simulink model "ACT_ur10"  (R2021b)
settings: Solver=ode4  StartTime=0.0  StopTime=15.0  FixedStep=1e-3  RelTol=1e-3
values from neighbouring files (symbols this model uses):
  Kp = [100 0 0 0 0 0 0 250 0 0 0 0 ... (36 elements, 6x6)]    [ACT_workspace.mat]    (also in GuadagniControllore.m = 100 * diag([1 1 2 4 5 5]))
  Kv = [100 0 0 0 0 0 0 100 0 0 0 0 ... (36 elements, 6x6)]    [ACT_workspace.mat]    (also in GuadagniControllore.m = 100 * diag([1 1 3 3 5 5]))
  l1 = 0.1273    [ACT_workspace.mat]
  l2 = -0.612    [ACT_workspace.mat]
  l3 = -0.5723    [ACT_workspace.mat]
  l4 = 0.1639    [ACT_workspace.mat]
  l5 = 0.1157    [ACT_workspace.mat]
  l6 = 0.0922    [ACT_workspace.mat]
  m1 = 7.1    [ACT_workspace.mat]
  m2 = 12.7    [ACT_workspace.mat]
  m3 = 4.27    [ACT_workspace.mat]
  m4 = 2    [ACT_workspace.mat]
  m5 = 2    [ACT_workspace.mat]
  m6 = 0.365    [ACT_workspace.mat]
  q0 = [0 0 0 0 0 0]    [ACT_workspace.mat]
  r = 0.02    [ACT_workspace.mat]
undefined symbols (not defined in the file or in its folder): B, pi_param, Spline
libraries: roblocks x2, robotcorelib x1, simulink x1
(part 2 of 6)

== matlab function ACT_ur10/CT control1/Dynamics_parametrs/Regressor ==
  data: q input; Y output; qd input; qdd input
function Y = Y(q, qd, qdd)

t1 = q(1);
t2 = q(2);
t3 = q(3);
t4 = q(4);
t5 = q(5);
t6 = q(6);
t1d = qd(1);
t2d = qd(2);
t3d = qd(3);
t4d = qd(4);
t5d = qd(5);
t6d = qd(6);
t1dd = qdd(1);
t2dd = qdd(2);
t3dd = qdd(3);
t4dd = qdd(4);
t5dd = qdd(5);
t6dd = qdd(6);




%#codegen

%    This function was generated by the Symbolic Math Toolbox version 9.0.
%    31-Aug-2022 14:42:02

t8 = cos(t1);
t9 = cos(t2);
t10 = cos(t3);
t11 = cos(t4);
t12 = cos(t5);
t13 = cos(t6);
t14 = sin(t1);
t15 = sin(t2);
t16 = sin(t3);
t17 = sin(t4);
t18 = sin(t5);
t19 = sin(t6);
t20 = t2+t3;
t21 = t1d.^2;
t22 = t2d.^2;
t33 = -t5;
t23 = t8.^2;
t24 = t9.^2;
t25 = t12.^2;
t26 = t14.^2;
t27 = t15.^2;
t28 = t18.^2;
t29 = t18.^3;
t30 = cos(t20);
t31 = sin(t20);
t32 = t4+t20;
t34 = t8.*t12;
t35 = t8.*t18;
t36 = t12.*t14;
t38 = t14.*t18;
t43 = t9.*t15.*t1d;
t45 = t9.*6.12e+3;
t46 = t15.*6.12e+3;
t86 = t9.*(1.53e+2./2.5e+2);
t87 = t8.*(1.53e+2./5.0e+2);
t96 = t15.*(1.53e+2./2.5e+2);
t97 = t14.*(1.53e+2./5.0e+2);
t160 = t8.*t9.*(-1.53e+2./2.5e+2);
t161 = t9.*t14.*(-1.53e+2./2.5e+2);
t167 = t14.*t15.*(-1.53e+2./2.5e+2);
t169 = t8.*1.639e-1;
t170 = t8.*2.8615e-1;
t171 = t14.*1.639e-1;
t172 = t14.*2.8615e-1;
t225 = t9.*6.00372;
t273 = t8.*t15.*t16.*5.723e-1;
t274 = t9.*t14.*t16.*5.723e-1;
t275 = t10.*t14.*t15.*5.723e-1;
t277 = t14.*t15.*t16.*5.723e-1;
t305 = t8.*t9.*t10.*5.723e-1;
t311 = t8.*t9.*t16.*5.723e-1;
t312 = t8.*t10.*t15.*5.723e-1;
t313 = t9.*t10.*t14.*5.723e-1;
t37 = cos(t32);
t39 = sin(t32);
t40 = t5+t32;
t41 = t30.^2;
t42 = t31.^2;
t47 = t8.*t24;
t48 = t9.*t23;
t49 = t8.*t27;
t50 = t9.*t26;
t51 = t15.*t23;
t52 = t14.*t24;
t54 = t14.*t27;
t55 = t15.*t26;
t58 = t43.*t2d.*2.0;
t65 = t32+t33;
t67 = t30.*5.723e+3;
t68 = t31.*5.723e+3;
t69 = t23.*t30;
t71 = t26.*t30;
t72 = t23.*t31;
t76 = t26.*t31;
t82 = t23+t26;
t88 = t30.*t31.*t1d;
t116 = t30.*t31.*t2d.*2.0;
t117 = t30.*t31.*t3d.*2.0;
t124 = t8.*t86;
t126 = t8.*t96;
t127 = t14.*t86;
t134 = t14.*t96;
t208 = t17.*t31.*9.22e-2;
t209 = t30.*5.723e-1;
t212 = t34.*1.383e-1;
t213 = t34.*5.785e-2;
t214 = t31.*5.723e-1;
t216 = t35.*1.383e-1;
t217 = t36.*1.383e-1;
t218 = t35.*5.785e-2;
t219 = t36.*5.785e-2;
t222 = t38.*1.383e-1;
t223 = t38.*5.785e-2;
t236 = t11.*t30.*9.22e-2;
t238 = t17.*t30.*9.22e-2;
t239 = t11.*t31.*9.22e-2;
t244 = -t225;
t271 = t17.*t31.*1.157e-1;
t302 = t11.*t30.*1.157e-1;
t306 = t17.*t30.*1.157e-1;
t307 = t11.*t31.*1.157e-1;
t315 = t14.*t31.*(-5.723e-1);
t316 = -t277;
t335 = -t305;
t338 = t8.*t31.*(-5.723e-1);
t366 = t30.*5.614263;
t396 = t14.*t17.*t30.*(-1.157e-1);
t397 = t8.*t17.*t31.*(-1.157e-1);
t398 = t11.*t14.*t31.*(-1.157e-1);
t399 = t14.*t17.*t31.*(-1.157e-1);
t486 = t87+t161;
t44 = sin(t40);
t53 = t37.^2;
t56 = t39.^2;
t57 = t39.^3;
t59 = t13.*t37;
t60 = t19.*t37;
t61 = t13.*t39;
t62 = t41.*2.0;
t63 = t19.*t39;
t64 = t42.*2.0;
t66 = sin(t65);
t70 = t8.*t41;
t73 = t14.*t41;
t74 = t8.*t42;
t77 = t14.*t42;
t78 = -t42;
t80 = -t49;
t81 = -t54;
t83 = t34.*t37;
t89 = t35.*t37;
t90 = t36.*t37;
t98 = t37.*t38;
t104 = t23.*t37;
t107 = t26.*t37;
t108 = t23.*t39;
t113 = t26.*t39;
t128 = t37.*t39.*t1d;
t141 = t69./2.0;
t145 = t71./2.0;
t146 = t72./2.0;
t147 = t76./2.0;
t152 = t37.*t39.*2.0;
t173 = t12.*t37.*t39;
t174 = t18.*t37.*t39;
t197 = t23.*t82;
t198 = t26.*t82;
t204 = t30.*t82;
t205 = t31.*t82;
t226 = t48+t50;
t227 = t37.*t82;
t229 = t51+t55;
t230 = t39.*t82;
t241 = -t209;
t251 = t37.*1.157e-1;
t252 = t37.*8.195e-2;
t253 = t39.*1.157e-1;
t254 = t39.*8.195e-2;
t259 = -t236;
t272 = t14.*t214;
t285 = t18.*t37.*4.61e-2;
t286 = t12.*t39.*4.61e-2;
t294 = t18.*t39.*4.61e-2;
t298 = t45+t67;
t299 = t46+t68;
t308 = t8.*t214;
t314 = -t271;
t324 = t18.*t37.*5.785e-2;
t327 = t18.*t39.*5.785e-2;
t336 = -t306;
t337 = -t307;
t343 = t72+t76;
t346 = t72.*5.723e-1;
t347 = t76.*5.723e-1;
t349 = t14.*t39.*(-8.195e-2);
t350 = t8.*t302;
t351 = t8.*t306;
t352 = t14.*t302;
t353 = t8.*t307;
t357 = t14.*t306;
t358 = t8.*t271;
t359 = t14.*t307;
t362 = t14.*t271;
t365 = t69+t71;
t380 = t39.*t216;
t382 = t39.*t218;
t388 = t39.*t222;
t389 = t39.*t223;
t404 = -t366;
t419 = t39.*1.135017;
t420 = t39.*8.039295e-1;
t454 = t97+t124;
t460 = t116+t117;
t529 = t86+t209;
t530 = t96+t214;
t554 = t14.*t486;
t622 = t238+t239;
t707 = t9.*t87.*t486;
t708 = t126.*t486;
t75 = t53.*t1dd;
t79 = -t64;
t84 = t8.*t59;
t85 = t12.*t59;
t91 = t8.*t60;
t92 = t14.*t59;
t93 = t8.*t61;
t94 = t12.*t60;
t95 = t12.*t61;
t99 = t14.*t60;
t100 = t8.*t63;
t101 = t14.*t61;
t102 = t12.*t63;
t103 = t14.*t63;
t105 = t8.*t53;
t106 = t12.*t53;
t109 = t14.*t53;
t110 = t8.*t56;
t111 = t18.*t53;
t112 = t12.*t56;
t114 = t14.*t56;
t115 = t18.*t56;
t118 = -t74;
t119 = -t77;
t125 = t34.*t61;
t129 = t34.*t63;
t130 = t36.*t61;
t131 = t23.*t56;
t132 = t25.*t57;
t135 = t36.*t63;
t136 = t26.*t56;
t137 = t28.*t56;
t138 = t28.*t57;
t139 = -t89;
t140 = -t90;
t148 = t34.*t56;
t149 = t35.*t56;
t150 = t36.*t56;
t151 = t12.*t18.*t57;
t153 = t38.*t56;
t163 = t152.*t2d;
t164 = t152.*t3d;
t165 = t152.*t4d;
t166 = t25.*t56.*2.0;
t178 = -t152;
t179 = t104./2.0;
t180 = t107./2.0;
t181 = t108./2.0;
t182 = t113./2.0;
t188 = t39.*t53.*3.0;
t228 = t204.*t1dd;
t231 = t205.*t1dd;
t232 = t18.*t39.*t59;
t233 = t18.*t39.*t60;
t242 = t39.*t53.*(3.0./2.0);
t245 = t25.*t128;
t246 = t39.*t83.*3.0;
t247 = t28.*t128;
t248 = t39.*t89.*3.0;
t249 = t39.*t90.*3.0;
t250 = t39.*t98.*3.0;
t255 = t34+t98;
t256 = t38+t83;
t257 = t227.*t1dd;
t258 = t230.*t1dd;
t260 = t41+t78;
t261 = t39.*t104.*2.0;
t264 = -t204;
t265 = t39.*t107.*2.0;
t266 = t28.*t152;
t269 = -t205;
t278 = t53.*t108;
t279 = t25.*t39.*t53;
t280 = t47+t80;
t281 = t53.*t113;
t283 = t28.*t39.*t53;
t284 = -t227;
t290 = t52+t81;
t291 = -t230;
t295 = -t251;
t296 = -t253;
t297 = -t254;
t301 = t12.*t18.*t128.*2.0;
t321 = t29.*t37.*t56.*3.0;
t322 = t8.*t252;
t323 = -t285;
t325 = t14.*t252;
t326 = t8.*t254;
t328 = t14.*t254;
t348 = -t324;
t355 = (t204.*t1d.*t2d)./2.0;
t356 = (t204.*t1d.*t3d)./2.0;
t360 = (t205.*t1d.*t2d)./2.0;
t361 = (t205.*t1d.*t3d)./2.0;
t369 = t83.*1.383e-1;
t370 = t83.*5.785e-2;
t371 = t89.*1.383e-1;
t372 = t90.*1.383e-1;
t373 = t89.*5.785e-2;
t374 = t90.*5.785e-2;
t376 = (t227.*t1d.*t2d)./2.0;
t377 = (t227.*t1d.*t3d)./2.0;
t378 = (t227.*t1d.*t4d)./2.0;
t379 = t98.*1.383e-1;
t381 = t98.*5.785e-2;
t384 = t29.*t37.*t56.*(3.0./2.0);
t385 = (t230.*t1d.*t2d)./2.0;
t386 = (t230.*t1d.*t3d)./2.0;
t387 = (t230.*t1d.*t4d)./2.0;
t392 = t104.*8.195e-2;
t393 = t107.*8.195e-2;
t421 = t365.*t2d;
t422 = t365.*t3d;
t425 = t104+t107;
t426 = t343.*t2d;
t427 = t343.*t3d;
t431 = t108+t113;
t432 = t44.*6.783615e-1;
t433 = t44.*2.8375425e-1;
t492 = t66.*6.783615e-1;
t493 = t66.*2.8375425e-1;
t497 = t460.*t1d;
t532 = t8.*t454;
t534 = (t14.*t299)./1.0e+4;
t550 = (t8.*t298)./1.0e+4;
t551 = (t14.*t298)./1.0e+4;
t553 = (t8.*t299)./1.0e+4;
t562 = t530.^2;
t583 = t197+t198;
t584 = (t23.*t299)./1.0e+4;
t586 = (t26.*t299)./1.0e+4;
t599 = -t554;
t638 = t208+t259;
t647 = t214+t252;
t648 = t39.*t104.*3.35790125e-3;
t649 = t39.*t104.*1.007370375e-2;
t652 = t39.*t107.*3.35790125e-3;
t653 = t39.*t107.*1.007370375e-2;
t670 = t241+t254;
t677 = t12.*t622;
t678 = t18.*t622;
t687 = t251+t327;
t692 = t9.*t97.*t454;
t693 = t134.*t454;
t742 = t346+t347;
t820 = t252+t530;
t896 = t69.*t530.*2.8615e-1;
t897 = t76.*t529.*2.8615e-1;
t899 = t346.*t530;
t900 = t71.*t530.*2.8615e-1;
t907 = t347.*t530;
t932 = t72.*t529.*2.8615e-1;
t1287 = t350+t380+t397;
t1288 = t350+t382+t397;
t1297 = t352+t388+t399;
t1298 = t352+t389+t399;
t1453 = t169+t313+t316+t349;
t120 = t106.*2.0;
t121 = t111.*2.0;
t122 = t112.*2.0;
t123 = t115.*2.0;
t133 = -t85;
t142 = -t100;
t143 = -t101;
t144 = -t102;
t154 = -t110;
t155 = -t112;
t157 = -t114;
t158 = -t115;
t162 = t18.*t112.*t1d;
t168 = t137.*2.0;
t175 = t137.*t1dd;
t177 = t151.*2.0;
t183 = t28.*t110;
t184 = t26.*t112;
t185 = t23.*t115;
t186 = t25.*t114;
t187 = t13.*t137;
t189 = t28.*t114;
t190 = t26.*t115;
t191 = t19.*t137;
t193 = -t129;
t194 = -t135;
t196 = -t138;
t199 = -t148;
t200 = t18.*t112.*-2.0;
t201 = -t151;
t203 = -t153;
t206 = t25.*t110;
t207 = t23.*t112;
t211 = -t188;
t221 = t132./2.0;
t224 = t138./2.0;
t237 = t37.*t112;
t240 = t37.*t115;
t276 = -t242;
t282 = t37.*t137;
t287 = t28.*t163;
t288 = t28.*t164;
t289 = t28.*t165;
t292 = -t248;
t293 = -t249;
t317 = t255.^2;
t318 = t62+t79;
t319 = t279.*2.0;
t320 = t283.*2.0;
t329 = t35+t140;
t330 = t36+t139;
t333 = t18.*t39.*t106.*4.0;
t334 = -t257;
t339 = t14.*t256;
t340 = t19.*t256;
t341 = t60+t95;
t342 = t61+t94;
t344 = -t279;
t363 = t8.*t255;
t364 = t13.*t256;
t367 = t21.*t260;
t375 = t53.*t181;
t383 = t53.*t182;
t390 = t14.*t280;
t391 = t8.*t290;
t394 = -t355;
t395 = -t356;
t405 = t73+t119;
t406 = -t371;
t407 = -t372;
t408 = -t373;
t409 = -t374;
t410 = -t376;
t411 = -t377;
t412 = -t378;
t414 = -t385;
t415 = -t386;
t416 = -t387;
t430 = t70+t118;
t435 = t37.*t255;
t436 = t37.*t256;
t437 = t39.*t255;
t438 = t39.*t256;
t439 = t148.*5.785e-2;
t441 = t150.*5.785e-2;
t442 = -t432;
t443 = -t433;
t450 = t425.*t2d;
t451 = t425.*t3d;
t452 = t425.*t4d;
t453 = t91+t125;
t456 = t431.*t2d;
t457 = t431.*t3d;
t458 = t431.*t4d;
t459 = t99+t130;
t505 = t101.*t255;
t512 = t103.*t255;
t535 = t18.*t61.*t255.*2.0;
t537 = t18.*t63.*t255.*2.0;
t555 = -t534;
t568 = t153.*t255;
t571 = -t551;
t572 = -t553;
t617 = t583.*t2dd;
t618 = t583.*t3dd;
t619 = t583.*t4dd;
t637 = t53+t131+t136;
t675 = t647.^2;
t688 = t18.*t638;
t697 = t255.*t380;
t703 = t253+t348;
t704 = t212+t379;
t705 = t222+t369;
t706 = t223+t370;
t720 = t687.^2;
t777 = t163+t164+t165;
t787 = t146+t147+t269;
t793 = t172+t550;
t795 = t167+t534;
t798 = t141+t145+t264;
t799 = t392+t393;
t842 = t426+t427;
t843 = t297+t529;
t855 = t8.*t37.*t687;
t858 = t14.*t37.*t687;
t859 = t8.*t39.*t687;
t860 = t14.*t39.*t687;
t865 = t421+t422;
t876 = t179+t180+t284;
t878 = t181+t182+t291;
t880 = t820.^2;
t881 = -t8.*(t553-t8.*t15.*(1.53e+2./2.5e+2));
t951 = t178+t261+t265;
t1036 = t214+t687;
t1055 = t209+t296+t324;
t1082 = t286+t677;
t1089 = t392.*t647;
t1092 = t393.*t647;
t1093 = t108.*t647.*8.195e-2;
t1094 = t108.*t647.*4.0975e-2;
t1097 = t113.*t647.*8.195e-2;
t1098 = t113.*t647.*4.0975e-2;
t1121 = t311+t312+t322;
t1122 = t392.*t670;
Y = ft_1({t100,t101,t103,t1036,t104,t105,t1055,t106,t107,t108,t1082,t1089,t109,t1092,t1093,t1094,t1097,t1098,t111,t112,t1121,t1122,t113,t115,t12,t120,t121,t122,t123,t124,t126,t127,t128,t1287,t1288,t1297,t1298,t13,t131,t132,t133,t134,t136,t137,t138,t14,t140,t142,t143,t144,t1453,t148,t149,t15,t150,t152,t153,t154,t155,t157,t158,t160,t162,t163,t164,t165,t166,t168,t169,t170,t171,t172,t173,t174,t175,t177,t179,t18,t180,t183,t184,t185,t186,t187,t189,t19,t190,t191,t193,t194,t196,t199,t1d,t1dd,t200,t201,t203,t206,t207,t209,t21,t211,t213,t214,t216,t217,t218,t219,t22,t221,t224,t226,t228,t229,t23,t231,t232,t233,t237,t24,t240,t241,t244,t245,t246,t247,t248,t249,t25,t250,t255,t256,t258,t26,t261,t265,t266,t27,t272,t273,t274,t275,t276,t278,t279,t28,t281,t282,t283,t285,t287,t288,t289,t29,t292,t293,t294,t295,t296,t299,t2d,t2dd,t30,t301,t302,t306,t307,t308,t31,t311,t312,t313,t314,t315,t316,t317,t318,t319,t320,t321,t322,t323,t324,t325,t326,t328,t329,t330,t333,t334,t335,t336,t337,t338,t339,t34,t340,t341,t342,t343,t344,t346,t347,t35,t351,t353,t36,t360,t361,t363,t364,t365,t367,t37,t375,t38,t381,t383,t384,t388,t39,t390,t391,t392,t393,t394,t395,t396,t398,t3d,t3dd,t404,t405,t406,t407,t408,t409,t41,t410,t411,t412,t414,t415,t416,t419,t42,t420,t425,t43,t430,t431,t435,t436,t437,t438,t439,t441,t442,t443,t450,t451,t452,t453,t454,t456,t457,t458,t459,t48,t486,t492,t493,t497,t4d,t4dd,t50,t51,t512,t529,t53,t530,t532,t535,t537,t55,t550,t553,t554,t555,t56,t562,t57,t571,t572,t58,t584,t586,t59,t599,t5d,t5dd,t61,t617,t618,t619,t63,t637,t647,t648,t649,t652,t653,t670,t675,t678,t687,t688,t69,t692,t693,t697,t6d,t6dd,t703,t704,t705,t706,t707,t708,t71,t720,t742,t75,t777,t787,t793,t795,t798,t799,t8,t82,t820,t83,t84,t842,t843,t855,t858,t859,t860,t865,t876,t878,t88,t880,t881,t89,t896,t897,t899,t9,t90,t900,t907,t92,t93,t932,t951,t98});
end
function Y = ft_1(ct)
t100 = ct{1};
t101 = ct{2};
t103 = ct{3};
t1036 = ct{4};
t104 = ct{5};
t105 = ct{6};
t1055 = ct{7};
t106 = ct{8};
t107 = ct{9};
t108 = ct{10};
t1082 = ct{11};
t1089 = ct{12};
t109 = ct{13};
t1092 = ct{14};
t1093 = ct{15};
t1094 = ct{16};
t1097 = ct{17};
t1098 = ct{18};
t111 = ct{19};
t112 = ct{20};
t1121 = ct{21};
t1122 = ct{22};
t113 = ct{23};
t115 = ct{24};
t12 = ct{25};
t120 = ct{26};
t121 = ct{27};
t122 = ct{28};
t123 = ct{29};
t124 = ct{30};
t126 = ct{31};
t127 = ct{32};
t128 = ct{33};
t1287 = ct{34};
t1288 = ct{35};
t1297 = ct{36};
t1298 = ct{37};
t13 = ct{38};
t131 = ct{39};
t132 = ct{40};
t133 = ct{41};
t134 = ct{42};
t136 = ct{43};
t137 = ct{44};
t138 = ct{45};
t14 = ct{46};
t140 = ct{47};
t142 = ct{48};
t143 = ct{49};
t144 = ct{50};
t1453 = ct{51};
t148 = ct{52};
t149 = ct{53};
t15 = ct{54};
t150 = ct{55};
t152 = ct{56};
t153 = ct{57};
t154 = ct{58};
t155 = ct{59};
t157 = ct{60};
t158 = ct{61};
t160 = ct{62};
t162 = ct{63};
t163 = ct{64};
t164 = ct{65};
t165 = ct{66};
t166 = ct{67};
t168 = ct{68};
t169 = ct{69};
t170 = ct{70};
t171 = ct{71};
t172 = ct{72};
t173 = ct{73};
t174 = ct{74};
t175 = ct{75};
t177 = ct{76};
t179 = ct{77};
t18 = ct{78};
t180 = ct{79};
t183 = ct{80};
t184 = ct{81};
t185 = ct{82};
t186 = ct{83};
t187 = ct{84};
t189 = ct{85};
t19 = ct{86};
t190 = ct{87};
t191 = ct{88};
t193 = ct{89};
t194 = ct{90};
t196 = ct{91};
t199 = ct{92};
t1d = ct{93};
t1dd = ct{94};
t200 = ct{95};
t201 = ct{96};
t203 = ct{97};
t206 = ct{98};
t207 = ct{99};
t209 = ct{100};
t21 = ct{101};
t211 = ct{102};
t213 = ct{103};
t214 = ct{104};
t216 = ct{105};
t217 = ct{106};
t218 = ct{107};
t219 = ct{108};
t22 = ct{109};
t221 = ct{110};
t224 = ct{111};
t226 = ct{112};
t228 = ct{113};
t229 = ct{114};
t23 = ct{115};
t231 = ct{116};
t232 = ct{117};
t233 = ct{118};
t237 = ct{119};
t24 = ct{120};
t240 = ct{121};
t241 = ct{122};
t244 = ct{123};
t245 = ct{124};
t246 = ct{125};
t247 = ct{126};
t248 = ct{127};
t249 = ct{128};
t25 = ct{129};
t250 = ct{130};
t255 = ct{131};
t256 = ct{132};
t258 = ct{133};
t26 = ct{134};
t261 = ct{135};
t265 = ct{136};
t266 = ct{137};
t27 = ct{138};
t272 = ct{139};
t273 = ct{140};
t274 = ct{141};
t275 = ct{142};
t276 = ct{143};
t278 = ct{144};
t279 = ct{145};
t28 = ct{146};
t281 = ct{147};
t282 = ct{148};
t283 = ct{149};
t285 = ct{150};
t287 = ct{151};
t288 = ct{152};
t289 = ct{153};
t29 = ct{154};
t292 = ct{155};
t293 = ct{156};
t294 = ct{157};
t295 = ct{158};
t296 = ct{159};
t299 = ct{160};
t2d = ct{161};
t2dd = ct{162};
t30 = ct{163};
t301 = ct{164};
t302 = ct{165};
t306 = ct{166};
t307 = ct{167};
t308 = ct{168};
t31 = ct{169};
t311 = ct{170};
t312 = ct{171};
t313 = ct{172};
t314 = ct{173};
t315 = ct{174};
t316 = ct{175};
t317 = ct{176};
t318 = ct{177};
t319 = ct{178};
t320 = ct{179};
t321 = ct{180};
t322 = ct{181};
t323 = ct{182};
t324 = ct{183};
t325 = ct{184};
t326 = ct{185};
t328 = ct{186};
t329 = ct{187};
t330 = ct{188};
t333 = ct{189};
t334 = ct{190};
t335 = ct{191};
t336 = ct{192};
t337 = ct{193};
t338 = ct{194};
t339 = ct{195};
t34 = ct{196};
t340 = ct{197};
t341 = ct{198};
t342 = ct{199};
t343 = ct{200};
t344 = ct{201};
t346 = ct{202};
t347 = ct{203};
t35 = ct{204};
t351 = ct{205};
t353 = ct{206};
t36 = ct{207};
t360 = ct{208};
t361 = ct{209};
t363 = ct{210};
t364 = ct{211};
t365 = ct{212};
t367 = ct{213};
t37 = ct{214};
t375 = ct{215};
t38 = ct{216};
t381 = ct{217};
t383 = ct{218};
t384 = ct{219};
t388 = ct{220};
t39 = ct{221};
t390 = ct{222};
t391 = ct{223};
t392 = ct{224};
t393 = ct{225};
t394 = ct{226};
t395 = ct{227};
t396 = ct{228};
t398 = ct{229};
t3d = ct{230};
t3dd = ct{231};
t404 = ct{232};
t405 = ct{233};
t406 = ct{234};
t407 = ct{235};
t408 = ct{236};
t409 = ct{237};
t41 = ct{238};
t410 = ct{239};
t411 = ct{240};
t412 = ct{241};
t414 = ct{242};
t415 = ct{243};
t416 = ct{244};
t419 = ct{245};
t42 = ct{246};
t420 = ct{247};
t425 = ct{248};
t43 = ct{249};
t430 = ct{250};
t431 = ct{251};
t435 = ct{252};
t436 = ct{253};
t437 = ct{254};
t438 = ct{255};
t439 = ct{256};
t441 = ct{257};
t442 = ct{258};
t443 = ct{259};
t450 = ct{260};
t451 = ct{261};
t452 = ct{262};
t453 = ct{263};
t454 = ct{264};
t456 = ct{265};
t457 = ct{266};
t458 = ct{267};
t459 = ct{268};
t48 = ct{269};
t486 = ct{270};
t492 = ct{271};
t493 = ct{272};
t497 = ct{273};
t4d = ct{274};
t4dd = ct{275};
t50 = ct{276};
t51 = ct{277};
t512 = ct{278};
t529 = ct{279};
t53 = ct{280};
t530 = ct{281};
t532 = ct{282};
t535 = ct{283};
t537 = ct{284};
t55 = ct{285};
t550 = ct{286};
t553 = ct{287};
t554 = ct{288};
t555 = ct{289};
t56 = ct{290};
t562 = ct{291};
t57 = ct{292};
t571 = ct{293};
t572 = ct{294};
t58 = ct{295};
t584 = ct{296};
t586 = ct{297};
t59 = ct{298};
t599 = ct{299};
t5d = ct{300};
t5dd = ct{301};
t61 = ct{302};
t617 = ct{303};
t618 = ct{304};
t619 = ct{305};
t63 = ct{306};
t637 = ct{307};
t647 = ct{308};
t648 = ct{309};
t649 = ct{310};
t652 = ct{311};
t653 = ct{312};
t670 = ct{313};
t675 = ct{314};
t678 = ct{315};
t687 = ct{316};
t688 = ct{317};
t69 = ct{318};
t692 = ct{319};
t693 = ct{320};
t697 = ct{321};
t6d = ct{322};
t6dd = ct{323};
t703 = ct{324};
t704 = ct{325};
t705 = ct{326};
t706 = ct{327};
t707 = ct{328};
t708 = ct{329};
t71 = ct{330};
t720 = ct{331};
t742 = ct{332};
t75 = ct{333};
t777 = ct{334};
t787 = ct{335};
t793 = ct{336};
t795 = ct{337};
t798 = ct{338};
t799 = ct{339};
t8 = ct{340};
t82 = ct{341};
t820 = ct{342};
t83 = ct{343};
t84 = ct{344};
t842 = ct{345};
t843 = ct{346};
t855 = ct{347};
t858 = ct{348};
t859 = ct{349};
t860 = ct{350};
t865 = ct{351};
t876 = ct{352};
t878 = ct{353};
t88 = ct{354};
t880 = ct{355};
t881 = ct{356};
t89 = ct{357};
t896 = ct{358};
t897 = ct{359};
t899 = ct{360};
t9 = ct{361};
t90 = ct{362};
t900 = ct{363};
t907 = ct{364};
t92 = ct{365};
t93 = ct{366};
t932 = ct{367};
t951 = ct{368};
t98 = ct{369};
t1123 = t104.*t670.*4.0975e-2;
t1133 = t393.*t670;
t1134 = t107.*t670.*4.0975e-2;
t1140 = t274+t275+t325;
t1203 = t532+t599;
t1222 = t12.*t113.*t687.*2.8925e-2;
t1245 = t12.*t108.*t687.*5.785e-2;
t1246 = t12.*t108.*t687.*2.8925e-2;
t1248 = t12.*t113.*t687.*5.785e-2;
t1265 = t584+t586;
t1302 = t530+t687;
t1321 = t296+t324+t529;
t1330 = t393.*t820;
t1331 = t108.*t820.*8.195e-2;
t1332 = t108.*t820.*4.0975e-2;
t1334 = t113.*t820.*8.195e-2;
t1335 = t113.*t820.*4.0975e-2;
t1352 = t392.*t820;
t1364 = t8.*t1287;
t1365 = t8.*t1288;
t1372 = t14.*t1297;
t1373 = t14.*t1298;
t1426 = t37.*t1287;
t1427 = t37.*t1288;
t1431 = t37.*t1297;
t1432 = t37.*t1298;
t1450 = t171+t273+t326+t335;
t1462 = t14.*t39.*t1287;
t1463 = t14.*t39.*t1288;
t1466 = t8.*t39.*t1297;
t1467 = t8.*t39.*t1298;
t1510 = t14.*t1453;
t1519 = t693+t708;
t1534 = t692+t707;
t1596 = t213+t381+t396+t398;
t1666 = t23.*t647.*t820;
t1669 = t26.*t647.*t820;
t1677 = t127+t1453;
t1754 = (t23.*t670.*t820)./2.0;
t1758 = (t26.*t670.*t820)./2.0;
t1807 = t294+t302+t314+t678;
t1961 = t311+t312+t1287;
t1962 = t311+t312+t1288;
t1976 = t274+t275+t1297;
t1977 = t274+t275+t1298;
t2106 = (t14.*t687.*t1288)./2.0;
t2109 = (t8.*t687.*t1298)./2.0;
t156 = -t122;
t159 = -t123;
t176 = t18.*t122;
t195 = -t168;
t202 = -t177;
t210 = t13.*t168;
t215 = t19.*t168;
t220 = t18.*t155.*t1d;
t234 = t34.*t123;
t235 = t36.*t123;
t243 = -t224;
t262 = t37.*t122;
t263 = t39.*t120;
t267 = t37.*t123;
t268 = t39.*t121;
t270 = t25.*t154;
t300 = t18.*t237;
t303 = t37.*t155;
t304 = t237.*-2.0;
t309 = t37.*t158;
t310 = t240.*-2.0;
t345 = -t319;
t368 = t330.^2;
t400 = t14.*t330;
t401 = t19.*t329;
t402 = t59+t144;
t403 = t63+t133;
t413 = t13.*t317;
t417 = t19.*t317;
t418 = t341.^2;
t423 = t13.*t363;
t424 = t19.*t363;
t428 = t8.*t329;
t429 = t13.*t329;
t434 = -t367;
t440 = -t391;
t447 = t390./2.0;
t448 = t391./2.0;
t449 = -t441;
t462 = t105+t154;
t463 = t106+t155;
t465 = t109+t157;
t466 = t111+t158;
t467 = t183.*1.383e-1;
t468 = t8.*t436;
t469 = t12.*t435;
t470 = t12.*t436;
t471 = t189.*1.383e-1;
t472 = t14.*t435;
t473 = t8.*t438;
t474 = t18.*t435;
t475 = t18.*t436;
t476 = t12.*t437;
t477 = t14.*t437;
t478 = t18.*t438;
t479 = t14.*t430;
t480 = t37.*t329;
t481 = t37.*t330;
t482 = t8.*t405;
t483 = t39.*t329;
t484 = t39.*t330;
t490 = t12.*t438.*2.0;
t491 = t18.*t437.*2.0;
t494 = t37.*t341;
t495 = t37.*t342;
t496 = t39.*t341;
t499 = t84+t193;
t502 = t92+t194;
t503 = t35.*t437;
t504 = t36.*t438;
t506 = t8.*t459;
t533 = t14.*t453;
t536 = t38.*t437.*2.0;
t545 = t18.*t39.*t342;
t556 = t100.*t330;
t557 = t143.*t255;
t561 = -t512;
t574 = t93.*t330;
t578 = t18.*t61.*t330.*2.0;
t579 = t18.*t63.*t330.*2.0;
t597 = t115.*t341;
t602 = t18.*t63.*t341.*2.0;
t603 = t149.*t330;
t606 = t203.*t255;
t609 = t93+t340;
t610 = t189.*t255;
t611 = t123.*t341;
t614 = t83.*t438;
t615 = t8.*t39.*t453;
t616 = t18.*t39.*t453;
t620 = t98.*t437;
t623 = t14.*t39.*t459;
t624 = t18.*t39.*t459;
t634 = t158.*t341;
t636 = t168.*t341;
t640 = t142+t364;
t642 = t183.*t330;
t644 = t28.*t157.*t255;
t664 = t18.*t152.*t341;
t695 = -t14.*(t100-t364);
t696 = t266.*t341;
t698 = t255.*t341;
t699 = t256.*t341;
t700 = t255.*t342;
t709 = t255.*t329.*2.0;
t710 = t256.*t330.*2.0;
t715 = t199+t436;
t718 = t203+t435;
t719 = -t688;
t721 = t216+t407;
t722 = t217+t406;
t723 = t218+t409;
t731 = t330.*t388;
t732 = t329.*t341;
t733 = t330.*t341;
t734 = t330.*t342;
t738 = t39.*t637;
t741 = t246+t438;
t743 = t250+t437;
t744 = t341.*t342;
t745 = t8.*t705;
t746 = t8.*t706;
t749 = -t8.*t39.*(t100-t364);
t750 = -t18.*t37.*(t100-t364);
t751 = -t12.*t39.*(t100-t364);
t758 = -t18.*t39.*(t100-t364);
t768 = -t14.*(t148-t436);
t769 = -t8.*(t153-t435);
t771 = t8.*t37.*t637;
t772 = t12.*t37.*t637;
t773 = t14.*t37.*t637;
t774 = t18.*t37.*t637;
t779 = t255.*t459;
t782 = -t8.*t37.*(t100-t364);
t791 = t126+t572;
t802 = t8.*t39.*(t100-t364);
t811 = t18.*t39.*(t100-t364);
t818 = t37.*t705;
t819 = t37.*t706;
t824 = t170+t571;
t828 = t777.*t1d;
t830 = t330.*t453;
t836 = -t35.*t39.*(t100-t364);
t837 = -t18.*t61.*(t100-t364);
t840 = -t18.*t63.*(t100-t364);
t841 = t341.*t453;
t844 = t341.*t459;
t849 = t14.*(t148-t436).*(-1.0./2.0);
t850 = t8.*(t153-t435).*(-1.0./2.0);
t856 = t798.*t2d;
t857 = t798.*t3d;
t862 = t787.*t2d;
t863 = t787.*t3d;
t869 = t18.*t37.*t704;
t870 = t12.*t39.*t704;
t872 = t14.*t39.*t705;
t873 = t18.*t39.*t704;
t874 = t18.*t39.*t705;
t875 = t14.*t39.*t706;
t884 = t8.*t793;
t885 = t8.*t39.*t703;
t886 = t14.*t39.*t703;
t890 = t14.*t795;
t892 = t35.*t39.*(t100-t364);
t893 = t18.*t61.*(t100-t364);
t918 = -t8.*t37.*(t148-t436);
t920 = -t8.*t39.*(t148-t436);
t921 = -t855;
t924 = -t858;
t925 = -t859;
t926 = -t14.*t37.*(t153-t435);
t929 = -t14.*t39.*(t153-t435);
t933 = t35.*t39.*t704;
t934 = t876.*t2d;
t935 = t876.*t3d;
t936 = t876.*t4d;
t940 = t878.*t2d;
t941 = t878.*t3d;
t942 = t878.*t4d;
t963 = t8.*t37.*(t148-t436);
t966 = t8.*t39.*(t148-t436);
t970 = t14.*t37.*(t153-t435);
t973 = t14.*t39.*(t153-t435);
t1002 = t255.*t637;
t1003 = t256.*t637;
t1016 = -t256.*(t100-t364);
t1051 = t329.*t637;
t1052 = t330.*t637;
t1065 = -t330.*(t100-t364);
t1066 = t256.*(t100-t364);
t1075 = -t342.*(t100-t364);
t1085 = t37.*t951;
t1096 = t1036.^2;
t1104 = t341.*(t100-t364).*-2.0;
t1135 = -t1094;
t1139 = -t1098;
t1141 = t255.*t705;
t1142 = t256.*t704;
t1163 = t8.*t39.*t951;
t1164 = t12.*t39.*t951;
t1165 = t14.*t39.*t951;
t1166 = t18.*t39.*t951;
t1169 = t160+t793;
t1172 = -t1123;
t1174 = -t1134;
t1194 = t330.*t704;
t1200 = t14.*t1140;
t1215 = t8.*t1121;
t1256 = t14.*t209.*t793;
t1257 = t30.*t172.*t793;
t1258 = t272.*t793;
t1299 = t8.*t39.*t1082;
t1303 = t14.*t39.*t1082;
t1333 = t1302.^2;
t1355 = -t1332;
t1358 = -t1335;
t1368 = t617+t618;
t1375 = t104.*t843.*4.0975e-2;
t1378 = t107.*t843.*4.0975e-2;
t1380 = t255.*t951;
t1381 = t256.*t951;
t1410 = t126+t1121;
t1413 = t134+t1140;
t1414 = t329.*t951;
t1415 = t330.*t951;
t1470 = t255.*t1082;
t1481 = t8.*t1450;
t1485 = t450+t451+t452;
t1488 = t14.*t530.*t793;
t1492 = t456+t457+t458;
t1494 = -t1466;
t1495 = -t1467;
t1498 = t325.*t1121;
t1499 = t14.*t37.*t1121.*4.0975e-2;
t1500 = t322.*t1140;
t1501 = t8.*t37.*t1140.*4.0975e-2;
t1506 = t330.*t1082;
t1512 = t338+t1121;
t1515 = t315+t1140;
t1516 = t14.*t37.*t1121.*(-8.195e-2);
t1517 = t12.*t108.*t1036.*5.785e-2;
t1518 = t12.*t108.*t1036.*2.8925e-2;
t1520 = t12.*t113.*t1036.*5.785e-2;
t1521 = t12.*t113.*t1036.*2.8925e-2;
t1540 = -t1510;
t1541 = (t14.*t529.*t793)./2.0;
t1547 = t14.*t687.*t706;
t1576 = t219+t351+t353+t408;
t1595 = t396+t398+t704;
t1650 = (t23.*t687.*t703)./2.0;
t1651 = t23.*t687.*t703.*(3.0./2.0);
t1652 = (t26.*t687.*t703)./2.0;
t1653 = t26.*t687.*t703.*(3.0./2.0);
t1674 = t160+t1450;
t1709 = t12.*t108.*t1302.*5.785e-2;
t1710 = t12.*t108.*t1302.*2.8925e-2;
t1713 = t12.*t113.*t1302.*5.785e-2;
t1714 = t12.*t113.*t1302.*2.8925e-2;
t1729 = t37.*t1596;
t1731 = t39.*t1596;
t1745 = t14.*t1677;
t1751 = (t23.*t647.*t843)./2.0;
t1755 = (t26.*t647.*t843)./2.0;
t1818 = t306+t307+t323+t688;
t1837 = t14.*t706.*t1036;
t1840 = t1807.^2;
t1863 = t23.*t687.*t1036;
t1868 = t26.*t687.*t1036;
t1888 = t23.*t687.*t1055;
t1889 = t23.*t703.*t1036;
t1890 = t26.*t687.*t1055;
t1891 = t26.*t703.*t1036;
t1906 = (t14.*t647.*t1121)./2.0;
t1910 = (t8.*t647.*t1140)./2.0;
t2003 = t8.*t37.*t1807;
t2006 = t14.*t37.*t1807;
t2007 = t8.*t39.*t1807;
t2008 = t14.*t39.*t1807;
t2034 = t8.*t1961;
t2035 = t8.*t1962;
t2040 = t14.*t1976;
t2041 = t14.*t1977;
t2043 = t14.*t820.*t1121;
t2044 = t8.*t820.*t1140;
t2051 = t322.*t1677;
t2055 = t326.*t1677;
t2056 = t8.*t39.*t1677.*4.0975e-2;
t2070 = t14.*t706.*t1302;
t2081 = t23.*t687.*t1302;
t2087 = t26.*t687.*t1302;
t2100 = t23.*t703.*t1302;
t2101 = t26.*t703.*t1302;
t2113 = t214+t1807;
t2118 = -t2106;
t2141 = (t23.*t687.*t1321)./2.0;
t2142 = (t26.*t687.*t1321)./2.0;
t2148 = t295+t1807;
t2167 = t126+t1961;
t2168 = t126+t1962;
t2173 = t134+t1976;
t2174 = t134+t1977;
t2201 = t571+t1677;
t2272 = t338+t1961;
t2273 = t338+t1962;
t2276 = t315+t1976;
t2277 = t315+t1977;
t2279 = t530+t1807;
t2286 = t8.*t1036.*t1298;
t2309 = t14.*t1036.*t1288;
t2338 = t8.*t647.*t1677;
t2340 = t23.*t1036.*t1302;
t2344 = t26.*t1036.*t1302;
t2354 = t8.*t670.*t1677;
t2398 = (t23.*t1036.*t1321)./2.0;
t2399 = (t23.*t1055.*t1302)./2.0;
t2400 = (t26.*t1036.*t1321)./2.0;
t2401 = (t26.*t1055.*t1302)./2.0;
t2465 = t14.*t1288.*t1302;
t2467 = t8.*t1298.*t1302;
t2483 = t169+t313+t316+t1596;
t2496 = t8.*t820.*t1677;
t2509 = t14.*t705.*t1807;
t2529 = t1364+t1372;
t2530 = t1365+t1373;
t2565 = (t8.*t843.*t1677)./2.0;
t2606 = t8.*t687.*t1977;
t2618 = t14.*t687.*t1962;
t2743 = t23.*t1082.*t1807;
t2744 = t26.*t1082.*t1807;
t2831 = (t8.*t1036.*t1977)./2.0;
t2839 = (t14.*t1036.*t1962)./2.0;
t2896 = (t14.*t1287.*t1807)./2.0;
t2897 = (t8.*t1297.*t1807)./2.0;
t2956 = t14.*t1302.*t1962;
t2960 = t8.*t1302.*t1977;
t3307 = t14.*t1807.*t1961;
t3308 = t8.*t1807.*t1976;
t192 = t176.*t5d;
t331 = t37.*t176;
t332 = t18.*t263;
t354 = t18.*t303;
t444 = t13.*t368;
t445 = t19.*t368;
t446 = t402.^2;
t455 = t418.*2.0;
t461 = t13.*t400;
t464 = t19.*t400;
t485 = -t448;
t487 = t120+t156;
t488 = t121+t159;
t489 = -t471;
t498 = t463.*t1d;
t501 = t466.*t1d;
t507 = t8.*t481;
t508 = -t468;
t509 = t12.*t480;
t510 = t12.*t481;
t511 = -t469;
t513 = t14.*t480;
t514 = t8.*t484;
t515 = -t472;
t516 = -t473;
t517 = t18.*t480;
t518 = t18.*t481;
t519 = t12.*t484;
t520 = -t474;
t521 = -t475;
t522 = t14.*t462;
t523 = t14.*t483;
t524 = -t477;
t525 = t18.*t483;
t526 = -t478;
t527 = t8.*t465;
t528 = -t482;
t538 = t12.*t483.*2.0;
t539 = t18.*t484.*2.0;
t540 = t479./2.0;
t541 = t482./2.0;
t542 = t18.*t494;
t543 = t12.*t496;
t544 = t18.*t496;
t546 = t37.*t402;
t547 = t37.*t403;
t548 = t39.*t402;
t552 = t39.*t418;
t558 = t8.*t502;
t559 = t38.*t484;
t560 = -t536;
t569 = t545.*2.0;
t570 = t166+t195;
t573 = t34.*t483;
t575 = t14.*t499;
t576 = -t533;
t577 = t35.*t484.*2.0;
t582 = t35.*t496;
t585 = t38.*t496;
t592 = t18.*t39.*t403;
t594 = -t545;
t596 = t18.*t37.*t418;
t621 = t8.*t39.*t462;
t628 = -t602;
t629 = t14.*t39.*t465;
t633 = t115.*t402;
t635 = t597.*-2.0;
t639 = t18.*t61.*t402.*2.0;
t641 = t103+t429;
t645 = t123.*t402;
t650 = t8.*t39.*t499;
t651 = -t615;
t654 = t89.*t484;
t655 = t90.*t483;
t656 = t18.*t39.*t499;
t657 = -t616;
t658 = -t620;
t659 = t14.*t39.*t502;
t660 = -t623;
t661 = t18.*t39.*t502;
t666 = t610./2.0;
t667 = t158.*t402;
t669 = t14.*t609;
t671 = t614./2.0;
t672 = t620./2.0;
t673 = t168.*t402;
t679 = t143+t401;
t682 = t28.*t39.*t494;
t684 = t140.*t483;
t689 = t18.*t152.*t402;
t690 = t642./2.0;
t716 = t150+t480;
t717 = t149+t481;
t724 = -t8.*(t101-t401);
t725 = t266.*t402;
t726 = t8.*t39.*t609;
t727 = t18.*t37.*t609;
t728 = t12.*t39.*t609;
t729 = t19.*t698;
t730 = t18.*t39.*t609;
t735 = t255.*t402;
t736 = t256.*t402;
t737 = t255.*t403;
t739 = t8.*t37.*t609;
t740 = t13.*t698;
t747 = t14.*t721;
t748 = t14.*t723;
t752 = t19.*t733;
t759 = t329.*t402;
t760 = t330.*t402;
t761 = t330.*t403;
t762 = -t734;
t766 = t744.*2.0;
t775 = t12.*t738;
t776 = t18.*t738;
t778 = -t738;
Y = ft_2({t100,t1002,t1003,t101,t1016,t1036,t104,t1051,t1052,t1055,t106,t1065,t1066,t107,t1075,t108,t1082,t1085,t1089,t1092,t1093,t1094,t1096,t1097,t1098,t1104,t111,t112,t1121,t1122,t1123,t113,t1133,t1134,t1135,t1139,t1140,t1141,t1142,t115,t1163,t1164,t1165,t1166,t1169,t1172,t1174,t1194,t12,t1200,t1203,t1215,t1222,t124,t1245,t1246,t1248,t1256,t1257,t1258,t1265,t127,t128,t1287,t1288,t1297,t1298,t1299,t13,t1302,t1303,t131,t132,t1321,t1330,t1331,t1332,t1333,t1334,t1335,t134,t1352,t1355,t1358,t136,t1368,t137,t1375,t1378,t138,t1380,t1381,t14,t1410,t1413,t1414,t1415,t1426,t1427,t1431,t1432,t1462,t1463,t1470,t1481,t1485,t1488,t1492,t1494,t1495,t1499,t15,t150,t1500,t1501,t1506,t1512,t1515,t1516,t1517,t1518,t1519,t152,t1520,t1521,t1534,t1540,t1541,t1547,t155,t156,t1576,t158,t159,t1595,t160,t162,t163,t164,t165,t1650,t1651,t1652,t1653,t1666,t1669,t1674,t1677,t169,t170,t1709,t171,t1710,t1713,t1714,t1729,t173,t1731,t174,t1745,t175,t1751,t1754,t1755,t1758,t177,t179,t18,t180,t1807,t1818,t183,t1837,t184,t1840,t185,t186,t1863,t1868,t187,t1888,t1889,t189,t1890,t1891,t19,t190,t1906,t191,t1910,t192,t196,t1961,t1962,t1976,t1977,t199,t1d,t1dd,t200,t2003,t2006,t2007,t2008,t201,t202,t2034,t2035,t2040,t2041,t2043,t2044,t2051,t2055,t2056,t206,t207,t2070,t2081,t2087,t209,t21,t210,t2100,t2101,t2109,t211,t2113,t2118,t213,t2141,t2142,t2148,t215,t2167,t2168,t2173,t2174,t219,t22,t220,t2201,t221,t226,t2272,t2273,t2276,t2277,t2279,t228,t2286,t229,t23,t2309,t231,t232,t233,t2338,t234,t2340,t2344,t235,t2354,t2398,t2399,t24,t2400,t2401,t241,t243,t244,t245,t2465,t2467,t247,t248,t2483,t249,t2496,t25,t2509,t2529,t2530,t255,t256,t2565,t258,t26,t2606,t261,t2618,t263,t265,t266,t268,t27,t270,t273,t2743,t2744,t276,t278,t279,t28,t281,t282,t283,t2831,t2839,t285,t287,t288,t289,t2896,t2897,t29,t292,t293,t2956,t296,t2960,t299,t2d,t2dd,t30,t301,t303,t304,t308,t309,t31,t310,t313,t315,t316,t317,t318,t319,t320,t321,t322,t325,t328,t329,t330,t3307,t3308,t331,t332,t333,t334,t335,t336,t337,t339,t34,t341,t342,t343,t344,t345,t346,t347,t35,t351,t353,t354,t36,t360,t361,t363,t364,t365,t368,t37,t375,t38,t383,t384,t39,t390,t392,t393,t394,t395,t3d,t3dd,t400,t401,t402,t403,t404,t41,t410,t411,t412,t413,t414,t415,t416,t417,t418,t419,t42,t420,t423,t424,t425,t428,t43,t431,t434,t437,t439,t440,t441,t442,t443,t444,t445,t446,t447,t449,t453,t454,t455,t459,t461,t463,t464,t466,t467,t468,t470,t472,t473,t476,t477,t478,t479,t48,t483,t484,t485,t486,t487,t488,t489,t490,t491,t492,t493,t494,t495,t496,t497,t498,t499,t4d,t4dd,t50,t501,t502,t503,t504,t506,t507,t508,t509,t51,t510,t511,t513,t514,t515,t516,t517,t518,t519,t520,t521,t522,t523,t524,t525,t526,t527,t528,t529,t53,t530,t532,t535,t536,t537,t538,t539,t540,t541,t542,t543,t544,t545,t546,t547,t548,t55,t550,t552,t553,t554,t555,t556,t557,t558,t559,t56,t560,t561,t562,t569,t57,t570,t571,t573,t574,t575,t576,t577,t578,t579,t58,t582,t585,t592,t594,t596,t5d,t5dd,t602,t603,t606,t609,t61,t614,t615,t616,t617,t619,t621,t623,t624,t628,t629,t63,t633,t634,t635,t636,t637,t639,t641,t642,t644,t645,t647,t648,t649,t650,t651,t652,t653,t654,t655,t656,t657,t658,t659,t660,t661,t664,t666,t667,t669,t670,t671,t672,t673,t675,t682,t684,t687,t689,t69,t690,t695,t696,t697,t698,t699,t6d,t6dd,t700,t703,t705,t706,t709,t71,t710,t716,t717,t719,t720,t721,t722,t723,t724,t725,t726,t727,t728,t729,t730,t731,t732,t733,t735,t736,t737,t738,t739,t740,t741,t742,t743,t744,t745,t746,t747,t748,t749,t75,t750,t751,t752,t759,t760,t761,t762,t766,t768,t769,t771,t772,t773,t774,t775,t776,t778,t779,t782,t791,t793,t799,t8,t802,t811,t818,t819,t82,t820,t824,t828,t830,t836,t840,t841,t842,t843,t844,t849,t850,t855,t856,t857,t859,t860,t862,t863,t865,t869,t870,t872,t873,t874,t875,t88,t880,t881,t884,t885,t886,t890,t892,t893,t896,t897,t899,t9,t900,t907,t921,t924,t925,t932,t933,t934,t935,t936,t940,t941,t942,t963,t966,t970,t973});
end
function Y = ft_2(ct)
t100 = ct{1};
t1002 = ct{2};
t1003 = ct{3};
t101 = ct{4};
t1016 = ct{5};
t1036 = ct{6};
t104 = ct{7};
t1051 = ct{8};
t1052 = ct{9};
t1055 = ct{10};
t106 = ct{11};
t1065 = ct{12};
t1066 = ct{13};
t107 = ct{14};
t1075 = ct{15};
t108 = ct{16};
t1082 = ct{17};
t1085 = ct{18};
t1089 = ct{19};
t1092 = ct{20};
t1093 = ct{21};
t1094 = ct{22};
t1096 = ct{23};
t1097 = ct{24};
t1098 = ct{25};
t1104 = ct{26};
t111 = ct{27};
t112 = ct{28};
t1121 = ct{29};
t1122 = ct{30};
t1123 = ct{31};
t113 = ct{32};
t1133 = ct{33};
t1134 = ct{34};
t1135 = ct{35};
t1139 = ct{36};
t1140 = ct{37};
t1141 = ct{38};
t1142 = ct{39};
t115 = ct{40};
t1163 = ct{41};
t1164 = ct{42};
t1165 = ct{43};
t1166 = ct{44};
t1169 = ct{45};
t1172 = ct{46};
t1174 = ct{47};
t1194 = ct{48};
t12 = ct{49};
t1200 = ct{50};
t1203 = ct{51};
t1215 = ct{52};
t1222 = ct{53};
t124 = ct{54};
t1245 = ct{55};
t1246 = ct{56};
t1248 = ct{57};
t1256 = ct{58};
t1257 = ct{59};
t1258 = ct{60};
t1265 = ct{61};
t127 = ct{62};
t128 = ct{63};
t1287 = ct{64};
t1288 = ct{65};
t1297 = ct{66};
t1298 = ct{67};
t1299 = ct{68};
t13 = ct{69};
t1302 = ct{70};
t1303 = ct{71};
t131 = ct{72};
t132 = ct{73};
t1321 = ct{74};
t1330 = ct{75};
t1331 = ct{76};
t1332 = ct{77};
t1333 = ct{78};
t1334 = ct{79};
t1335 = ct{80};
t134 = ct{81};
t1352 = ct{82};
t1355 = ct{83};
t1358 = ct{84};
t136 = ct{85};
t1368 = ct{86};
t137 = ct{87};
t1375 = ct{88};
t1378 = ct{89};
t138 = ct{90};
t1380 = ct{91};
t1381 = ct{92};
t14 = ct{93};
t1410 = ct{94};
t1413 = ct{95};
t1414 = ct{96};
t1415 = ct{97};
t1426 = ct{98};
t1427 = ct{99};
t1431 = ct{100};
t1432 = ct{101};
t1462 = ct{102};
t1463 = ct{103};
t1470 = ct{104};
t1481 = ct{105};
t1485 = ct{106};
t1488 = ct{107};
t1492 = ct{108};
t1494 = ct{109};
t1495 = ct{110};
t1499 = ct{111};
t15 = ct{112};
t150 = ct{113};
t1500 = ct{114};
t1501 = ct{115};
t1506 = ct{116};
t1512 = ct{117};
t1515 = ct{118};
t1516 = ct{119};
t1517 = ct{120};
t1518 = ct{121};
t1519 = ct{122};
t152 = ct{123};
t1520 = ct{124};
t1521 = ct{125};
t1534 = ct{126};
t1540 = ct{127};
t1541 = ct{128};
t1547 = ct{129};
t155 = ct{130};
t156 = ct{131};
t1576 = ct{132};
t158 = ct{133};
t159 = ct{134};
t1595 = ct{135};
t160 = ct{136};
t162 = ct{137};
t163 = ct{138};
t164 = ct{139};
t165 = ct{140};
t1650 = ct{141};
t1651 = ct{142};
t1652 = ct{143};
t1653 = ct{144};
t1666 = ct{145};
t1669 = ct{146};
t1674 = ct{147};
t1677 = ct{148};
t169 = ct{149};
t170 = ct{150};
t1709 = ct{151};
t171 = ct{152};
t1710 = ct{153};
t1713 = ct{154};
t1714 = ct{155};
t1729 = ct{156};
t173 = ct{157};
t1731 = ct{158};
t174 = ct{159};
t1745 = ct{160};
t175 = ct{161};
t1751 = ct{162};
t1754 = ct{163};
t1755 = ct{164};
t1758 = ct{165};
t177 = ct{166};
t179 = ct{167};
t18 = ct{168};
t180 = ct{169};
t1807 = ct{170};
t1818 = ct{171};
t183 = ct{172};
t1837 = ct{173};
t184 = ct{174};
t1840 = ct{175};
t185 = ct{176};
t186 = ct{177};
t1863 = ct{178};
t1868 = ct{179};
t187 = ct{180};
t1888 = ct{181};
t1889 = ct{182};
t189 = ct{183};
t1890 = ct{184};
t1891 = ct{185};
t19 = ct{186};
t190 = ct{187};
t1906 = ct{188};
t191 = ct{189};
t1910 = ct{190};
t192 = ct{191};
t196 = ct{192};
t1961 = ct{193};
t1962 = ct{194};
t1976 = ct{195};
t1977 = ct{196};
t199 = ct{197};
t1d = ct{198};
t1dd = ct{199};
t200 = ct{200};
t2003 = ct{201};
t2006 = ct{202};
t2007 = ct{203};
t2008 = ct{204};
t201 = ct{205};
t202 = ct{206};
t2034 = ct{207};
t2035 = ct{208};
t2040 = ct{209};
t2041 = ct{210};
t2043 = ct{211};
t2044 = ct{212};
t2051 = ct{213};
t2055 = ct{214};
t2056 = ct{215};
t206 = ct{216};
t207 = ct{217};
t2070 = ct{218};
t2081 = ct{219};
t2087 = ct{220};
t209 = ct{221};
t21 = ct{222};
t210 = ct{223};
t2100 = ct{224};
t2101 = ct{225};
t2109 = ct{226};
t211 = ct{227};
t2113 = ct{228};
t2118 = ct{229};
t213 = ct{230};
t2141 = ct{231};
t2142 = ct{232};
t2148 = ct{233};
t215 = ct{234};
t2167 = ct{235};
t2168 = ct{236};
t2173 = ct{237};
t2174 = ct{238};
t219 = ct{239};
t22 = ct{240};
t220 = ct{241};
t2201 = ct{242};
t221 = ct{243};
t226 = ct{244};
t2272 = ct{245};
t2273 = ct{246};
t2276 = ct{247};
t2277 = ct{248};
t2279 = ct{249};
t228 = ct{250};
t2286 = ct{251};
t229 = ct{252};
t23 = ct{253};
t2309 = ct{254};
t231 = ct{255};
t232 = ct{256};
t233 = ct{257};
t2338 = ct{258};
t234 = ct{259};
t2340 = ct{260};
t2344 = ct{261};
t235 = ct{262};
t2354 = ct{263};
t2398 = ct{264};
t2399 = ct{265};
t24 = ct{266};
t2400 = ct{267};
t2401 = ct{268};
t241 = ct{269};
t243 = ct{270};
t244 = ct{271};
t245 = ct{272};
t2465 = ct{273};
t2467 = ct{274};
t247 = ct{275};
t248 = ct{276};
t2483 = ct{277};
t249 = ct{278};
t2496 = ct{279};
t25 = ct{280};
t2509 = ct{281};
t2529 = ct{282};
t2530 = ct{283};
t255 = ct{284};
t256 = ct{285};
t2565 = ct{286};
t258 = ct{287};
t26 = ct{288};
t2606 = ct{289};
t261 = ct{290};
t2618 = ct{291};
t263 = ct{292};
t265 = ct{293};
t266 = ct{294};
t268 = ct{295};
t27 = ct{296};
t270 = ct{297};
t273 = ct{298};
t2743 = ct{299};
t2744 = ct{300};
t276 = ct{301};
t278 = ct{302};
t279 = ct{303};
t28 = ct{304};
t281 = ct{305};
t282 = ct{306};
t283 = ct{307};
t2831 = ct{308};
t2839 = ct{309};
t285 = ct{310};
t287 = ct{311};
t288 = ct{312};
t289 = ct{313};
t2896 = ct{314};
t2897 = ct{315};
t29 = ct{316};
t292 = ct{317};
t293 = ct{318};
t2956 = ct{319};
t296 = ct{320};
t2960 = ct{321};
t299 = ct{322};
t2d = ct{323};
t2dd = ct{324};
t30 = ct{325};
t301 = ct{326};
t303 = ct{327};
t304 = ct{328};
t308 = ct{329};
t309 = ct{330};
t31 = ct{331};
t310 = ct{332};
t313 = ct{333};
t315 = ct{334};
t316 = ct{335};
t317 = ct{336};
t318 = ct{337};
t319 = ct{338};
t320 = ct{339};
t321 = ct{340};
t322 = ct{341};
t325 = ct{342};
t328 = ct{343};
t329 = ct{344};
t330 = ct{345};
t3307 = ct{346};
t3308 = ct{347};
t331 = ct{348};
t332 = ct{349};
t333 = ct{350};
t334 = ct{351};
t335 = ct{352};
t336 = ct{353};
t337 = ct{354};
t339 = ct{355};
t34 = ct{356};
t341 = ct{357};
t342 = ct{358};
t343 = ct{359};
t344 = ct{360};
t345 = ct{361};
t346 = ct{362};
t347 = ct{363};
t35 = ct{364};
t351 = ct{365};
t353 = ct{366};
t354 = ct{367};
t36 = ct{368};
t360 = ct{369};
t361 = ct{370};
t363 = ct{371};
t364 = ct{372};
t365 = ct{373};
t368 = ct{374};
t37 = ct{375};
t375 = ct{376};
t38 = ct{377};
t383 = ct{378};
t384 = ct{379};
t39 = ct{380};
t390 = ct{381};
t392 = ct{382};
t393 = ct{383};
t394 = ct{384};
t395 = ct{385};
t3d = ct{386};
t3dd = ct{387};
t400 = ct{388};
t401 = ct{389};
t402 = ct{390};
t403 = ct{391};
t404 = ct{392};
t41 = ct{393};
t410 = ct{394};
t411 = ct{395};
t412 = ct{396};
t413 = ct{397};
t414 = ct{398};
t415 = ct{399};
t416 = ct{400};
t417 = ct{401};
t418 = ct{402};
t419 = ct{403};
t42 = ct{404};
t420 = ct{405};
t423 = ct{406};
t424 = ct{407};
t425 = ct{408};
t428 = ct{409};
t43 = ct{410};
t431 = ct{411};
t434 = ct{412};
t437 = ct{413};
t439 = ct{414};
t440 = ct{415};
t441 = ct{416};
t442 = ct{417};
t443 = ct{418};
t444 = ct{419};
t445 = ct{420};
t446 = ct{421};
t447 = ct{422};
t449 = ct{423};
t453 = ct{424};
t454 = ct{425};
t455 = ct{426};
t459 = ct{427};
t461 = ct{428};
t463 = ct{429};
t464 = ct{430};
t466 = ct{431};
t467 = ct{432};
t468 = ct{433};
t470 = ct{434};
t472 = ct{435};
t473 = ct{436};
t476 = ct{437};
t477 = ct{438};
t478 = ct{439};
t479 = ct{440};
t48 = ct{441};
t483 = ct{442};
t484 = ct{443};
t485 = ct{444};
t486 = ct{445};
t487 = ct{446};
t488 = ct{447};
t489 = ct{448};
t490 = ct{449};
t491 = ct{450};
t492 = ct{451};
t493 = ct{452};
t494 = ct{453};
t495 = ct{454};
t496 = ct{455};
t497 = ct{456};
t498 = ct{457};
t499 = ct{458};
t4d = ct{459};
t4dd = ct{460};
t50 = ct{461};
t501 = ct{462};
t502 = ct{463};
t503 = ct{464};
t504 = ct{465};
t506 = ct{466};
t507 = ct{467};
t508 = ct{468};
t509 = ct{469};
t51 = ct{470};
t510 = ct{471};
t511 = ct{472};
t513 = ct{473};
t514 = ct{474};
t515 = ct{475};
t516 = ct{476};
t517 = ct{477};
t518 = ct{478};
t519 = ct{479};
t520 = ct{480};
t521 = ct{481};
t522 = ct{482};
t523 = ct{483};
t524 = ct{484};
t525 = ct{485};
t526 = ct{486};
t527 = ct{487};
t528 = ct{488};
t529 = ct{489};
t53 = ct{490};
t530 = ct{491};
t532 = ct{492};
t535 = ct{493};
t536 = ct{494};
t537 = ct{495};
t538 = ct{496};
t539 = ct{497};
t540 = ct{498};
t541 = ct{499};
t542 = ct{500};
t543 = ct{501};
t544 = ct{502};
t545 = ct{503};
t546 = ct{504};
t547 = ct{505};
t548 = ct{506};
t55 = ct{507};
t550 = ct{508};
t552 = ct{509};
t553 = ct{510};
t554 = ct{511};
t555 = ct{512};
t556 = ct{513};
t557 = ct{514};
t558 = ct{515};
t559 = ct{516};
t56 = ct{517};
t560 = ct{518};
t561 = ct{519};
t562 = ct{520};
t569 = ct{521};
t57 = ct{522};
t570 = ct{523};
t571 = ct{524};
t573 = ct{525};
t574 = ct{526};
t575 = ct{527};
t576 = ct{528};
t577 = ct{529};
t578 = ct{530};
t579 = ct{531};
t58 = ct{532};
t582 = ct{533};
t585 = ct{534};
t592 = ct{535};
t594 = ct{536};
t596 = ct{537};
t5d = ct{538};
t5dd = ct{539};
t602 = ct{540};
t603 = ct{541};
t606 = ct{542};
t609 = ct{543};
t61 = ct{544};
t614 = ct{545};
t615 = ct{546};
t616 = ct{547};
t617 = ct{548};
t619 = ct{549};
t621 = ct{550};
t623 = ct{551};
t624 = ct{552};
t628 = ct{553};
t629 = ct{554};
t63 = ct{555};
t633 = ct{556};
t634 = ct{557};
t635 = ct{558};
t636 = ct{559};
t637 = ct{560};
t639 = ct{561};
t641 = ct{562};
t642 = ct{563};
t644 = ct{564};
t645 = ct{565};
t647 = ct{566};
t648 = ct{567};
t649 = ct{568};
t650 = ct{569};
t651 = ct{570};
t652 = ct{571};
t653 = ct{572};
t654 = ct{573};
t655 = ct{574};
t656 = ct{575};
t657 = ct{576};
t658 = ct{577};
t659 = ct{578};
t660 = ct{579};
t661 = ct{580};
t664 = ct{581};
t666 = ct{582};
t667 = ct{583};
t669 = ct{584};
t670 = ct{585};
t671 = ct{586};
t672 = ct{587};
t673 = ct{588};
t675 = ct{589};
t682 = ct{590};
t684 = ct{591};
t687 = ct{592};
t689 = ct{593};
t69 = ct{594};
t690 = ct{595};
t695 = ct{596};
t696 = ct{597};
t697 = ct{598};
t698 = ct{599};
t699 = ct{600};
t6d = ct{601};
t6dd = ct{602};
t700 = ct{603};
t703 = ct{604};
t705 = ct{605};
t706 = ct{606};
t709 = ct{607};
t71 = ct{608};
t710 = ct{609};
t716 = ct{610};
t717 = ct{611};
t719 = ct{612};
t720 = ct{613};
t721 = ct{614};
t722 = ct{615};
t723 = ct{616};
t724 = ct{617};
t725 = ct{618};
t726 = ct{619};
t727 = ct{620};
t728 = ct{621};
t729 = ct{622};
t730 = ct{623};
t731 = ct{624};
t732 = ct{625};
t733 = ct{626};
t735 = ct{627};
t736 = ct{628};
t737 = ct{629};
t738 = ct{630};
t739 = ct{631};
t740 = ct{632};
t741 = ct{633};
t742 = ct{634};
t743 = ct{635};
t744 = ct{636};
t745 = ct{637};
t746 = ct{638};
t747 = ct{639};
t748 = ct{640};
t749 = ct{641};
t75 = ct{642};
t750 = ct{643};
t751 = ct{644};
t752 = ct{645};
t759 = ct{646};
t760 = ct{647};
t761 = ct{648};
t762 = ct{649};
t766 = ct{650};
t768 = ct{651};
t769 = ct{652};
t771 = ct{653};
t772 = ct{654};
t773 = ct{655};
t774 = ct{656};
t775 = ct{657};
t776 = ct{658};
t778 = ct{659};
t779 = ct{660};
t782 = ct{661};
t791 = ct{662};
t793 = ct{663};
t799 = ct{664};
t8 = ct{665};
t802 = ct{666};
t811 = ct{667};
t818 = ct{668};
t819 = ct{669};
t82 = ct{670};
t820 = ct{671};
t824 = ct{672};
t828 = ct{673};
t830 = ct{674};
t836 = ct{675};
t840 = ct{676};
t841 = ct{677};
t842 = ct{678};
t843 = ct{679};
t844 = ct{680};
t849 = ct{681};
t850 = ct{682};
t855 = ct{683};
t856 = ct{684};
t857 = ct{685};
t859 = ct{686};
t860 = ct{687};
t862 = ct{688};
t863 = ct{689};
t865 = ct{690};
t869 = ct{691};
t870 = ct{692};
t872 = ct{693};
t873 = ct{694};
t874 = ct{695};
t875 = ct{696};
t88 = ct{697};
t880 = ct{698};
t881 = ct{699};
t884 = ct{700};
t885 = ct{701};
t886 = ct{702};
t890 = ct{703};
t892 = ct{704};
t893 = ct{705};
t896 = ct{706};
t897 = ct{707};
t899 = ct{708};
t9 = ct{709};
t900 = ct{710};
t907 = ct{711};
t921 = ct{712};
t924 = ct{713};
t925 = ct{714};
t932 = ct{715};
t933 = ct{716};
t934 = ct{717};
t935 = ct{718};
t936 = ct{719};
t940 = ct{720};
t941 = ct{721};
t942 = ct{722};
t963 = ct{723};
t966 = ct{724};
t970 = ct{725};
t973 = ct{726};
t780 = t35.*t39.*t609;
t781 = t18.*t61.*t609;
t784 = t13.*t733;
t786 = t18.*t63.*t609;
t788 = t339+t428;
t789 = t363+t400;
t790 = t270+t470;
t797 = t738./2.0;
t800 = -t745;
t801 = -t746;
t807 = -t14.*t37.*(t101-t401);
t809 = -t18.*t37.*(t101-t401);
t810 = -t12.*t39.*(t101-t401);
t812 = t293+t483;
t813 = t292+t484;
t815 = -t14.*t39.*(t101-t401);
t816 = -t18.*t39.*(t101-t401);
t821 = t14.*t741;
t822 = t8.*t743;
t823 = t34.*t738;
t825 = t35.*t738;
t826 = t36.*t738;
t827 = t38.*t738;
t831 = t341.*t402.*t1d;
t832 = t341.*t403.*t1d;
t833 = t342.*t402.*t1d;
t834 = t255.*t502;
t835 = -t779;
t845 = t37.*t721;
t846 = t37.*t723;
t847 = t402.*t403;
t852 = t772./2.0;
t853 = t390+t440;
t854 = t774./2.0;
t861 = t341.*t402.*t6d.*2.0;
t864 = t37.*t738;
t866 = -t38.*t39.*(t101-t401);
t867 = -t18.*t63.*(t101-t401);
t868 = t18.*t37.*(t101-t401);
t871 = t14.*t39.*(t101-t401);
t879 = -t828;
t883 = -t14.*(t206-t470);
t887 = t330.*t499;
t894 = -t18.*t61.*(t101-t401);
t901 = t341.*t499;
t902 = t402.*t453;
t903 = t8.*t39.*t721;
t904 = t18.*t37.*t722;
t905 = t12.*t39.*t722;
t906 = t8.*t39.*t723;
t909 = t18.*t39.*t721;
t910 = t18.*t39.*t722;
t911 = t341.*t502;
t912 = t402.*t459;
t913 = -t844;
t914 = -t8.*(t249-t483);
t916 = -t14.*(t248-t484);
t928 = t14.*t824;
t937 = t38.*t39.*(t101-t401);
t938 = -t870;
t939 = -t873;
t943 = t402.*t494;
t944 = t403.*t494;
t945 = t402.*t495;
t946 = t402.*t496;
t948 = -t890;
t952 = t402.*t499;
t953 = t38.*t39.*t722;
t954 = t104.*t738;
t956 = t107.*t738;
t958 = t402.*t502;
t959 = t8.*t39.*t741;
t965 = t14.*t39.*t743;
t968 = t14.*(t206-t470).*(-1.0./2.0);
t969 = t256.*t609;
t981 = -t933;
t984 = t8.*(t249-t483).*(-1.0./2.0);
t985 = t14.*(t248-t484).*(-1.0./2.0);
t989 = t402.*t545;
t990 = t963.*(-1.0./2.0);
t995 = t970.*(-1.0./2.0);
t1008 = t963./2.0;
t1015 = t330.*t609;
t1018 = t970./2.0;
t1022 = -t8.*t39.*(t206-t470);
t1027 = t341.*t609;
t1028 = t342.*t609;
t1029 = t179.*t738;
t1030 = t180.*t738;
t1037 = -t8.*t39.*(t248-t484);
t1040 = -t14.*t39.*(t249-t483);
t1069 = -t255.*(t101-t401);
t1070 = t137+t317+t368;
t1076 = t403.*t609;
t1086 = t8.*t39.*(t248-t484);
t1087 = t14.*t39.*(t249-t483);
t1099 = t8.*t39.*(t206-t470).*(-1.0./2.0);
t1105 = t402.*t609.*2.0;
t1137 = -t329.*(t101-t401);
t1149 = -t402.*(t100-t364);
t1150 = -t403.*(t100-t364);
t1153 = -t341.*(t101-t401);
t1154 = -t342.*(t101-t401);
t1170 = t127+t824;
t1175 = t255.*t722;
t1179 = t341.*t695;
t1188 = t1085./2.0;
t1193 = t329.*(t101-t401);
t1195 = -t1142;
t1197 = t402.*(t100-t364);
t1198 = -t403.*(t101-t401);
t1213 = t329.*t722;
t1214 = t330.*t721;
t1223 = t402.*(t101-t401).*-2.0;
t1229 = t1164./2.0;
t1235 = t1166./2.0;
t1242 = t8.*t1169;
t1243 = -t1194;
t1275 = t8.*t209.*t824;
t1276 = t30.*t170.*t824;
t1279 = t308.*t824;
t1283 = -t8.*t494.*(t100-t364);
t1349 = -t1303;
t1353 = t8.*t494.*(t100-t364).*(-1.0./2.0);
t1399 = t439+t819;
t1416 = -t1380;
t1417 = -t1381;
t1455 = t14.*t1413;
t1469 = t8.*t1410;
t1511 = t8.*t530.*t824;
t1532 = t232+t557+t574;
t1535 = t233+t556+t561;
t1542 = t14.*t1515;
t1548 = (t8.*t529.*t824)./2.0;
t1570 = t8.*t1512;
t1574 = t8.*t687.*t723;
t1575 = t351+t353+t722;
t1618 = t1547./2.0;
t1640 = t282+t603+t606;
t1699 = t733+t811;
t1704 = t37.*t1576;
t1706 = t39.*t1576;
t1728 = t37.*t1595;
t1730 = t39.*t1595;
t1732 = t325.*t1410;
t1733 = t14.*t37.*t1410.*4.0975e-2;
t1736 = t8.*t1674;
t1740 = t322.*t1413;
t1741 = t8.*t37.*t1413.*4.0975e-2;
t1759 = t14.*t37.*t1410.*(-8.195e-2);
t1769 = t8.*t1729;
t1772 = t8.*t1731;
t1788 = -t1745;
t1804 = t862+t863;
t1811 = t200+t709+t710;
t1812 = t856+t857;
t1866 = t8.*t723.*t1036;
t1930 = t1837./2.0;
t1937 = -t1906;
t1942 = t555+t1413;
t1955 = t791+t1121;
t1965 = t1888./2.0;
t1968 = t1889./2.0;
t1969 = t1890./2.0;
t1973 = t1891./2.0;
t1984 = t619+t1368;
t1989 = t771+t1163;
t1994 = t773+t1165;
t2017 = t8.*t39.*t1818;
t2019 = t14.*t39.*t1818;
t2037 = -t2003;
t2038 = -t2006;
t2039 = -t2007;
t2045 = t325.*t1674;
t2047 = t328.*t1674;
t2048 = t14.*t39.*t1674.*4.0975e-2;
t2063 = -t37.*(t738-t1085);
t2074 = -t2043;
t2075 = t8.*t647.*t1413;
t2085 = t8.*t723.*t1302;
t2089 = t14.*t647.*t1410;
t2090 = t2043./2.0;
t2093 = t2044./2.0;
t2110 = t37.*(t738-t1085).*(-1.0./2.0);
t2117 = t2070./2.0;
t2123 = t818+t1299;
t2140 = t241+t1818;
t2144 = t2100./2.0;
t2145 = t2101./2.0;
t2147 = t2113.^2;
t2158 = t296+t1818;
t2170 = t578+t699+t751;
t2197 = t550+t1674;
t2217 = t8.*t2167;
t2218 = t8.*t2168;
t2231 = t14.*t2173;
t2232 = t14.*t2174;
t2254 = t14.*t2201;
t2298 = (t14.*t820.*t1410)./2.0;
t2300 = t1200+t1215;
t2303 = (t8.*t820.*t1413)./2.0;
t2311 = t2279.^2;
t2312 = t35.*t39.*t2148;
t2315 = t38.*t39.*t2148;
t2334 = t14.*t647.*t1674;
t2336 = t8.*t2272;
t2337 = t8.*t2273;
t2341 = t14.*t2276;
t2342 = t14.*t2277;
t2346 = -t2309;
t2348 = t2286./2.0;
t2353 = t14.*t670.*t1674;
t2357 = t285+t336+t337+t529+t719;
t2359 = t2309./2.0;
t2395 = t2354./2.0;
t2434 = t255.*t2148;
t2435 = t256.*t2148;
t2470 = t171+t273+t335+t1576;
t2472 = t329.*t2148;
t2473 = t330.*t2148;
t2482 = t169+t313+t316+t1595;
t2490 = -t2465;
t2495 = t14.*t820.*t1674;
t2507 = t860+t1729;
t2508 = t2465./2.0;
t2511 = t2467./2.0;
t2527 = t8.*t721.*t1807;
t2540 = t14.*t2483;
t2542 = -t2509;
t2557 = t2509./2.0;
t2560 = (t14.*t843.*t1674)./2.0;
t2633 = t791+t1961;
t2634 = t791+t1962;
t2638 = t555+t2173;
t2639 = t555+t2174;
t2642 = -t2618;
t2644 = t2606./2.0;
t2648 = t2618./2.0;
t2659 = t127+t2483;
t2685 = t940+t941+t942;
t2692 = t934+t935+t936;
t2708 = t14.*t705.*t2113;
t2718 = t8.*t721.*t2113;
t2745 = t8.*t687.*t2174;
t2748 = t14.*t687.*t2168;
t2749 = t1481+t1540;
t2776 = t2743./2.0;
t2777 = t2744./2.0;
t2849 = -t2831;
t2862 = t14.*t705.*t2279;
t2876 = t8.*t721.*t2279;
t2919 = -t2896;
t2983 = t23.*t1082.*t2113;
t2985 = t26.*t1082.*t2113;
t2987 = t8.*t1036.*t2174;
t2989 = -t2960;
t2995 = t14.*t1036.*t2168;
t2996 = t2956./2.0;
t2999 = t2960./2.0;
t3035 = t8.*t1297.*t2113;
t3046 = t14.*t1287.*t2113;
t3086 = t23.*t1082.*t2279;
t3088 = t26.*t1082.*t2279;
t3122 = (t14.*t1302.*t2168)./2.0;
t3131 = (t8.*t1302.*t2174)./2.0;
t3178 = t14.*t1287.*t2279;
t3183 = t8.*t1297.*t2279;
t3288 = (t23.*t1807.*t1818)./2.0;
t3289 = t23.*t1807.*t1818.*(3.0./2.0);
t3291 = (t26.*t1807.*t1818)./2.0;
t3292 = t26.*t1807.*t1818.*(3.0./2.0);
t3321 = -t3307;
t3330 = t3307./2.0;
t3332 = t3308./2.0;
t3388 = t23.*t1807.*t2113;
t3391 = t26.*t1807.*t2113;
t3400 = t23.*t1818.*t2113;
t3401 = t26.*t1818.*t2113;
t3404 = t2034+t2040;
t3405 = t2035+t2041;
t3415 = t8.*t1807.*t2173;
t3422 = t14.*t1807.*t2167;
t3488 = (t8.*t1976.*t2113)./2.0;
t3496 = (t14.*t1961.*t2113)./2.0;
t3509 = t23.*t1807.*t2279;
t3510 = t26.*t1807.*t2279;
t3516 = t23.*t1818.*t2279;
t3517 = t26.*t1818.*t2279;
t3553 = t14.*t1961.*t2279;
t3557 = t8.*t1976.*t2279;
t3575 = t8.*t2113.*t2173;
t3593 = t14.*t2113.*t2167;
t3683 = t23.*t2113.*t2279;
t3685 = t26.*t2113.*t2279;
t3743 = (t14.*t2167.*t2279)./2.0;
t3746 = (t8.*t2173.*t2279)./2.0;
t3905 = t886+t924+t1432+t1731;
t500 = t446.*2.0;
t549 = -t498;
t563 = -t525;
t564 = -t527;
t565 = -t541;
t566 = t542.*2.0;
t567 = t543.*2.0;
t580 = t522./2.0;
t581 = t527./2.0;
t587 = t18.*t546;
t588 = t12.*t548;
t589 = -t543;
t591 = t18.*t548;
t593 = -t544;
t595 = -t569;
t598 = t39.*t446;
t601 = t37.*t487;
t607 = t592.*2.0;
t608 = t37.*t488;
t612 = t552./2.0;
t613 = -t575;
t625 = t35.*t548;
t626 = -t582;
t627 = t38.*t548;
t630 = -t592;
t632 = t18.*t37.*t446;
t643 = t596./2.0;
t668 = t633.*-2.0;
t674 = t621./2.0;
t676 = t629./2.0;
t681 = -t666;
t683 = -t650;
t685 = -t672;
t686 = -t659;
t694 = t8.*t641;
t701 = t654./2.0;
t702 = t655./2.0;
t711 = t28.*t39.*t546;
t712 = -t682;
t713 = t682.*-2.0;
t753 = t19.*t735;
t754 = -t729;
t755 = t14.*t37.*t641;
t756 = t18.*t37.*t641;
t757 = t12.*t39.*t641;
t763 = -t736;
t764 = t14.*t39.*t641;
t765 = t18.*t39.*t641;
t767 = t8.*t716;
t770 = t14.*t717;
t783 = -t739;
t785 = t13.*t735;
t792 = t186+t509;
t794 = t183+t518;
t796 = t189+t520;
t803 = t19.*t760;
t804 = -t752;
t805 = t38.*t39.*t641;
t806 = t18.*t63.*t641;
t814 = -t759;
t829 = -t797;
t838 = t13.*t760;
t839 = t18.*t61.*t641;
t877 = t847.*2.0;
t891 = -t834;
t898 = t423+t461;
t908 = t424+t464;
t915 = t821./2.0;
t917 = t822./2.0;
t919 = t8.*t37.*t717;
t922 = t14.*t37.*t716;
t923 = t8.*t39.*t717;
t927 = t14.*t39.*t716;
t931 = t37.*t778;
t950 = t37.*t797;
t955 = -t905;
t957 = -t910;
t960 = t943.*2.0;
t961 = t944.*2.0;
t962 = t945.*2.0;
t964 = t946.*2.0;
t971 = -t928;
t972 = t22.*t853;
t974 = t37.*t788;
t975 = t37.*t789;
t978 = t39.*t788;
t979 = t39.*t789;
t980 = t864.*(-1.0./2.0);
t986 = t402.*t542;
t987 = t402.*t544;
t988 = t403.*t544;
t991 = t447+t485;
t992 = -t946;
t998 = -t952;
t999 = -t953;
t1000 = t53.*t788;
t1001 = t53.*t789;
t1007 = t402.*t569;
t1017 = -t969;
t1021 = t255.*t641;
t1034 = t959./2.0;
t1041 = t965./2.0;
t1045 = t106.*t788;
t1046 = t111.*t789;
t1047 = t112.*t788;
t1048 = t115.*t789;
t1059 = t18.*t61.*t789;
t1062 = t18.*t63.*t789;
t1068 = t329.*t641;
t1071 = t479+t528;
t1077 = t342.*t641;
t1102 = t152.*t788;
t1103 = t152.*t789;
t1107 = t341.*t641.*2.0;
t1112 = t131.*t788;
t1113 = t131.*t789;
t1114 = t1086.*(-1.0./2.0);
t1115 = t136.*t788;
t1116 = t136.*t789;
t1117 = t137.*t789;
t1118 = t1087.*(-1.0./2.0);
t1127 = t519+t526;
t1128 = t490+t539;
t1129 = t491+t538;
t1144 = t18.*t112.*t789;
t1151 = -t1076;
t1155 = t402.*t641;
t1156 = t403.*t641;
t1167 = t1086./2.0;
t1168 = t1087./2.0;
t1176 = t173.*t788;
t1177 = t174.*t789;
t1180 = t402.*t669;
t1183 = t207.*t788;
t1184 = t184.*t788;
t1185 = t185.*t789;
t1186 = t504+t573;
t1187 = t506+t576;
t1189 = t190.*t789;
t1190 = t503+t559;
t1196 = t18.*t155.*t789;
t1219 = -t14.*(t478-t519);
t1224 = t261.*t788;
t1225 = t261.*t789;
t1226 = t265.*t788;
t1227 = t265.*t789;
t1228 = t266.*t789;
t1230 = t23.*t155.*t788;
t1236 = t26.*t155.*t788;
t1237 = t23.*t158.*t789;
t1238 = t26.*t158.*t789;
t1244 = t14.*t1170;
t1253 = t255.*t788;
t1254 = t256.*t789;
t1262 = -t1214;
t1263 = t402.*t724;
t1264 = t14.*t494.*t641;
t1267 = t18.*t37.*t1070;
t1268 = t12.*t39.*t1070;
t1277 = t256.*t788.*2.0;
t1278 = t255.*t789.*2.0;
t1284 = t8.*t546.*t609;
t1285 = t14.*(t478-t519).*(-1.0./2.0);
t1291 = t363.*t789;
t1292 = t13.*t255.*t789;
t1293 = t339.*t788;
t1294 = t19.*t255.*t789;
t1295 = t330.*t788;
t1296 = t329.*t789;
t1305 = t317.*t789;
t1306 = -t8.*t37.*(t478-t519);
t1307 = t585.*t641;
t1310 = t35.*t39.*t1070;
t1311 = t18.*t61.*t1070;
t1313 = -t8.*t39.*(t478-t519);
t1315 = t38.*t39.*t1070;
t1316 = t18.*t63.*t1070;
t1319 = t329.*t788.*2.0;
t1320 = t330.*t789.*2.0;
t1322 = t115.*t1070;
t1323 = t341.*t788;
t1324 = t341.*t789;
t1325 = t342.*t789;
t1340 = t428.*t788;
t1341 = t13.*t330.*t789;
t1342 = t400.*t789;
t1343 = t19.*t330.*t789;
t1351 = t368.*t789;
t1360 = -t14.*t546.*(t101-t401);
t1366 = t158.*t1070;
t1369 = t402.*t788;
t1370 = t402.*t789;
t1371 = t403.*t789;
t1376 = t582.*(t100-t364);
t1382 = t8.*t37.*(t478-t519).*(-1.0./2.0);
t1384 = t628+t639;
t1386 = t8.*t39.*(t478-t519).*(-1.0./2.0);
t1398 = (t8.*t39.*(t478-t519))./2.0;
t1400 = t468.*t788;
t1401 = t453.*t789;
t1403 = t472.*t789;
t1404 = t473.*t788;
t1405 = t477.*t789;
Y = ft_3({t100,t1000,t1001,t1002,t1003,t1007,t1008,t101,t1015,t1016,t1017,t1018,t1021,t1022,t1027,t1028,t1029,t1030,t1034,t1036,t104,t1041,t1045,t1046,t1047,t1048,t1051,t1052,t1055,t1059,t106,t1062,t1065,t1066,t1068,t1069,t107,t1070,t1071,t1075,t1077,t108,t1082,t1085,t1086,t1087,t1089,t1092,t1093,t1094,t1096,t1097,t1098,t1099,t1104,t1105,t1107,t111,t1112,t1113,t1115,t1116,t1117,t112,t1121,t1122,t1123,t1128,t1129,t113,t1133,t1134,t1135,t1137,t1139,t1140,t1141,t1144,t115,t1150,t1151,t1153,t1154,t1155,t1156,t1164,t1166,t1167,t1168,t1172,t1174,t1175,t1176,t1177,t1179,t1180,t1183,t1184,t1185,t1186,t1187,t1188,t1189,t1190,t1193,t1195,t1196,t1197,t1198,t12,t1203,t1213,t1219,t1222,t1223,t1224,t1225,t1226,t1227,t1229,t1230,t1235,t1236,t1237,t1238,t124,t1242,t1243,t1244,t1245,t1246,t1248,t1253,t1254,t1256,t1257,t1258,t1262,t1263,t1264,t1265,t1267,t1268,t127,t1275,t1276,t1277,t1278,t1279,t128,t1283,t1284,t1285,t1287,t1288,t1291,t1292,t1293,t1294,t1295,t1296,t1297,t1298,t13,t1302,t1305,t1306,t1307,t131,t1310,t1311,t1313,t1315,t1316,t1319,t132,t1320,t1321,t1322,t1323,t1324,t1325,t1330,t1331,t1332,t1333,t1334,t1335,t134,t1340,t1341,t1342,t1343,t1349,t1351,t1352,t1353,t1355,t1358,t136,t1360,t1366,t1368,t1369,t137,t1370,t1371,t1375,t1376,t1378,t138,t1382,t1398,t1399,t14,t1400,t1401,t1403,t1410,t1413,t1414,t1415,t1416,t1417,t1426,t1427,t1431,t1455,t1462,t1463,t1469,t1470,t1485,t1488,t1492,t1494,t1495,t1499,t15,t150,t1500,t1501,t1506,t1511,t1516,t1517,t1518,t1519,t152,t1520,t1521,t1532,t1534,t1535,t1541,t1542,t1547,t1548,t155,t156,t1570,t1574,t1575,t158,t159,t160,t1618,t162,t163,t164,t1640,t165,t1650,t1651,t1652,t1653,t1666,t1669,t1674,t1677,t1699,t1704,t1706,t1709,t171,t1710,t1713,t1714,t1728,t173,t1730,t1733,t1736,t174,t1740,t1741,t175,t1751,t1754,t1755,t1758,t1759,t1769,t177,t1772,t1788,t18,t1804,t1807,t1811,t1812,t1818,t1837,t184,t1840,t185,t1863,t1866,t1868,t187,t1888,t1889,t1890,t1891,t19,t190,t191,t1910,t192,t1930,t1937,t1942,t1955,t196,t1961,t1962,t1965,t1968,t1969,t1973,t1976,t1977,t1984,t1989,t199,t1994,t1d,t1dd,t200,t2008,t201,t2017,t2019,t202,t2037,t2038,t2039,t2044,t2045,t2047,t2048,t2051,t2055,t2056,t206,t2063,t207,t2070,t2074,t2075,t2081,t2085,t2087,t2089,t2090,t2093,t21,t210,t2100,t2101,t2109,t211,t2110,t2113,t2117,t2118,t2123,t213,t2140,t2141,t2142,t2144,t2145,t2147,t215,t2158,t2167,t2168,t2170,t2173,t2174,t219,t2197,t22,t220,t221,t2217,t2218,t2231,t2232,t2254,t226,t2279,t228,t2286,t229,t2298,t23,t2300,t2303,t231,t2311,t2312,t2315,t232,t233,t2334,t2336,t2337,t2338,t234,t2340,t2341,t2342,t2344,t2346,t2348,t235,t2353,t2354,t2357,t2359,t2395,t2398,t2399,t24,t2400,t2401,t243,t2434,t2435,t244,t245,t2467,t247,t2470,t2472,t2473,t248,t2482,t249,t2490,t2495,t2496,t25,t2507,t2508,t2509,t2511,t2527,t2529,t2530,t2540,t255,t2557,t256,t2560,t2565,t258,t26,t2606,t263,t2633,t2634,t2638,t2639,t2642,t2644,t2648,t2659,t266,t268,t2685,t2692,t27,t2708,t2718,t273,t2743,t2744,t2745,t2748,t2749,t276,t2776,t2777,t278,t279,t28,t281,t283,t2839,t2849,t2862,t287,t2876,t288,t289,t2897,t29,t2919,t2956,t2983,t2985,t2987,t2989,t299,t2995,t2996,t2999,t2d,t2dd,t30,t301,t303,t3035,t304,t3046,t308,t3086,t3088,t309,t31,t310,t3122,t3131,t315,t317,t3178,t318,t3183,t319,t320,t321,t325,t3288,t3289,t329,t3291,t3292,t330,t3308,t331,t332,t3321,t333,t3330,t3332,t334,t335,t3388,t339,t3391,t34,t3400,t3401,t3404,t3405,t341,t3415,t342,t3422,t343,t344,t345,t346,t347,t3488,t3496,t35,t3509,t3510,t3516,t3517,t354,t3553,t3557,t3575,t3593,t36,t360,t361,t363,t364,t365,t368,t3683,t3685,t37,t3743,t3746,t375,t38,t383,t384,t39,t3905,t392,t393,t394,t395,t3d,t3dd,t400,t401,t402,t403,t404,t41,t410,t411,t412,t413,t414,t415,t416,t417,t418,t419,t42,t420,t425,t428,t43,t431,t434,t437,t441,t442,t443,t444,t445,t446,t449,t453,t454,t455,t459,t463,t466,t467,t468,t470,t472,t476,t477,t478,t48,t483,t484,t486,t487,t488,t489,t492,t493,t494,t495,t496,t497,t498,t499,t4d,t4dd,t50,t500,t501,t502,t503,t507,t508,t51,t510,t511,t513,t514,t515,t516,t517,t519,t521,t522,t523,t524,t529,t53,t530,t532,t535,t536,t537,t540,t542,t543,t544,t545,t546,t547,t548,t549,t55,t550,t552,t553,t554,t558,t56,t560,t562,t563,t564,t565,t566,t567,t569,t57,t570,t571,t577,t579,t58,t580,t581,t582,t585,t587,t588,t589,t591,t593,t594,t595,t596,t598,t5d,t5dd,t601,t602,t607,t608,t609,t61,t612,t613,t614,t615,t616,t617,t621,t623,t624,t625,t626,t627,t629,t63,t630,t632,t633,t634,t635,t636,t637,t639,t641,t642,t643,t644,t645,t647,t648,t649,t650,t651,t652,t653,t654,t655,t656,t657,t658,t659,t660,t661,t664,t667,t668,t669,t670,t671,t673,t674,t675,t676,t681,t682,t683,t684,t685,t686,t687,t689,t69,t690,t694,t695,t696,t697,t698,t699,t6d,t6dd,t700,t701,t702,t703,t705,t706,t71,t711,t712,t713,t720,t721,t723,t724,t725,t726,t727,t728,t729,t730,t731,t732,t733,t735,t736,t737,t738,t739,t740,t742,t744,t745,t746,t747,t748,t749,t75,t750,t752,t753,t754,t755,t756,t757,t759,t760,t761,t762,t763,t764,t765,t766,t767,t768,t769,t770,t772,t774,t775,t776,t778,t780,t781,t782,t783,t784,t785,t786,t788,t789,t792,t793,t794,t796,t797,t799,t8,t800,t801,t802,t803,t804,t805,t806,t807,t810,t814,t815,t816,t82,t820,t821,t822,t823,t824,t825,t826,t827,t828,t829,t830,t831,t832,t833,t835,t836,t838,t839,t840,t841,t842,t843,t844,t845,t846,t847,t849,t850,t852,t853,t854,t855,t859,t861,t865,t866,t867,t868,t869,t870,t871,t872,t873,t874,t875,t877,t879,t88,t880,t881,t883,t884,t885,t887,t890,t891,t892,t893,t894,t896,t897,t898,t899,t9,t900,t901,t902,t903,t904,t906,t907,t908,t909,t910,t911,t912,t913,t914,t915,t916,t917,t919,t921,t922,t923,t925,t927,t928,t931,t932,t937,t938,t939,t943,t944,t945,t948,t952,t954,t955,t956,t957,t958,t959,t960,t961,t962,t963,t964,t965,t966,t968,t969,t970,t971,t972,t973,t974,t975,t978,t979,t980,t981,t984,t985,t986,t987,t988,t989,t991,t992,t998,t999});
end
function Y = ft_3(ct)
t100 = ct{1};
t1000 = ct{2};
t1001 = ct{3};
t1002 = ct{4};
t1003 = ct{5};
t1007 = ct{6};
t1008 = ct{7};
t101 = ct{8};
t1015 = ct{9};
t1016 = ct{10};
t1017 = ct{11};
t1018 = ct{12};
t1021 = ct{13};
t1022 = ct{14};
t1027 = ct{15};
t1028 = ct{16};
t1029 = ct{17};
t1030 = ct{18};
t1034 = ct{19};
t1036 = ct{20};
t104 = ct{21};
t1041 = ct{22};
t1045 = ct{23};
t1046 = ct{24};
t1047 = ct{25};
t1048 = ct{26};
t1051 = ct{27};
t1052 = ct{28};
t1055 = ct{29};
t1059 = ct{30};
t106 = ct{31};
t1062 = ct{32};
t1065 = ct{33};
t1066 = ct{34};
t1068 = ct{35};
t1069 = ct{36};
t107 = ct{37};
t1070 = ct{38};
t1071 = ct{39};
t1075 = ct{40};
t1077 = ct{41};
t108 = ct{42};
t1082 = ct{43};
t1085 = ct{44};
t1086 = ct{45};
t1087 = ct{46};
t1089 = ct{47};
t1092 = ct{48};
t1093 = ct{49};
t1094 = ct{50};
t1096 = ct{51};
t1097 = ct{52};
t1098 = ct{53};
t1099 = ct{54};
t1104 = ct{55};
t1105 = ct{56};
t1107 = ct{57};
t111 = ct{58};
t1112 = ct{59};
t1113 = ct{60};
t1115 = ct{61};
t1116 = ct{62};
t1117 = ct{63};
t112 = ct{64};
t1121 = ct{65};
t1122 = ct{66};
t1123 = ct{67};
t1128 = ct{68};
t1129 = ct{69};
t113 = ct{70};
t1133 = ct{71};
t1134 = ct{72};
t1135 = ct{73};
t1137 = ct{74};
t1139 = ct{75};
t1140 = ct{76};
t1141 = ct{77};
t1144 = ct{78};
t115 = ct{79};
t1150 = ct{80};
t1151 = ct{81};
t1153 = ct{82};
t1154 = ct{83};
t1155 = ct{84};
t1156 = ct{85};
t1164 = ct{86};
t1166 = ct{87};
t1167 = ct{88};
t1168 = ct{89};
t1172 = ct{90};
t1174 = ct{91};
t1175 = ct{92};
t1176 = ct{93};
t1177 = ct{94};
t1179 = ct{95};
t1180 = ct{96};
t1183 = ct{97};
t1184 = ct{98};
t1185 = ct{99};
t1186 = ct{100};
t1187 = ct{101};
t1188 = ct{102};
t1189 = ct{103};
t1190 = ct{104};
t1193 = ct{105};
t1195 = ct{106};
t1196 = ct{107};
t1197 = ct{108};
t1198 = ct{109};
t12 = ct{110};
t1203 = ct{111};
t1213 = ct{112};
t1219 = ct{113};
t1222 = ct{114};
t1223 = ct{115};
t1224 = ct{116};
t1225 = ct{117};
t1226 = ct{118};
t1227 = ct{119};
t1229 = ct{120};
t1230 = ct{121};
t1235 = ct{122};
t1236 = ct{123};
t1237 = ct{124};
t1238 = ct{125};
t124 = ct{126};
t1242 = ct{127};
t1243 = ct{128};
t1244 = ct{129};
t1245 = ct{130};
t1246 = ct{131};
t1248 = ct{132};
t1253 = ct{133};
t1254 = ct{134};
t1256 = ct{135};
t1257 = ct{136};
t1258 = ct{137};
t1262 = ct{138};
t1263 = ct{139};
t1264 = ct{140};
t1265 = ct{141};
t1267 = ct{142};
t1268 = ct{143};
t127 = ct{144};
t1275 = ct{145};
t1276 = ct{146};
t1277 = ct{147};
t1278 = ct{148};
t1279 = ct{149};
t128 = ct{150};
t1283 = ct{151};
t1284 = ct{152};
t1285 = ct{153};
t1287 = ct{154};
t1288 = ct{155};
t1291 = ct{156};
t1292 = ct{157};
t1293 = ct{158};
t1294 = ct{159};
t1295 = ct{160};
t1296 = ct{161};
t1297 = ct{162};
t1298 = ct{163};
t13 = ct{164};
t1302 = ct{165};
t1305 = ct{166};
t1306 = ct{167};
t1307 = ct{168};
t131 = ct{169};
t1310 = ct{170};
t1311 = ct{171};
t1313 = ct{172};
t1315 = ct{173};
t1316 = ct{174};
t1319 = ct{175};
t132 = ct{176};
t1320 = ct{177};
t1321 = ct{178};
t1322 = ct{179};
t1323 = ct{180};
t1324 = ct{181};
t1325 = ct{182};
t1330 = ct{183};
t1331 = ct{184};
t1332 = ct{185};
t1333 = ct{186};
t1334 = ct{187};
t1335 = ct{188};
t134 = ct{189};
t1340 = ct{190};
t1341 = ct{191};
t1342 = ct{192};
t1343 = ct{193};
t1349 = ct{194};
t1351 = ct{195};
t1352 = ct{196};
t1353 = ct{197};
t1355 = ct{198};
t1358 = ct{199};
t136 = ct{200};
t1360 = ct{201};
t1366 = ct{202};
t1368 = ct{203};
t1369 = ct{204};
t137 = ct{205};
t1370 = ct{206};
t1371 = ct{207};
t1375 = ct{208};
t1376 = ct{209};
t1378 = ct{210};
t138 = ct{211};
t1382 = ct{212};
t1398 = ct{213};
t1399 = ct{214};
t14 = ct{215};
t1400 = ct{216};
t1401 = ct{217};
t1403 = ct{218};
t1410 = ct{219};
t1413 = ct{220};
t1414 = ct{221};
t1415 = ct{222};
t1416 = ct{223};
t1417 = ct{224};
t1426 = ct{225};
t1427 = ct{226};
t1431 = ct{227};
t1455 = ct{228};
t1462 = ct{229};
t1463 = ct{230};
t1469 = ct{231};
t1470 = ct{232};
t1485 = ct{233};
t1488 = ct{234};
t1492 = ct{235};
t1494 = ct{236};
t1495 = ct{237};
t1499 = ct{238};
t15 = ct{239};
t150 = ct{240};
t1500 = ct{241};
t1501 = ct{242};
t1506 = ct{243};
t1511 = ct{244};
t1516 = ct{245};
t1517 = ct{246};
t1518 = ct{247};
t1519 = ct{248};
t152 = ct{249};
t1520 = ct{250};
t1521 = ct{251};
t1532 = ct{252};
t1534 = ct{253};
t1535 = ct{254};
t1541 = ct{255};
t1542 = ct{256};
t1547 = ct{257};
t1548 = ct{258};
t155 = ct{259};
t156 = ct{260};
t1570 = ct{261};
t1574 = ct{262};
t1575 = ct{263};
t158 = ct{264};
t159 = ct{265};
t160 = ct{266};
t1618 = ct{267};
t162 = ct{268};
t163 = ct{269};
t164 = ct{270};
t1640 = ct{271};
t165 = ct{272};
t1650 = ct{273};
t1651 = ct{274};
t1652 = ct{275};
t1653 = ct{276};
t1666 = ct{277};
t1669 = ct{278};
t1674 = ct{279};
t1677 = ct{280};
t1699 = ct{281};
t1704 = ct{282};
t1706 = ct{283};
t1709 = ct{284};
t171 = ct{285};
t1710 = ct{286};
t1713 = ct{287};
t1714 = ct{288};
t1728 = ct{289};
t173 = ct{290};
t1730 = ct{291};
t1733 = ct{292};
t1736 = ct{293};
t174 = ct{294};
t1740 = ct{295};
t1741 = ct{296};
t175 = ct{297};
t1751 = ct{298};
t1754 = ct{299};
t1755 = ct{300};
t1758 = ct{301};
t1759 = ct{302};
t1769 = ct{303};
t177 = ct{304};
t1772 = ct{305};
t1788 = ct{306};
t18 = ct{307};
t1804 = ct{308};
t1807 = ct{309};
t1811 = ct{310};
t1812 = ct{311};
t1818 = ct{312};
t1837 = ct{313};
t184 = ct{314};
t1840 = ct{315};
t185 = ct{316};
t1863 = ct{317};
t1866 = ct{318};
t1868 = ct{319};
t187 = ct{320};
t1888 = ct{321};
t1889 = ct{322};
t1890 = ct{323};
t1891 = ct{324};
t19 = ct{325};
t190 = ct{326};
t191 = ct{327};
t1910 = ct{328};
t192 = ct{329};
t1930 = ct{330};
t1937 = ct{331};
t1942 = ct{332};
t1955 = ct{333};
t196 = ct{334};
t1961 = ct{335};
t1962 = ct{336};
t1965 = ct{337};
t1968 = ct{338};
t1969 = ct{339};
t1973 = ct{340};
t1976 = ct{341};
t1977 = ct{342};
t1984 = ct{343};
t1989 = ct{344};
t199 = ct{345};
t1994 = ct{346};
t1d = ct{347};
t1dd = ct{348};
t200 = ct{349};
t2008 = ct{350};
t201 = ct{351};
t2017 = ct{352};
t2019 = ct{353};
t202 = ct{354};
t2037 = ct{355};
t2038 = ct{356};
t2039 = ct{357};
t2044 = ct{358};
t2045 = ct{359};
t2047 = ct{360};
t2048 = ct{361};
t2051 = ct{362};
t2055 = ct{363};
t2056 = ct{364};
t206 = ct{365};
t2063 = ct{366};
t207 = ct{367};
t2070 = ct{368};
t2074 = ct{369};
t2075 = ct{370};
t2081 = ct{371};
t2085 = ct{372};
t2087 = ct{373};
t2089 = ct{374};
t2090 = ct{375};
t2093 = ct{376};
t21 = ct{377};
t210 = ct{378};
t2100 = ct{379};
t2101 = ct{380};
t2109 = ct{381};
t211 = ct{382};
t2110 = ct{383};
t2113 = ct{384};
t2117 = ct{385};
t2118 = ct{386};
t2123 = ct{387};
t213 = ct{388};
t2140 = ct{389};
t2141 = ct{390};
t2142 = ct{391};
t2144 = ct{392};
t2145 = ct{393};
t2147 = ct{394};
t215 = ct{395};
t2158 = ct{396};
t2167 = ct{397};
t2168 = ct{398};
t2170 = ct{399};
t2173 = ct{400};
t2174 = ct{401};
t219 = ct{402};
t2197 = ct{403};
t22 = ct{404};
t220 = ct{405};
t221 = ct{406};
t2217 = ct{407};
t2218 = ct{408};
t2231 = ct{409};
t2232 = ct{410};
t2254 = ct{411};
t226 = ct{412};
t2279 = ct{413};
t228 = ct{414};
t2286 = ct{415};
t229 = ct{416};
t2298 = ct{417};
t23 = ct{418};
t2300 = ct{419};
t2303 = ct{420};
t231 = ct{421};
t2311 = ct{422};
t2312 = ct{423};
t2315 = ct{424};
t232 = ct{425};
t233 = ct{426};
t2334 = ct{427};
t2336 = ct{428};
t2337 = ct{429};
t2338 = ct{430};
t234 = ct{431};
t2340 = ct{432};
t2341 = ct{433};
t2342 = ct{434};
t2344 = ct{435};
t2346 = ct{436};
t2348 = ct{437};
t235 = ct{438};
t2353 = ct{439};
t2354 = ct{440};
t2357 = ct{441};
t2359 = ct{442};
t2395 = ct{443};
t2398 = ct{444};
t2399 = ct{445};
t24 = ct{446};
t2400 = ct{447};
t2401 = ct{448};
t243 = ct{449};
t2434 = ct{450};
t2435 = ct{451};
t244 = ct{452};
t245 = ct{453};
t2467 = ct{454};
t247 = ct{455};
t2470 = ct{456};
t2472 = ct{457};
t2473 = ct{458};
t248 = ct{459};
t2482 = ct{460};
t249 = ct{461};
t2490 = ct{462};
t2495 = ct{463};
t2496 = ct{464};
t25 = ct{465};
t2507 = ct{466};
t2508 = ct{467};
t2509 = ct{468};
t2511 = ct{469};
t2527 = ct{470};
t2529 = ct{471};
t2530 = ct{472};
t2540 = ct{473};
t255 = ct{474};
t2557 = ct{475};
t256 = ct{476};
t2560 = ct{477};
t2565 = ct{478};
t258 = ct{479};
t26 = ct{480};
t2606 = ct{481};
t263 = ct{482};
t2633 = ct{483};
t2634 = ct{484};
t2638 = ct{485};
t2639 = ct{486};
t2642 = ct{487};
t2644 = ct{488};
t2648 = ct{489};
t2659 = ct{490};
t266 = ct{491};
t268 = ct{492};
t2685 = ct{493};
t2692 = ct{494};
t27 = ct{495};
t2708 = ct{496};
t2718 = ct{497};
t273 = ct{498};
t2743 = ct{499};
t2744 = ct{500};
t2745 = ct{501};
t2748 = ct{502};
t2749 = ct{503};
t276 = ct{504};
t2776 = ct{505};
t2777 = ct{506};
t278 = ct{507};
t279 = ct{508};
t28 = ct{509};
t281 = ct{510};
t283 = ct{511};
t2839 = ct{512};
t2849 = ct{513};
t2862 = ct{514};
t287 = ct{515};
t2876 = ct{516};
t288 = ct{517};
t289 = ct{518};
t2897 = ct{519};
t29 = ct{520};
t2919 = ct{521};
t2956 = ct{522};
t2983 = ct{523};
t2985 = ct{524};
t2987 = ct{525};
t2989 = ct{526};
t299 = ct{527};
t2995 = ct{528};
t2996 = ct{529};
t2999 = ct{530};
t2d = ct{531};
t2dd = ct{532};
t30 = ct{533};
t301 = ct{534};
t303 = ct{535};
t3035 = ct{536};
t304 = ct{537};
t3046 = ct{538};
t308 = ct{539};
t3086 = ct{540};
t3088 = ct{541};
t309 = ct{542};
t31 = ct{543};
t310 = ct{544};
t3122 = ct{545};
t3131 = ct{546};
t315 = ct{547};
t317 = ct{548};
t3178 = ct{549};
t318 = ct{550};
t3183 = ct{551};
t319 = ct{552};
t320 = ct{553};
t321 = ct{554};
t325 = ct{555};
t3288 = ct{556};
t3289 = ct{557};
t329 = ct{558};
t3291 = ct{559};
t3292 = ct{560};
t330 = ct{561};
t3308 = ct{562};
t331 = ct{563};
t332 = ct{564};
t3321 = ct{565};
t333 = ct{566};
t3330 = ct{567};
t3332 = ct{568};
t334 = ct{569};
t335 = ct{570};
t3388 = ct{571};
t339 = ct{572};
t3391 = ct{573};
t34 = ct{574};
t3400 = ct{575};
t3401 = ct{576};
t3404 = ct{577};
t3405 = ct{578};
t341 = ct{579};
t3415 = ct{580};
t342 = ct{581};
t3422 = ct{582};
t343 = ct{583};
t344 = ct{584};
t345 = ct{585};
t346 = ct{586};
t347 = ct{587};
t3488 = ct{588};
t3496 = ct{589};
t35 = ct{590};
t3509 = ct{591};
t3510 = ct{592};
t3516 = ct{593};
t3517 = ct{594};
t354 = ct{595};
t3553 = ct{596};
t3557 = ct{597};
t3575 = ct{598};
t3593 = ct{599};
t36 = ct{600};
t360 = ct{601};
t361 = ct{602};
t363 = ct{603};
t364 = ct{604};
t365 = ct{605};
t368 = ct{606};
t3683 = ct{607};
t3685 = ct{608};
t37 = ct{609};
t3743 = ct{610};
t3746 = ct{611};
t375 = ct{612};
t38 = ct{613};
t383 = ct{614};
t384 = ct{615};
t39 = ct{616};
t3905 = ct{617};
t392 = ct{618};
t393 = ct{619};
t394 = ct{620};
t395 = ct{621};
t3d = ct{622};
t3dd = ct{623};
t400 = ct{624};
t401 = ct{625};
t402 = ct{626};
t403 = ct{627};
t404 = ct{628};
t41 = ct{629};
t410 = ct{630};
t411 = ct{631};
t412 = ct{632};
t413 = ct{633};
t414 = ct{634};
t415 = ct{635};
t416 = ct{636};
t417 = ct{637};
t418 = ct{638};
t419 = ct{639};
t42 = ct{640};
t420 = ct{641};
t425 = ct{642};
t428 = ct{643};
t43 = ct{644};
t431 = ct{645};
t434 = ct{646};
t437 = ct{647};
t441 = ct{648};
t442 = ct{649};
t443 = ct{650};
t444 = ct{651};
t445 = ct{652};
t446 = ct{653};
t449 = ct{654};
t453 = ct{655};
t454 = ct{656};
t455 = ct{657};
t459 = ct{658};
t463 = ct{659};
t466 = ct{660};
t467 = ct{661};
t468 = ct{662};
t470 = ct{663};
t472 = ct{664};
t476 = ct{665};
t477 = ct{666};
t478 = ct{667};
t48 = ct{668};
t483 = ct{669};
t484 = ct{670};
t486 = ct{671};
t487 = ct{672};
t488 = ct{673};
t489 = ct{674};
t492 = ct{675};
t493 = ct{676};
t494 = ct{677};
t495 = ct{678};
t496 = ct{679};
t497 = ct{680};
t498 = ct{681};
t499 = ct{682};
t4d = ct{683};
t4dd = ct{684};
t50 = ct{685};
t500 = ct{686};
t501 = ct{687};
t502 = ct{688};
t503 = ct{689};
t507 = ct{690};
t508 = ct{691};
t51 = ct{692};
t510 = ct{693};
t511 = ct{694};
t513 = ct{695};
t514 = ct{696};
t515 = ct{697};
t516 = ct{698};
t517 = ct{699};
t519 = ct{700};
t521 = ct{701};
t522 = ct{702};
t523 = ct{703};
t524 = ct{704};
t529 = ct{705};
t53 = ct{706};
t530 = ct{707};
t532 = ct{708};
t535 = ct{709};
t536 = ct{710};
t537 = ct{711};
t540 = ct{712};
t542 = ct{713};
t543 = ct{714};
t544 = ct{715};
t545 = ct{716};
t546 = ct{717};
t547 = ct{718};
t548 = ct{719};
t549 = ct{720};
t55 = ct{721};
t550 = ct{722};
t552 = ct{723};
t553 = ct{724};
t554 = ct{725};
t558 = ct{726};
t56 = ct{727};
t560 = ct{728};
t562 = ct{729};
t563 = ct{730};
t564 = ct{731};
t565 = ct{732};
t566 = ct{733};
t567 = ct{734};
t569 = ct{735};
t57 = ct{736};
t570 = ct{737};
t571 = ct{738};
t577 = ct{739};
t579 = ct{740};
t58 = ct{741};
t580 = ct{742};
t581 = ct{743};
t582 = ct{744};
t585 = ct{745};
t587 = ct{746};
t588 = ct{747};
t589 = ct{748};
t591 = ct{749};
t593 = ct{750};
t594 = ct{751};
t595 = ct{752};
t596 = ct{753};
t598 = ct{754};
t5d = ct{755};
t5dd = ct{756};
t601 = ct{757};
t602 = ct{758};
t607 = ct{759};
t608 = ct{760};
t609 = ct{761};
t61 = ct{762};
t612 = ct{763};
t613 = ct{764};
t614 = ct{765};
t615 = ct{766};
t616 = ct{767};
t617 = ct{768};
t621 = ct{769};
t623 = ct{770};
t624 = ct{771};
t625 = ct{772};
t626 = ct{773};
t627 = ct{774};
t629 = ct{775};
t63 = ct{776};
t630 = ct{777};
t632 = ct{778};
t633 = ct{779};
t634 = ct{780};
t635 = ct{781};
t636 = ct{782};
t637 = ct{783};
t639 = ct{784};
t641 = ct{785};
t642 = ct{786};
t643 = ct{787};
t644 = ct{788};
t645 = ct{789};
t647 = ct{790};
t648 = ct{791};
t649 = ct{792};
t650 = ct{793};
t651 = ct{794};
t652 = ct{795};
t653 = ct{796};
t654 = ct{797};
t655 = ct{798};
t656 = ct{799};
t657 = ct{800};
t658 = ct{801};
t659 = ct{802};
t660 = ct{803};
t661 = ct{804};
t664 = ct{805};
t667 = ct{806};
t668 = ct{807};
t669 = ct{808};
t670 = ct{809};
t671 = ct{810};
t673 = ct{811};
t674 = ct{812};
t675 = ct{813};
t676 = ct{814};
t681 = ct{815};
t682 = ct{816};
t683 = ct{817};
t684 = ct{818};
t685 = ct{819};
t686 = ct{820};
t687 = ct{821};
t689 = ct{822};
t69 = ct{823};
t690 = ct{824};
t694 = ct{825};
t695 = ct{826};
t696 = ct{827};
t697 = ct{828};
t698 = ct{829};
t699 = ct{830};
t6d = ct{831};
t6dd = ct{832};
t700 = ct{833};
t701 = ct{834};
t702 = ct{835};
t703 = ct{836};
t705 = ct{837};
t706 = ct{838};
t71 = ct{839};
t711 = ct{840};
t712 = ct{841};
t713 = ct{842};
t720 = ct{843};
t721 = ct{844};
t723 = ct{845};
t724 = ct{846};
t725 = ct{847};
t726 = ct{848};
t727 = ct{849};
t728 = ct{850};
t729 = ct{851};
t730 = ct{852};
t731 = ct{853};
t732 = ct{854};
t733 = ct{855};
t735 = ct{856};
t736 = ct{857};
t737 = ct{858};
t738 = ct{859};
t739 = ct{860};
t740 = ct{861};
t742 = ct{862};
t744 = ct{863};
t745 = ct{864};
t746 = ct{865};
t747 = ct{866};
t748 = ct{867};
t749 = ct{868};
t75 = ct{869};
t750 = ct{870};
t752 = ct{871};
t753 = ct{872};
t754 = ct{873};
t755 = ct{874};
t756 = ct{875};
t757 = ct{876};
t759 = ct{877};
t760 = ct{878};
t761 = ct{879};
t762 = ct{880};
t763 = ct{881};
t764 = ct{882};
t765 = ct{883};
t766 = ct{884};
t767 = ct{885};
t768 = ct{886};
t769 = ct{887};
t770 = ct{888};
t772 = ct{889};
t774 = ct{890};
t775 = ct{891};
t776 = ct{892};
t778 = ct{893};
t780 = ct{894};
t781 = ct{895};
t782 = ct{896};
t783 = ct{897};
t784 = ct{898};
t785 = ct{899};
t786 = ct{900};
t788 = ct{901};
t789 = ct{902};
t792 = ct{903};
t793 = ct{904};
t794 = ct{905};
t796 = ct{906};
t797 = ct{907};
t799 = ct{908};
t8 = ct{909};
t800 = ct{910};
t801 = ct{911};
t802 = ct{912};
t803 = ct{913};
t804 = ct{914};
t805 = ct{915};
t806 = ct{916};
t807 = ct{917};
t810 = ct{918};
t814 = ct{919};
t815 = ct{920};
t816 = ct{921};
t82 = ct{922};
t820 = ct{923};
t821 = ct{924};
t822 = ct{925};
t823 = ct{926};
t824 = ct{927};
t825 = ct{928};
t826 = ct{929};
t827 = ct{930};
t828 = ct{931};
t829 = ct{932};
t830 = ct{933};
t831 = ct{934};
t832 = ct{935};
t833 = ct{936};
t835 = ct{937};
t836 = ct{938};
t838 = ct{939};
t839 = ct{940};
t840 = ct{941};
t841 = ct{942};
t842 = ct{943};
t843 = ct{944};
t844 = ct{945};
t845 = ct{946};
t846 = ct{947};
t847 = ct{948};
t849 = ct{949};
t850 = ct{950};
t852 = ct{951};
t853 = ct{952};
t854 = ct{953};
t855 = ct{954};
t859 = ct{955};
t861 = ct{956};
t865 = ct{957};
t866 = ct{958};
t867 = ct{959};
t868 = ct{960};
t869 = ct{961};
t870 = ct{962};
t871 = ct{963};
t872 = ct{964};
t873 = ct{965};
t874 = ct{966};
t875 = ct{967};
t877 = ct{968};
t879 = ct{969};
t88 = ct{970};
t880 = ct{971};
t881 = ct{972};
t883 = ct{973};
t884 = ct{974};
t885 = ct{975};
t887 = ct{976};
t890 = ct{977};
t891 = ct{978};
t892 = ct{979};
t893 = ct{980};
t894 = ct{981};
t896 = ct{982};
t897 = ct{983};
t898 = ct{984};
t899 = ct{985};
t9 = ct{986};
t900 = ct{987};
t901 = ct{988};
t902 = ct{989};
t903 = ct{990};
t904 = ct{991};
t906 = ct{992};
t907 = ct{993};
t908 = ct{994};
t909 = ct{995};
t910 = ct{996};
t911 = ct{997};
t912 = ct{998};
t913 = ct{999};
t914 = ct{1000};
t915 = ct{1001};
t916 = ct{1002};
t917 = ct{1003};
t919 = ct{1004};
t921 = ct{1005};
t922 = ct{1006};
t923 = ct{1007};
t925 = ct{1008};
t927 = ct{1009};
t928 = ct{1010};
t931 = ct{1011};
t932 = ct{1012};
t937 = ct{1013};
t938 = ct{1014};
t939 = ct{1015};
t943 = ct{1016};
t944 = ct{1017};
t945 = ct{1018};
t948 = ct{1019};
t952 = ct{1020};
t954 = ct{1021};
t955 = ct{1022};
t956 = ct{1023};
t957 = ct{1024};
t958 = ct{1025};
t959 = ct{1026};
t960 = ct{1027};
t961 = ct{1028};
t962 = ct{1029};
t963 = ct{1030};
t964 = ct{1031};
t965 = ct{1032};
t966 = ct{1033};
t968 = ct{1034};
t969 = ct{1035};
t970 = ct{1036};
t971 = ct{1037};
t972 = ct{1038};
t973 = ct{1039};
t974 = ct{1040};
t975 = ct{1041};
t978 = ct{1042};
t979 = ct{1043};
t980 = ct{1044};
t981 = ct{1045};
t984 = ct{1046};
t985 = ct{1047};
t986 = ct{1048};
t987 = ct{1049};
t988 = ct{1050};
t989 = ct{1051};
t991 = ct{1052};
t992 = ct{1053};
t998 = ct{1054};
t999 = ct{1055};
t1406 = t459.*t789;
t1418 = t14.*t546.*(t101-t401).*(-1.0./2.0);
t1419 = t173+t516+t523;
t1420 = t174+t514+t524;
t1424 = t192+t287+t288+t289;
t1425 = t28.*t37.*t39.*t1070;
t1433 = t449+t846;
t1434 = t507.*t789;
t1435 = t499.*t789;
t1439 = t38.*t437.*t789;
t1440 = t513.*t788;
t1441 = t514.*t789;
t1442 = t516.*t788;
t1443 = t523.*t788;
t1444 = t524.*t789;
t1445 = t502.*t789;
t1452 = t234+t510+t521;
t1454 = t235+t511+t517;
t1458 = t536.*t789;
t1468 = t256.*t1070;
t1471 = t35.*t484.*t789;
t1482 = t577.*t789;
t1490 = t363.*t1070;
t1491 = t13.*t255.*t1070;
t1493 = t19.*t255.*t1070;
t1497 = t329.*t1070;
t1502 = t669+t724;
t1504 = t341.*t1070;
t1505 = t342.*t1070;
t1522 = t609.*t788;
t1523 = t609.*t789;
t1527 = t13.*t330.*t1070;
t1530 = t400.*t1070;
t1531 = t19.*t330.*t1070;
t1536 = t402.*t1070;
t1537 = t403.*t1070;
t1544 = -t788.*(t100-t364);
t1545 = -t789.*(t100-t364);
t1551 = t641.*t788;
t1552 = t641.*t789;
t1553 = t266+t560+t577;
t1583 = t453.*t1070;
t1584 = t472.*t1070;
t1585 = t459.*t1070;
t1591 = t788.*(t100-t364);
t1592 = -t788.*(t101-t401);
t1593 = -t789.*(t101-t401);
t1627 = t507.*t1070;
t1628 = t499.*t1070;
t1629 = t38.*t437.*t1070;
t1630 = t515.*t1070;
t1631 = t502.*t1070;
t1636 = t1574./2.0;
t1637 = t788.*(t101-t401);
t1659 = t730+t760;
t1667 = t35.*t484.*t1070;
t1678 = t18.*t39.*t1532;
t1679 = t1640.*t5dd;
t1680 = t18.*t39.*t1535;
t1701 = t735+t816;
t1703 = t37.*t1575;
t1705 = t39.*t1575;
t1711 = t747+t800;
t1712 = t748+t801;
t1723 = t609.*t1070;
t1734 = t744+t847;
t1750 = t14.*t1704;
t1753 = t14.*t1706;
t1757 = -t1706;
t1768 = t8.*t1728;
t1770 = -t1070.*(t100-t364);
t1771 = t8.*t1730;
t1773 = t641.*t1070;
t1775 = t14.*t1699;
t1780 = t784+t893;
t1801 = -t1070.*(t101-t401);
t1817 = t822+t916;
t1831 = t821+t914;
t1834 = t255.*t1535;
t1839 = t1812.*t1d;
t1845 = t255.*t1532;
t1846 = t8.*t37.*t1699;
t1847 = t1804.*t1d;
t1848 = t8.*t39.*t1699;
t1874 = t872+t903;
t1875 = t875+t906;
t1886 = t330.*t1535;
t1905 = t35.*t39.*t1699;
t1907 = t330.*t1532;
t1908 = t881+t948;
t1916 = t341.*t1532;
t1925 = t341.*t1535;
t1944 = t1866./2.0;
t1946 = t778+t1085;
t1963 = t402.*t1532;
t1971 = t402.*t1535;
t1988 = t18.*t39.*t1811;
t1995 = -t1968;
t1999 = -t1973;
t2011 = t14.*t1942;
t2025 = t8.*t1955;
t2046 = t841+t1150;
t2049 = t14.*t1989;
t2052 = t8.*t1994;
t2076 = -t1d.*(t797-t1188);
t2086 = t330.*t1699;
t2112 = t1d.*(t797-t1188);
t2116 = t958+t1154;
t2119 = -t2089;
t2120 = t184+t207+t463+t508+t513;
t2122 = t2075./2.0;
t2124 = t185+t190+t466+t507+t515;
t2127 = t8.*t39.*t1989;
t2128 = t2085./2.0;
t2131 = -t14.*(t952-t1028);
t2132 = t609.*t1532;
t2133 = t14.*t39.*t1994;
t2135 = t609.*t1535;
t2136 = t2089./2.0;
t2149 = t255.*t1811;
t2150 = t641.*t1535;
t2155 = -t2144;
t2156 = -t2145;
t2159 = -t1532.*(t100-t364);
t2160 = t641.*t1532;
t2162 = -t1535.*(t100-t364);
t2169 = t845+t1349;
t2175 = t14.*(t952-t1028).*(-1.0./2.0);
t2178 = (t14.*t687.*t1399)./2.0;
t2179 = t330.*t1811;
t2183 = -t1535.*(t101-t401);
t2184 = t341.*t1811;
t2189 = t1027+t1197;
t2190 = t1104+t1105;
t2194 = (t14.*(t952-t1028))./2.0;
t2196 = -t1532.*(t101-t401);
t2206 = t8.*t687.*(t441-t846).*(-1.0./2.0);
t2207 = -t8.*t39.*(t952-t1028);
t2210 = t402.*t1811;
t2227 = t14.*t2170;
t2233 = t546+t726+t871;
t2234 = t8.*t2197;
t2267 = t8.*t39.*(t952-t1028).*(-1.0./2.0);
t2270 = t1175+t1243;
t2281 = t211+t278+t281+t621+t629;
t2302 = -t2254;
t2318 = -t2303;
t2345 = -t8.*(-t537+t759+t12.*t39.*(t101-t401));
t2347 = -t2312;
t2371 = t1256+t1275;
t2372 = t1257+t1276;
t2374 = t1258+t1279;
t2383 = t609.*t1811;
t2388 = t8.*(-t537+t759+t12.*t39.*(t101-t401)).*(-1.0./2.0);
t2393 = t2353./2.0;
t2397 = -t330.*(t952-t1028);
t2422 = -t1811.*(t100-t364);
t2425 = t641.*t1811;
t2438 = (t14.*t1036.*t1399)./2.0;
t2453 = t330.*(t952-t1028).*(-1.0./2.0);
t2454 = t1811.*(t100-t364);
t2456 = -t1811.*(t101-t401);
t2458 = t255.*t2158;
t2469 = t171+t273+t335+t1575;
t2474 = -t2435;
t2478 = t8.*t1036.*(t441-t846).*(-1.0./2.0);
t2484 = t1811.*(t101-t401);
t2485 = t330.*t2158;
t2505 = -t2472;
t2519 = t8.*t2470;
t2537 = t925+t1704;
t2539 = t14.*t2482;
t2556 = -t2527;
t2572 = -t2540;
t2576 = t2527./2.0;
t2577 = -t2557;
t2593 = (t14.*t1302.*t1399)./2.0;
t2619 = t8.*t1302.*(t441-t846).*(-1.0./2.0);
t2630 = (t8.*t1302.*(t441-t846))./2.0;
t2655 = t160+t2470;
t2658 = t127+t2482;
t2662 = t8.*t2633;
t2663 = t8.*t2634;
t2666 = t1455+t1469;
t2671 = t14.*t2638;
t2672 = t14.*t2639;
t2687 = t14.*t2659;
t2706 = t2692.*t1d;
t2714 = t2685.*t1d;
t2719 = t1488+t1511;
t2730 = -t2708;
t2746 = -t2718;
t2747 = t2708./2.0;
t2755 = t2718./2.0;
t2771 = t39.*t213.*t2507;
t2772 = t34.*t39.*t2507.*2.8925e-2;
t2775 = -t2748;
t2778 = -t39.*t219.*(t859-t1704);
t2779 = t36.*t39.*(t859-t1704).*(-2.8925e-2);
t2780 = t2745./2.0;
t2790 = t2748./2.0;
t2796 = t1541+t1548;
t2798 = t36.*t39.*(t859-t1704).*2.8925e-2;
t2799 = -t14.*(t582+t616-t761+t18.*t37.*(t100-t364));
t2813 = t1542+t1570;
t2852 = t14.*(t582+t616-t761+t18.*t37.*(t100-t364)).*(-1.0./2.0);
t2871 = (t14.*(t582+t616-t761+t18.*t37.*(t100-t364)))./2.0;
t2889 = -t8.*t39.*(t582+t616-t761+t18.*t37.*(t100-t364));
t2915 = t2862./2.0;
t2927 = t8.*t39.*(t582+t616-t761+t18.*t37.*(t100-t364));
t2929 = t2876./2.0;
t2937 = t39.*t213.*t2659;
t2938 = t34.*t39.*t2659.*2.8925e-2;
t2953 = t34.*t39.*t2659.*(-5.785e-2);
t3007 = -t2987;
t3012 = t2983./2.0;
t3013 = t2985./2.0;
t3014 = t2987./2.0;
t3018 = t2995./2.0;
t3028 = -t330.*(t582+t616-t761+t18.*t37.*(t100-t364));
t3032 = t8.*t687.*t2507;
t3034 = t571+t2659;
t3043 = -t14.*t687.*(t859-t1704);
t3045 = t8.*t703.*t2507;
t3053 = -t14.*t703.*(t859-t1704);
t3059 = t330.*(t582+t616-t761+t18.*t37.*(t100-t364)).*(-1.0./2.0);
t3060 = (t723.*t2507)./2.0;
t3069 = -t3046;
t3072 = t706.*(t859-t1704).*(-1.0./2.0);
t3073 = t3035./2.0;
t3077 = t939+t2434;
t3078 = t14.*t703.*(t859-t1704);
t3080 = t3046./2.0;
t3083 = t1736+t1788;
t3129 = t3086./2.0;
t3130 = t3088./2.0;
t3148 = -t3131;
t3160 = t8.*t687.*t2659;
t3185 = t8.*t703.*t2659;
t3214 = -t3178;
t3230 = t1728+t2008;
t3232 = t3178./2.0;
t3234 = t3183./2.0;
t3250 = t8.*t1036.*t2507;
t3259 = -t14.*t1036.*(t859-t1704);
t3260 = t8.*t1055.*t2507;
t3272 = -t14.*t1055.*(t859-t1704);
t3306 = t14.*t1055.*(t859-t1704).*(-1.0./2.0);
t3318 = t799.*t2749;
t3331 = t1298.*t2507;
t3336 = -t1288.*(t859-t1704);
t3345 = t8.*t1036.*t2659;
t3348 = t8.*t1302.*t2507;
t3351 = t8.*t1055.*t2659;
t3354 = -t14.*t1302.*(t859-t1704);
t3363 = t1288.*(t859-t1704).*(-1.0./2.0);
t3384 = (t8.*t1321.*t2507)./2.0;
t3399 = t14.*t1321.*(t859-t1704).*(-1.0./2.0);
t3414 = t23.*t1807.*t2140;
t3416 = t26.*t1807.*t2140;
t3421 = (t14.*t1807.*t2123)./2.0;
t3429 = t2045+t2051;
t3431 = t2047+t2055;
t3432 = t2048+t2056;
t3439 = t3400./2.0;
t3440 = t3401./2.0;
t3445 = -t3422;
t3456 = t3415./2.0;
t3467 = t8.*t1302.*t2659;
t3469 = t3422./2.0;
t3500 = (t8.*t1321.*t2659)./2.0;
t3504 = -t3496;
t3528 = -t721.*(t873-t2434);
t3531 = t2659.*(t441-t846).*(-1.0./2.0);
t3543 = t3516./2.0;
t3544 = t3517./2.0;
t3545 = -t705.*(t910-t2473);
t3546 = t721.*(t873-t2434);
t3567 = t705.*(t910-t2473);
t3574 = -t3553;
t3578 = (t23.*t1807.*t2357)./2.0;
t3582 = (t26.*t1807.*t2357)./2.0;
t3590 = (t14.*t2113.*t2123)./2.0;
t3598 = t3553./2.0;
t3601 = t3557./2.0;
t3612 = -t18.*t39.*(-t495-t548+t650+t659+t739+t14.*t37.*(t101-t401));
t3617 = -t3593;
t3622 = t3575./2.0;
t3630 = t3593./2.0;
t3649 = t18.*t39.*(-t495-t548+t650+t659+t739+t14.*t37.*(t101-t401)).*(-1.0./2.0);
t3686 = t2217+t2231;
t3687 = t2218+t2232;
t3701 = (t14.*t2123.*t2279)./2.0;
t3712 = t1977.*t2507;
t3720 = -t1962.*(t859-t1704);
t3721 = -t255.*(-t495-t548+t650+t659+t739+t14.*t37.*(t101-t401));
t3737 = -t8.*t1082.*(t873-t2434);
t3745 = (t23.*t2140.*t2279)./2.0;
t3747 = (t26.*t2140.*t2279)./2.0;
t3752 = -t330.*(-t495-t548+t650+t659+t739+t14.*t37.*(t101-t401));
t3758 = -t341.*(-t495-t548+t650+t659+t739+t14.*t37.*(t101-t401));
t3760 = t1962.*(t859-t1704).*(-1.0./2.0);
t3761 = -t3746;
t3770 = (t23.*t2113.*t2357)./2.0;
t3771 = (t26.*t2113.*t2357)./2.0;
t3774 = t8.*t1082.*(t873-t2434).*(-1.0./2.0);
t3778 = -t14.*t1082.*(t910-t2473);
t3779 = t330.*(-t495-t548+t650+t659+t739+t14.*t37.*(t101-t401));
t3786 = -t402.*(-t495-t548+t650+t659+t739+t14.*t37.*(t101-t401));
t3792 = t341.*(-t495-t548+t650+t659+t739+t14.*t37.*(t101-t401)).*(-1.0./2.0);
t3796 = -t1297.*(t873-t2434);
t3806 = t14.*t1082.*(t910-t2473).*(-1.0./2.0);
t3813 = t402.*(-t495-t548+t650+t659+t739+t14.*t37.*(t101-t401)).*(-1.0./2.0);
t3817 = t2334+t2338;
t3821 = t2336+t2341;
t3822 = t2337+t2342;
t3827 = -t1287.*(t910-t2473);
t3830 = t1297.*(t873-t2434).*(-1.0./2.0);
t3840 = t2174.*t2507;
t3846 = t1287.*(t910-t2473);
t3849 = -t2168.*(t859-t1704);
t3875 = t2168.*(t859-t1704);
t3876 = -t609.*(-t495-t548+t650+t659+t739+t14.*t37.*(t101-t401));
t3906 = (t100-t364).*(-t495-t548+t650+t659+t739+t14.*t37.*(t101-t401));
t3907 = t609.*(-t495-t548+t650+t659+t739+t14.*t37.*(t101-t401));
t3910 = -t641.*(-t495-t548+t650+t659+t739+t14.*t37.*(t101-t401));
t3940 = (t101-t401).*(-t495-t548+t650+t659+t739+t14.*t37.*(t101-t401));
t3941 = t641.*(-t495-t548+t650+t659+t739+t14.*t37.*(t101-t401));
t4025 = t2495+t2496;
t4059 = -t8.*t1807.*(t873-t2434);
t4064 = -t8.*t1818.*(t873-t2434);
t4069 = -t14.*t1807.*(t910-t2473);
t4071 = t8.*t1818.*(t873-t2434).*(-1.0./2.0);
t4072 = -t14.*t1818.*(t910-t2473);
t4075 = t2507.*t2659;
t4076 = -t1976.*(t873-t2434);
t4084 = t14.*t1818.*(t910-t2473).*(-1.0./2.0);
t4086 = t1976.*(t873-t2434).*(-1.0./2.0);
t4089 = -t1961.*(t910-t2473);
t4098 = t1961.*(t910-t2473);
t4126 = -t8.*t2113.*(t873-t2434);
t4129 = -t2173.*(t873-t2434);
t4133 = -t8.*t2140.*(t873-t2434);
t4134 = -t14.*t2113.*(t910-t2473);
t4135 = t8.*t687.*t3905;
t4139 = -t14.*t687.*(t855-t885-t1427+t1706);
t4140 = t2123.*(t910-t2473).*(-1.0./2.0);
t4141 = -t2167.*(t910-t2473);
t4144 = t2173.*(t873-t2434).*(-1.0./2.0);
t4146 = t8.*t2140.*(t873-t2434).*(-1.0./2.0);
t4147 = -t14.*t2140.*(t910-t2473);
t4150 = t2167.*(t910-t2473);
t4152 = t14.*t687.*(t855-t885-t1427+t1706).*(-1.0./2.0);
t4157 = t14.*t2140.*(t910-t2473).*(-1.0./2.0);
t4159 = -t8.*t2279.*(t873-t2434);
t4172 = -t14.*t2279.*(t910-t2473);
t4199 = t8.*t2357.*(t873-t2434).*(-1.0./2.0);
t4203 = (t8.*t2357.*(t873-t2434))./2.0;
t4207 = t8.*t1036.*t3905;
t4212 = -t14.*t1036.*(t855-t885-t1427+t1706);
t4216 = t14.*t2357.*(t910-t2473).*(-1.0./2.0);
t4230 = (t14.*t2357.*(t910-t2473))./2.0;
t4236 = t14.*t1036.*(t855-t885-t1427+t1706).*(-1.0./2.0);
t4299 = t8.*t1302.*t3905;
t4304 = -t14.*t1302.*(t855-t885-t1427+t1706);
t4325 = t14.*t1302.*(t855-t885-t1427+t1706).*(-1.0./2.0);
t4332 = (t14.*t1302.*(t855-t885-t1427+t1706))./2.0;
t4466 = t1431+t1730+t2019+t2038;
t4538 = t2507.*t3905;
t4551 = (t859-t1704).*(t855-t885-t1427+t1706);
t4579 = t2659.*t3905;
t4581 = -t8.*t1807.*(t870-t909-t1470+t2472);
t4598 = t8.*t1807.*(t870-t909-t1470+t2472).*(-1.0./2.0);
t4667 = -t8.*t2113.*(t870-t909-t1470+t2472);
t4671 = t8.*t2113.*(t870-t909-t1470+t2472).*(-1.0./2.0);
t4706 = -t8.*t2279.*(t870-t909-t1470+t2472);
t4719 = t8.*t2279.*(t870-t909-t1470+t2472).*(-1.0./2.0);
t531 = -t500;
t590 = -t567;
t600 = -t581;
t604 = t587.*2.0;
t605 = t588.*2.0;
t631 = -t607;
t646 = t598./2.0;
t662 = t601./2.0;
t663 = t608./2.0;
t665 = -t632;
t680 = t632./2.0;
t714 = -t702;
t808 = -t755;
t817 = -t765;
t848 = t767./2.0;
t851 = t770./2.0;
t882 = t8.*t792;
t888 = t8.*t796;
t889 = t14.*t794;
t895 = -t839;
t982 = t974.*t1dd;
t983 = t975.*t1dd;
t993 = t919./2.0;
t994 = t922./2.0;
t997 = t14.*t39.*t796;
t1004 = t402.*t566;
t1005 = t987.*2.0;
t1006 = t988.*2.0;
t1009 = t12.*t974;
t1010 = t12.*t975;
t1011 = t18.*t974;
t1012 = t18.*t975;
t1013 = t12.*t978;
t1014 = t12.*t979;
t1019 = t18.*t978;
t1020 = t18.*t979;
t1023 = -t978;
t1024 = -t979;
t1025 = t8.*t39.*t794;
t1026 = t14.*t39.*t792;
t1033 = t991.*t2d;
t1035 = -t986;
t1038 = t403.*t593;
t1049 = (t974.*t1d)./2.0;
t1050 = (t975.*t1d)./2.0;
t1053 = (t978.*t1d)./2.0;
t1054 = (t979.*t1d)./2.0;
t1056 = t34.*t979;
t1057 = t35.*t978;
t1058 = t36.*t979;
t1061 = t38.*t978;
t1073 = t39.*t974;
t1074 = t39.*t975;
t1079 = t1000./2.0;
t1080 = t1001./2.0;
t1106 = -t1045;
t1108 = -t1046;
t1111 = t18.*t39.*t898;
t1119 = t18.*t39.*t908;
t1125 = -t1062;
t1126 = t476+t563;
t1130 = t1071.*t2d;
t1131 = t1071.*t3d;
t1138 = -t1068;
t1152 = t1045./2.0;
t1157 = -t1077;
t1158 = t1046./2.0;
t1159 = t1047./2.0;
t1161 = t1048./2.0;
t1171 = t1059./2.0;
t1173 = t1062./2.0;
t1178 = t341.*t694;
t1192 = t522+t564;
t1199 = -t1155;
t1201 = t104.*t978;
t1202 = t104.*t979;
t1204 = t107.*t978;
t1205 = t107.*t979;
t1208 = t1112./2.0;
t1209 = t1113./2.0;
t1210 = t1115./2.0;
t1211 = t1116./2.0;
t1216 = t540+t565;
t1218 = t8.*t1129;
t1220 = t14.*t1128;
t1221 = t1144./2.0;
t1231 = t1190.*t2dd;
t1232 = t1190.*t3dd;
t1233 = t1190.*t4dd;
t1250 = t1183./2.0;
t1251 = t1184./2.0;
t1252 = t1185./2.0;
t1255 = t1189./2.0;
t1261 = t255.*t796;
t1269 = t542+t630;
t1270 = t587+t594;
t1274 = t558+t613;
t1280 = -t1244;
t1300 = t330.*t794;
t1309 = -t1d.*(t545-t587);
t1314 = -t1264;
t1318 = -t1268;
t1327 = t626.*(t100-t364);
t1328 = t609.*t625;
t1329 = -t1284;
t1336 = t1264./2.0;
t1337 = t255.*t898;
t1338 = t1267./2.0;
t1339 = t255.*t908;
t1344 = -t1319;
t1345 = -t1320;
t1354 = t1284./2.0;
t1357 = t1d.*(t545-t587);
t1362 = -t1315;
t1374 = t18.*t39.*t1187;
t1383 = t1307./2.0;
t1387 = t330.*t898;
t1389 = t330.*t908;
t1390 = t1322./2.0;
t1391 = t1323./2.0;
t1392 = t1324./2.0;
t1393 = t1325./2.0;
t1394 = t1376.*(-1.0./2.0);
Y = ft_4({t100,t1000,t1001,t1002,t1003,t1004,t1005,t1006,t1007,t1008,t1009,t101,t1010,t1011,t1012,t1013,t1014,t1015,t1016,t1017,t1018,t1019,t1020,t1021,t1022,t1023,t1024,t1025,t1026,t1028,t1029,t1030,t1033,t1034,t1035,t1036,t1038,t104,t1041,t1045,t1046,t1047,t1048,t1049,t1050,t1051,t1052,t1053,t1054,t1055,t1056,t1058,t1059,t106,t1062,t1065,t1066,t1068,t1069,t107,t1070,t1071,t1073,t1074,t1075,t1079,t108,t1080,t1082,t1085,t1086,t1087,t1089,t1092,t1093,t1094,t1096,t1097,t1098,t1099,t1106,t1107,t1108,t111,t1111,t1112,t1113,t1115,t1116,t1117,t1119,t112,t1121,t1122,t1123,t1125,t1126,t1128,t1129,t113,t1130,t1131,t1133,t1134,t1135,t1137,t1138,t1139,t1140,t1141,t115,t1151,t1152,t1153,t1155,t1156,t1157,t1158,t1159,t1161,t1164,t1166,t1167,t1168,t1171,t1172,t1173,t1174,t1176,t1177,t1178,t1179,t1180,t1183,t1184,t1185,t1186,t1187,t1188,t1189,t1192,t1193,t1195,t1196,t1198,t1199,t12,t1201,t1202,t1203,t1204,t1205,t1208,t1209,t1210,t1211,t1213,t1216,t1218,t1219,t1220,t1221,t1222,t1223,t1224,t1225,t1226,t1227,t1229,t1230,t1231,t1232,t1233,t1235,t1236,t1237,t1238,t124,t1242,t1245,t1246,t1248,t1250,t1251,t1252,t1253,t1254,t1255,t1261,t1262,t1263,t1264,t1265,t1267,t1268,t1269,t127,t1270,t1274,t1277,t1278,t128,t1280,t1283,t1284,t1285,t1287,t1288,t1291,t1292,t1293,t1294,t1295,t1296,t1297,t1298,t13,t1300,t1302,t1305,t1306,t1307,t131,t1310,t1311,t1313,t1314,t1315,t1316,t1318,t132,t1321,t1323,t1324,t1325,t1328,t1329,t1330,t1331,t1332,t1333,t1334,t1335,t1336,t1337,t1338,t1339,t134,t1340,t1341,t1342,t1343,t1344,t1345,t1351,t1352,t1353,t1354,t1355,t1357,t1358,t136,t1360,t1362,t1366,t1368,t1369,t137,t1370,t1371,t1374,t1375,t1376,t1378,t138,t1382,t1383,t1387,t1389,t1390,t1391,t1392,t1393,t1398,t1399,t14,t1400,t1401,t1403,t1406,t1410,t1413,t1414,t1415,t1416,t1417,t1418,t1419,t1420,t1424,t1425,t1426,t1427,t1434,t1435,t1439,t1440,t1441,t1442,t1443,t1444,t1445,t1452,t1454,t1458,t1462,t1463,t1468,t1470,t1471,t1485,t1490,t1491,t1492,t1493,t1494,t1495,t1497,t1499,t15,t150,t1500,t1501,t1502,t1504,t1505,t1506,t1516,t1517,t1518,t1519,t152,t1520,t1521,t1522,t1523,t1527,t1530,t1531,t1532,t1534,t1535,t1536,t1537,t1545,t1547,t155,t1551,t1552,t1553,t156,t1574,t158,t1583,t1584,t1585,t159,t1591,t1593,t160,t1618,t162,t1627,t1628,t1629,t163,t1630,t1631,t1636,t1637,t164,t165,t1650,t1651,t1652,t1653,t1659,t1666,t1667,t1669,t1674,t1677,t1678,t1679,t1680,t1699,t1701,t1703,t1704,t1705,t1706,t1709,t171,t1710,t1713,t1714,t1723,t173,t1733,t1734,t1736,t174,t1740,t1741,t175,t1750,t1751,t1753,t1754,t1755,t1757,t1758,t1759,t1768,t1769,t177,t1770,t1771,t1772,t1773,t1775,t1780,t18,t1801,t1807,t1817,t1818,t1831,t1834,t1837,t1839,t1840,t1845,t1846,t1847,t1848,t1863,t1866,t1868,t187,t1874,t1875,t1886,t1888,t1889,t1890,t1891,t19,t1905,t1907,t191,t1910,t1916,t1925,t1930,t1937,t1944,t196,t1961,t1962,t1963,t1965,t1968,t1969,t1971,t1973,t1976,t1977,t1984,t1988,t199,t1995,t1999,t1d,t1dd,t200,t201,t2011,t2017,t202,t2025,t2037,t2039,t2044,t2046,t2049,t2052,t206,t2063,t2070,t2074,t2075,t2081,t2085,t2086,t2087,t2090,t2093,t21,t210,t2100,t2101,t2109,t2110,t2112,t2113,t2116,t2117,t2118,t2119,t2120,t2122,t2123,t2124,t2127,t2128,t2131,t2132,t2133,t2135,t2136,t2140,t2141,t2142,t2144,t2145,t2147,t2149,t215,t2150,t2155,t2156,t2159,t2160,t2162,t2167,t2168,t2169,t2170,t2173,t2174,t2178,t2179,t2183,t2184,t2189,t219,t2190,t2194,t2196,t22,t220,t2206,t2207,t221,t2210,t2227,t2233,t2234,t226,t2267,t2270,t2279,t228,t2281,t2286,t229,t2298,t23,t2300,t2302,t231,t2311,t2315,t2318,t232,t233,t2340,t2344,t2345,t2346,t2347,t2348,t2353,t2354,t2357,t2359,t2371,t2372,t2374,t2383,t2388,t2393,t2395,t2397,t2398,t2399,t24,t2400,t2401,t2425,t243,t2434,t2438,t244,t245,t2453,t2454,t2458,t2467,t2469,t247,t2472,t2473,t2474,t2478,t248,t2484,t2485,t249,t2490,t25,t2505,t2507,t2508,t2509,t2511,t2519,t2527,t2529,t2530,t2539,t255,t2557,t256,t2560,t2565,t2572,t2576,t258,t2593,t26,t2606,t2619,t263,t2630,t2642,t2644,t2648,t2655,t2658,t2659,t2662,t2663,t2666,t2671,t2672,t268,t2687,t27,t2706,t2708,t2714,t2718,t2719,t2743,t2744,t2745,t2747,t2749,t2755,t276,t2772,t2775,t2776,t2777,t2779,t2780,t279,t2790,t2796,t2798,t2799,t28,t2813,t283,t2839,t2849,t2862,t2871,t2876,t2897,t29,t2915,t2919,t2927,t2929,t2937,t2938,t2953,t2956,t2983,t2985,t2989,t299,t2995,t2996,t2999,t2d,t2dd,t30,t3007,t301,t3012,t3013,t3014,t3018,t3028,t303,t3032,t3034,t3035,t304,t3043,t3045,t3059,t3060,t3069,t3072,t3073,t3078,t308,t3080,t3083,t3086,t3088,t309,t31,t310,t3122,t3129,t3130,t3148,t315,t3160,t317,t318,t3183,t3185,t319,t320,t321,t3214,t3230,t3232,t3234,t325,t3250,t3259,t3260,t3272,t3288,t3289,t329,t3291,t3292,t330,t3306,t3308,t331,t3318,t332,t3321,t333,t3330,t3331,t3332,t334,t3345,t3348,t3351,t3354,t3384,t3388,t339,t3391,t3399,t34,t3400,t3401,t3404,t3405,t341,t3414,t3415,t3416,t342,t3421,t3429,t343,t3431,t3432,t3439,t344,t3440,t3445,t345,t3456,t346,t3467,t3469,t347,t3488,t35,t3500,t3504,t3509,t3510,t3516,t3517,t3531,t354,t3543,t3544,t3546,t3557,t3567,t3574,t3575,t3578,t3582,t3590,t3598,t36,t360,t3601,t361,t3612,t3617,t3622,t363,t3630,t364,t3649,t365,t368,t3683,t3685,t3686,t3687,t37,t3701,t3712,t3721,t3743,t3745,t3747,t375,t3758,t3761,t3770,t3771,t3779,t3786,t3792,t3796,t38,t3813,t3817,t3821,t3822,t383,t3830,t384,t3840,t3846,t3875,t39,t3906,t3907,t392,t393,t394,t3940,t3941,t395,t3d,t3dd,t400,t401,t402,t4025,t403,t404,t4059,t4069,t4071,t4075,t4076,t4084,t4086,t4098,t41,t410,t411,t412,t4126,t4129,t413,t4133,t4134,t4135,t4139,t414,t4140,t4144,t4146,t4147,t415,t4150,t4152,t4157,t4159,t416,t417,t4172,t418,t419,t42,t420,t4203,t4207,t4212,t4230,t4236,t425,t428,t4299,t43,t4304,t431,t4325,t4332,t434,t437,t441,t442,t443,t444,t445,t446,t4466,t453,t4538,t454,t455,t4551,t4579,t459,t467,t468,t470,t472,t477,t478,t48,t483,t484,t486,t487,t488,t489,t492,t493,t494,t495,t496,t497,t498,t499,t4d,t4dd,t50,t501,t502,t503,t507,t508,t51,t513,t514,t515,t516,t519,t523,t524,t529,t53,t530,t531,t532,t535,t537,t542,t543,t544,t546,t547,t548,t549,t55,t550,t552,t553,t554,t56,t562,t566,t569,t57,t570,t571,t579,t58,t580,t582,t585,t587,t588,t589,t590,t591,t593,t595,t596,t598,t5d,t5dd,t600,t601,t602,t604,t605,t608,t609,t61,t612,t614,t615,t616,t617,t623,t624,t625,t626,t627,t63,t631,t632,t633,t634,t635,t636,t637,t639,t641,t642,t643,t644,t645,t646,t647,t648,t649,t650,t651,t652,t653,t654,t655,t656,t657,t658,t659,t660,t661,t662,t663,t664,t665,t667,t668,t669,t670,t671,t673,t674,t675,t676,t680,t681,t682,t683,t684,t685,t686,t687,t689,t69,t690,t694,t695,t696,t697,t698,t699,t6d,t6dd,t700,t701,t702,t703,t705,t706,t71,t711,t712,t713,t714,t720,t721,t723,t724,t725,t726,t727,t728,t729,t731,t732,t733,t735,t736,t737,t738,t739,t740,t742,t745,t746,t747,t748,t749,t75,t750,t752,t753,t754,t755,t756,t757,t759,t760,t761,t762,t763,t764,t766,t767,t768,t769,t770,t772,t774,t775,t776,t780,t781,t782,t783,t785,t786,t788,t789,t793,t799,t8,t802,t803,t804,t805,t806,t807,t808,t810,t814,t815,t817,t82,t820,t823,t824,t825,t826,t827,t828,t829,t830,t831,t832,t833,t835,t836,t838,t840,t842,t843,t844,t846,t848,t849,t850,t851,t852,t853,t854,t855,t859,t861,t865,t866,t867,t868,t869,t870,t871,t873,t874,t877,t879,t88,t880,t882,t883,t884,t885,t887,t888,t889,t890,t891,t892,t894,t895,t896,t897,t898,t899,t9,t900,t901,t902,t904,t907,t908,t909,t910,t911,t912,t913,t915,t917,t919,t921,t922,t923,t927,t928,t931,t932,t937,t938,t943,t944,t945,t952,t954,t955,t956,t957,t959,t960,t961,t962,t963,t964,t965,t966,t968,t969,t970,t971,t972,t973,t974,t975,t978,t979,t980,t981,t982,t983,t984,t985,t986,t987,t989,t992,t993,t994,t997,t998,t999});
end
function Y = ft_4(ct)
t100 = ct{1};
t1000 = ct{2};
t1001 = ct{3};
t1002 = ct{4};
t1003 = ct{5};
t1004 = ct{6};
t1005 = ct{7};
t1006 = ct{8};
t1007 = ct{9};
t1008 = ct{10};
t1009 = ct{11};
t101 = ct{12};
t1010 = ct{13};
t1011 = ct{14};
t1012 = ct{15};
t1013 = ct{16};
t1014 = ct{17};
t1015 = ct{18};
t1016 = ct{19};
t1017 = ct{20};
t1018 = ct{21};
t1019 = ct{22};
t1020 = ct{23};
t1021 = ct{24};
t1022 = ct{25};
t1023 = ct{26};
t1024 = ct{27};
t1025 = ct{28};
t1026 = ct{29};
t1028 = ct{30};
t1029 = ct{31};
t1030 = ct{32};
t1033 = ct{33};
t1034 = ct{34};
t1035 = ct{35};
t1036 = ct{36};
t1038 = ct{37};
t104 = ct{38};
t1041 = ct{39};
t1045 = ct{40};
t1046 = ct{41};
t1047 = ct{42};
t1048 = ct{43};
t1049 = ct{44};
t1050 = ct{45};
t1051 = ct{46};
t1052 = ct{47};
t1053 = ct{48};
t1054 = ct{49};
t1055 = ct{50};
t1056 = ct{51};
t1058 = ct{52};
t1059 = ct{53};
t106 = ct{54};
t1062 = ct{55};
t1065 = ct{56};
t1066 = ct{57};
t1068 = ct{58};
t1069 = ct{59};
t107 = ct{60};
t1070 = ct{61};
t1071 = ct{62};
t1073 = ct{63};
t1074 = ct{64};
t1075 = ct{65};
t1079 = ct{66};
t108 = ct{67};
t1080 = ct{68};
t1082 = ct{69};
t1085 = ct{70};
t1086 = ct{71};
t1087 = ct{72};
t1089 = ct{73};
t1092 = ct{74};
t1093 = ct{75};
t1094 = ct{76};
t1096 = ct{77};
t1097 = ct{78};
t1098 = ct{79};
t1099 = ct{80};
t1106 = ct{81};
t1107 = ct{82};
t1108 = ct{83};
t111 = ct{84};
t1111 = ct{85};
t1112 = ct{86};
t1113 = ct{87};
t1115 = ct{88};
t1116 = ct{89};
t1117 = ct{90};
t1119 = ct{91};
t112 = ct{92};
t1121 = ct{93};
t1122 = ct{94};
t1123 = ct{95};
t1125 = ct{96};
t1126 = ct{97};
t1128 = ct{98};
t1129 = ct{99};
t113 = ct{100};
t1130 = ct{101};
t1131 = ct{102};
t1133 = ct{103};
t1134 = ct{104};
t1135 = ct{105};
t1137 = ct{106};
t1138 = ct{107};
t1139 = ct{108};
t1140 = ct{109};
t1141 = ct{110};
t115 = ct{111};
t1151 = ct{112};
t1152 = ct{113};
t1153 = ct{114};
t1155 = ct{115};
t1156 = ct{116};
t1157 = ct{117};
t1158 = ct{118};
t1159 = ct{119};
t1161 = ct{120};
t1164 = ct{121};
t1166 = ct{122};
t1167 = ct{123};
t1168 = ct{124};
t1171 = ct{125};
t1172 = ct{126};
t1173 = ct{127};
t1174 = ct{128};
t1176 = ct{129};
t1177 = ct{130};
t1178 = ct{131};
t1179 = ct{132};
t1180 = ct{133};
t1183 = ct{134};
t1184 = ct{135};
t1185 = ct{136};
t1186 = ct{137};
t1187 = ct{138};
t1188 = ct{139};
t1189 = ct{140};
t1192 = ct{141};
t1193 = ct{142};
t1195 = ct{143};
t1196 = ct{144};
t1198 = ct{145};
t1199 = ct{146};
t12 = ct{147};
t1201 = ct{148};
t1202 = ct{149};
t1203 = ct{150};
t1204 = ct{151};
t1205 = ct{152};
t1208 = ct{153};
t1209 = ct{154};
t1210 = ct{155};
t1211 = ct{156};
t1213 = ct{157};
t1216 = ct{158};
t1218 = ct{159};
t1219 = ct{160};
t1220 = ct{161};
t1221 = ct{162};
t1222 = ct{163};
t1223 = ct{164};
t1224 = ct{165};
t1225 = ct{166};
t1226 = ct{167};
t1227 = ct{168};
t1229 = ct{169};
t1230 = ct{170};
t1231 = ct{171};
t1232 = ct{172};
t1233 = ct{173};
t1235 = ct{174};
t1236 = ct{175};
t1237 = ct{176};
t1238 = ct{177};
t124 = ct{178};
t1242 = ct{179};
t1245 = ct{180};
t1246 = ct{181};
t1248 = ct{182};
t1250 = ct{183};
t1251 = ct{184};
t1252 = ct{185};
t1253 = ct{186};
t1254 = ct{187};
t1255 = ct{188};
t1261 = ct{189};
t1262 = ct{190};
t1263 = ct{191};
t1264 = ct{192};
t1265 = ct{193};
t1267 = ct{194};
t1268 = ct{195};
t1269 = ct{196};
t127 = ct{197};
t1270 = ct{198};
t1274 = ct{199};
t1277 = ct{200};
t1278 = ct{201};
t128 = ct{202};
t1280 = ct{203};
t1283 = ct{204};
t1284 = ct{205};
t1285 = ct{206};
t1287 = ct{207};
t1288 = ct{208};
t1291 = ct{209};
t1292 = ct{210};
t1293 = ct{211};
t1294 = ct{212};
t1295 = ct{213};
t1296 = ct{214};
t1297 = ct{215};
t1298 = ct{216};
t13 = ct{217};
t1300 = ct{218};
t1302 = ct{219};
t1305 = ct{220};
t1306 = ct{221};
t1307 = ct{222};
t131 = ct{223};
t1310 = ct{224};
t1311 = ct{225};
t1313 = ct{226};
t1314 = ct{227};
t1315 = ct{228};
t1316 = ct{229};
t1318 = ct{230};
t132 = ct{231};
t1321 = ct{232};
t1323 = ct{233};
t1324 = ct{234};
t1325 = ct{235};
t1328 = ct{236};
t1329 = ct{237};
t1330 = ct{238};
t1331 = ct{239};
t1332 = ct{240};
t1333 = ct{241};
t1334 = ct{242};
t1335 = ct{243};
t1336 = ct{244};
t1337 = ct{245};
t1338 = ct{246};
t1339 = ct{247};
t134 = ct{248};
t1340 = ct{249};
t1341 = ct{250};
t1342 = ct{251};
t1343 = ct{252};
t1344 = ct{253};
t1345 = ct{254};
t1351 = ct{255};
t1352 = ct{256};
t1353 = ct{257};
t1354 = ct{258};
t1355 = ct{259};
t1357 = ct{260};
t1358 = ct{261};
t136 = ct{262};
t1360 = ct{263};
t1362 = ct{264};
t1366 = ct{265};
t1368 = ct{266};
t1369 = ct{267};
t137 = ct{268};
t1370 = ct{269};
t1371 = ct{270};
t1374 = ct{271};
t1375 = ct{272};
t1376 = ct{273};
t1378 = ct{274};
t138 = ct{275};
t1382 = ct{276};
t1383 = ct{277};
t1387 = ct{278};
t1389 = ct{279};
t1390 = ct{280};
t1391 = ct{281};
t1392 = ct{282};
t1393 = ct{283};
t1398 = ct{284};
t1399 = ct{285};
t14 = ct{286};
t1400 = ct{287};
t1401 = ct{288};
t1403 = ct{289};
t1406 = ct{290};
t1410 = ct{291};
t1413 = ct{292};
t1414 = ct{293};
t1415 = ct{294};
t1416 = ct{295};
t1417 = ct{296};
t1418 = ct{297};
t1419 = ct{298};
t1420 = ct{299};
t1424 = ct{300};
t1425 = ct{301};
t1426 = ct{302};
t1427 = ct{303};
t1434 = ct{304};
t1435 = ct{305};
t1439 = ct{306};
t1440 = ct{307};
t1441 = ct{308};
t1442 = ct{309};
t1443 = ct{310};
t1444 = ct{311};
t1445 = ct{312};
t1452 = ct{313};
t1454 = ct{314};
t1458 = ct{315};
t1462 = ct{316};
t1463 = ct{317};
t1468 = ct{318};
t1470 = ct{319};
t1471 = ct{320};
t1485 = ct{321};
t1490 = ct{322};
t1491 = ct{323};
t1492 = ct{324};
t1493 = ct{325};
t1494 = ct{326};
t1495 = ct{327};
t1497 = ct{328};
t1499 = ct{329};
t15 = ct{330};
t150 = ct{331};
t1500 = ct{332};
t1501 = ct{333};
t1502 = ct{334};
t1504 = ct{335};
t1505 = ct{336};
t1506 = ct{337};
t1516 = ct{338};
t1517 = ct{339};
t1518 = ct{340};
t1519 = ct{341};
t152 = ct{342};
t1520 = ct{343};
t1521 = ct{344};
t1522 = ct{345};
t1523 = ct{346};
t1527 = ct{347};
t1530 = ct{348};
t1531 = ct{349};
t1532 = ct{350};
t1534 = ct{351};
t1535 = ct{352};
t1536 = ct{353};
t1537 = ct{354};
t1545 = ct{355};
t1547 = ct{356};
t155 = ct{357};
t1551 = ct{358};
t1552 = ct{359};
t1553 = ct{360};
t156 = ct{361};
t1574 = ct{362};
t158 = ct{363};
t1583 = ct{364};
t1584 = ct{365};
t1585 = ct{366};
t159 = ct{367};
t1591 = ct{368};
t1593 = ct{369};
t160 = ct{370};
t1618 = ct{371};
t162 = ct{372};
t1627 = ct{373};
t1628 = ct{374};
t1629 = ct{375};
t163 = ct{376};
t1630 = ct{377};
t1631 = ct{378};
t1636 = ct{379};
t1637 = ct{380};
t164 = ct{381};
t165 = ct{382};
t1650 = ct{383};
t1651 = ct{384};
t1652 = ct{385};
t1653 = ct{386};
t1659 = ct{387};
t1666 = ct{388};
t1667 = ct{389};
t1669 = ct{390};
t1674 = ct{391};
t1677 = ct{392};
t1678 = ct{393};
t1679 = ct{394};
t1680 = ct{395};
t1699 = ct{396};
t1701 = ct{397};
t1703 = ct{398};
t1704 = ct{399};
t1705 = ct{400};
t1706 = ct{401};
t1709 = ct{402};
t171 = ct{403};
t1710 = ct{404};
t1713 = ct{405};
t1714 = ct{406};
t1723 = ct{407};
t173 = ct{408};
t1733 = ct{409};
t1734 = ct{410};
t1736 = ct{411};
t174 = ct{412};
t1740 = ct{413};
t1741 = ct{414};
t175 = ct{415};
t1750 = ct{416};
t1751 = ct{417};
t1753 = ct{418};
t1754 = ct{419};
t1755 = ct{420};
t1757 = ct{421};
t1758 = ct{422};
t1759 = ct{423};
t1768 = ct{424};
t1769 = ct{425};
t177 = ct{426};
t1770 = ct{427};
t1771 = ct{428};
t1772 = ct{429};
t1773 = ct{430};
t1775 = ct{431};
t1780 = ct{432};
t18 = ct{433};
t1801 = ct{434};
t1807 = ct{435};
t1817 = ct{436};
t1818 = ct{437};
t1831 = ct{438};
t1834 = ct{439};
t1837 = ct{440};
t1839 = ct{441};
t1840 = ct{442};
t1845 = ct{443};
t1846 = ct{444};
t1847 = ct{445};
t1848 = ct{446};
t1863 = ct{447};
t1866 = ct{448};
t1868 = ct{449};
t187 = ct{450};
t1874 = ct{451};
t1875 = ct{452};
t1886 = ct{453};
t1888 = ct{454};
t1889 = ct{455};
t1890 = ct{456};
t1891 = ct{457};
t19 = ct{458};
t1905 = ct{459};
t1907 = ct{460};
t191 = ct{461};
t1910 = ct{462};
t1916 = ct{463};
t1925 = ct{464};
t1930 = ct{465};
t1937 = ct{466};
t1944 = ct{467};
t196 = ct{468};
t1961 = ct{469};
t1962 = ct{470};
t1963 = ct{471};
t1965 = ct{472};
t1968 = ct{473};
t1969 = ct{474};
t1971 = ct{475};
t1973 = ct{476};
t1976 = ct{477};
t1977 = ct{478};
t1984 = ct{479};
t1988 = ct{480};
t199 = ct{481};
t1995 = ct{482};
t1999 = ct{483};
t1d = ct{484};
t1dd = ct{485};
t200 = ct{486};
t201 = ct{487};
t2011 = ct{488};
t2017 = ct{489};
t202 = ct{490};
t2025 = ct{491};
t2037 = ct{492};
t2039 = ct{493};
t2044 = ct{494};
t2046 = ct{495};
t2049 = ct{496};
t2052 = ct{497};
t206 = ct{498};
t2063 = ct{499};
t2070 = ct{500};
t2074 = ct{501};
t2075 = ct{502};
t2081 = ct{503};
t2085 = ct{504};
t2086 = ct{505};
t2087 = ct{506};
t2090 = ct{507};
t2093 = ct{508};
t21 = ct{509};
t210 = ct{510};
t2100 = ct{511};
t2101 = ct{512};
t2109 = ct{513};
t2110 = ct{514};
t2112 = ct{515};
t2113 = ct{516};
t2116 = ct{517};
t2117 = ct{518};
t2118 = ct{519};
t2119 = ct{520};
t2120 = ct{521};
t2122 = ct{522};
t2123 = ct{523};
t2124 = ct{524};
t2127 = ct{525};
t2128 = ct{526};
t2131 = ct{527};
t2132 = ct{528};
t2133 = ct{529};
t2135 = ct{530};
t2136 = ct{531};
t2140 = ct{532};
t2141 = ct{533};
t2142 = ct{534};
t2144 = ct{535};
t2145 = ct{536};
t2147 = ct{537};
t2149 = ct{538};
t215 = ct{539};
t2150 = ct{540};
t2155 = ct{541};
t2156 = ct{542};
t2159 = ct{543};
t2160 = ct{544};
t2162 = ct{545};
t2167 = ct{546};
t2168 = ct{547};
t2169 = ct{548};
t2170 = ct{549};
t2173 = ct{550};
t2174 = ct{551};
t2178 = ct{552};
t2179 = ct{553};
t2183 = ct{554};
t2184 = ct{555};
t2189 = ct{556};
t219 = ct{557};
t2190 = ct{558};
t2194 = ct{559};
t2196 = ct{560};
t22 = ct{561};
t220 = ct{562};
t2206 = ct{563};
t2207 = ct{564};
t221 = ct{565};
t2210 = ct{566};
t2227 = ct{567};
t2233 = ct{568};
t2234 = ct{569};
t226 = ct{570};
t2267 = ct{571};
t2270 = ct{572};
t2279 = ct{573};
t228 = ct{574};
t2281 = ct{575};
t2286 = ct{576};
t229 = ct{577};
t2298 = ct{578};
t23 = ct{579};
t2300 = ct{580};
t2302 = ct{581};
t231 = ct{582};
t2311 = ct{583};
t2315 = ct{584};
t2318 = ct{585};
t232 = ct{586};
t233 = ct{587};
t2340 = ct{588};
t2344 = ct{589};
t2345 = ct{590};
t2346 = ct{591};
t2347 = ct{592};
t2348 = ct{593};
t2353 = ct{594};
t2354 = ct{595};
t2357 = ct{596};
t2359 = ct{597};
t2371 = ct{598};
t2372 = ct{599};
t2374 = ct{600};
t2383 = ct{601};
t2388 = ct{602};
t2393 = ct{603};
t2395 = ct{604};
t2397 = ct{605};
t2398 = ct{606};
t2399 = ct{607};
t24 = ct{608};
t2400 = ct{609};
t2401 = ct{610};
t2425 = ct{611};
t243 = ct{612};
t2434 = ct{613};
t2438 = ct{614};
t244 = ct{615};
t245 = ct{616};
t2453 = ct{617};
t2454 = ct{618};
t2458 = ct{619};
t2467 = ct{620};
t2469 = ct{621};
t247 = ct{622};
t2472 = ct{623};
t2473 = ct{624};
t2474 = ct{625};
t2478 = ct{626};
t248 = ct{627};
t2484 = ct{628};
t2485 = ct{629};
t249 = ct{630};
t2490 = ct{631};
t25 = ct{632};
t2505 = ct{633};
t2507 = ct{634};
t2508 = ct{635};
t2509 = ct{636};
t2511 = ct{637};
t2519 = ct{638};
t2527 = ct{639};
t2529 = ct{640};
t2530 = ct{641};
t2539 = ct{642};
t255 = ct{643};
t2557 = ct{644};
t256 = ct{645};
t2560 = ct{646};
t2565 = ct{647};
t2572 = ct{648};
t2576 = ct{649};
t258 = ct{650};
t2593 = ct{651};
t26 = ct{652};
t2606 = ct{653};
t2619 = ct{654};
t263 = ct{655};
t2630 = ct{656};
t2642 = ct{657};
t2644 = ct{658};
t2648 = ct{659};
t2655 = ct{660};
t2658 = ct{661};
t2659 = ct{662};
t2662 = ct{663};
t2663 = ct{664};
t2666 = ct{665};
t2671 = ct{666};
t2672 = ct{667};
t268 = ct{668};
t2687 = ct{669};
t27 = ct{670};
t2706 = ct{671};
t2708 = ct{672};
t2714 = ct{673};
t2718 = ct{674};
t2719 = ct{675};
t2743 = ct{676};
t2744 = ct{677};
t2745 = ct{678};
t2747 = ct{679};
t2749 = ct{680};
t2755 = ct{681};
t276 = ct{682};
t2772 = ct{683};
t2775 = ct{684};
t2776 = ct{685};
t2777 = ct{686};
t2779 = ct{687};
t2780 = ct{688};
t279 = ct{689};
t2790 = ct{690};
t2796 = ct{691};
t2798 = ct{692};
t2799 = ct{693};
t28 = ct{694};
t2813 = ct{695};
t283 = ct{696};
t2839 = ct{697};
t2849 = ct{698};
t2862 = ct{699};
t2871 = ct{700};
t2876 = ct{701};
t2897 = ct{702};
t29 = ct{703};
t2915 = ct{704};
t2919 = ct{705};
t2927 = ct{706};
t2929 = ct{707};
t2937 = ct{708};
t2938 = ct{709};
t2953 = ct{710};
t2956 = ct{711};
t2983 = ct{712};
t2985 = ct{713};
t2989 = ct{714};
t299 = ct{715};
t2995 = ct{716};
t2996 = ct{717};
t2999 = ct{718};
t2d = ct{719};
t2dd = ct{720};
t30 = ct{721};
t3007 = ct{722};
t301 = ct{723};
t3012 = ct{724};
t3013 = ct{725};
t3014 = ct{726};
t3018 = ct{727};
t3028 = ct{728};
t303 = ct{729};
t3032 = ct{730};
t3034 = ct{731};
t3035 = ct{732};
t304 = ct{733};
t3043 = ct{734};
t3045 = ct{735};
t3059 = ct{736};
t3060 = ct{737};
t3069 = ct{738};
t3072 = ct{739};
t3073 = ct{740};
t3078 = ct{741};
t308 = ct{742};
t3080 = ct{743};
t3083 = ct{744};
t3086 = ct{745};
t3088 = ct{746};
t309 = ct{747};
t31 = ct{748};
t310 = ct{749};
t3122 = ct{750};
t3129 = ct{751};
t3130 = ct{752};
t3148 = ct{753};
t315 = ct{754};
t3160 = ct{755};
t317 = ct{756};
t318 = ct{757};
t3183 = ct{758};
t3185 = ct{759};
t319 = ct{760};
t320 = ct{761};
t321 = ct{762};
t3214 = ct{763};
t3230 = ct{764};
t3232 = ct{765};
t3234 = ct{766};
t325 = ct{767};
t3250 = ct{768};
t3259 = ct{769};
t3260 = ct{770};
t3272 = ct{771};
t3288 = ct{772};
t3289 = ct{773};
t329 = ct{774};
t3291 = ct{775};
t3292 = ct{776};
t330 = ct{777};
t3306 = ct{778};
t3308 = ct{779};
t331 = ct{780};
t3318 = ct{781};
t332 = ct{782};
t3321 = ct{783};
t333 = ct{784};
t3330 = ct{785};
t3331 = ct{786};
t3332 = ct{787};
t334 = ct{788};
t3345 = ct{789};
t3348 = ct{790};
t3351 = ct{791};
t3354 = ct{792};
t3384 = ct{793};
t3388 = ct{794};
t339 = ct{795};
t3391 = ct{796};
t3399 = ct{797};
t34 = ct{798};
t3400 = ct{799};
t3401 = ct{800};
t3404 = ct{801};
t3405 = ct{802};
t341 = ct{803};
t3414 = ct{804};
t3415 = ct{805};
t3416 = ct{806};
t342 = ct{807};
t3421 = ct{808};
t3429 = ct{809};
t343 = ct{810};
t3431 = ct{811};
t3432 = ct{812};
t3439 = ct{813};
t344 = ct{814};
t3440 = ct{815};
t3445 = ct{816};
t345 = ct{817};
t3456 = ct{818};
t346 = ct{819};
t3467 = ct{820};
t3469 = ct{821};
t347 = ct{822};
t3488 = ct{823};
t35 = ct{824};
t3500 = ct{825};
t3504 = ct{826};
t3509 = ct{827};
t3510 = ct{828};
t3516 = ct{829};
t3517 = ct{830};
t3531 = ct{831};
t354 = ct{832};
t3543 = ct{833};
t3544 = ct{834};
t3546 = ct{835};
t3557 = ct{836};
t3567 = ct{837};
t3574 = ct{838};
t3575 = ct{839};
t3578 = ct{840};
t3582 = ct{841};
t3590 = ct{842};
t3598 = ct{843};
t36 = ct{844};
t360 = ct{845};
t3601 = ct{846};
t361 = ct{847};
t3612 = ct{848};
t3617 = ct{849};
t3622 = ct{850};
t363 = ct{851};
t3630 = ct{852};
t364 = ct{853};
t3649 = ct{854};
t365 = ct{855};
t368 = ct{856};
t3683 = ct{857};
t3685 = ct{858};
t3686 = ct{859};
t3687 = ct{860};
t37 = ct{861};
t3701 = ct{862};
t3712 = ct{863};
t3721 = ct{864};
t3743 = ct{865};
t3745 = ct{866};
t3747 = ct{867};
t375 = ct{868};
t3758 = ct{869};
t3761 = ct{870};
t3770 = ct{871};
t3771 = ct{872};
t3779 = ct{873};
t3786 = ct{874};
t3792 = ct{875};
t3796 = ct{876};
t38 = ct{877};
t3813 = ct{878};
t3817 = ct{879};
t3821 = ct{880};
t3822 = ct{881};
t383 = ct{882};
t3830 = ct{883};
t384 = ct{884};
t3840 = ct{885};
t3846 = ct{886};
t3875 = ct{887};
t39 = ct{888};
t3906 = ct{889};
t3907 = ct{890};
t392 = ct{891};
t393 = ct{892};
t394 = ct{893};
t3940 = ct{894};
t3941 = ct{895};
t395 = ct{896};
t3d = ct{897};
t3dd = ct{898};
t400 = ct{899};
t401 = ct{900};
t402 = ct{901};
t4025 = ct{902};
t403 = ct{903};
t404 = ct{904};
t4059 = ct{905};
t4069 = ct{906};
t4071 = ct{907};
t4075 = ct{908};
t4076 = ct{909};
t4084 = ct{910};
t4086 = ct{911};
t4098 = ct{912};
t41 = ct{913};
t410 = ct{914};
t411 = ct{915};
t412 = ct{916};
t4126 = ct{917};
t4129 = ct{918};
t413 = ct{919};
t4133 = ct{920};
t4134 = ct{921};
t4135 = ct{922};
t4139 = ct{923};
t414 = ct{924};
t4140 = ct{925};
t4144 = ct{926};
t4146 = ct{927};
t4147 = ct{928};
t415 = ct{929};
t4150 = ct{930};
t4152 = ct{931};
t4157 = ct{932};
t4159 = ct{933};
t416 = ct{934};
t417 = ct{935};
t4172 = ct{936};
t418 = ct{937};
t419 = ct{938};
t42 = ct{939};
t420 = ct{940};
t4203 = ct{941};
t4207 = ct{942};
t4212 = ct{943};
t4230 = ct{944};
t4236 = ct{945};
t425 = ct{946};
t428 = ct{947};
t4299 = ct{948};
t43 = ct{949};
t4304 = ct{950};
t431 = ct{951};
t4325 = ct{952};
t4332 = ct{953};
t434 = ct{954};
t437 = ct{955};
t441 = ct{956};
t442 = ct{957};
t443 = ct{958};
t444 = ct{959};
t445 = ct{960};
t446 = ct{961};
t4466 = ct{962};
t453 = ct{963};
t4538 = ct{964};
t454 = ct{965};
t455 = ct{966};
t4551 = ct{967};
t4579 = ct{968};
t459 = ct{969};
t467 = ct{970};
t468 = ct{971};
t470 = ct{972};
t472 = ct{973};
t477 = ct{974};
t478 = ct{975};
t48 = ct{976};
t483 = ct{977};
t484 = ct{978};
t486 = ct{979};
t487 = ct{980};
t488 = ct{981};
t489 = ct{982};
t492 = ct{983};
t493 = ct{984};
t494 = ct{985};
t495 = ct{986};
t496 = ct{987};
t497 = ct{988};
t498 = ct{989};
t499 = ct{990};
t4d = ct{991};
t4dd = ct{992};
t50 = ct{993};
t501 = ct{994};
t502 = ct{995};
t503 = ct{996};
t507 = ct{997};
t508 = ct{998};
t51 = ct{999};
t513 = ct{1000};
t514 = ct{1001};
t515 = ct{1002};
t516 = ct{1003};
t519 = ct{1004};
t523 = ct{1005};
t524 = ct{1006};
t529 = ct{1007};
t53 = ct{1008};
t530 = ct{1009};
t531 = ct{1010};
t532 = ct{1011};
t535 = ct{1012};
t537 = ct{1013};
t542 = ct{1014};
t543 = ct{1015};
t544 = ct{1016};
t546 = ct{1017};
t547 = ct{1018};
t548 = ct{1019};
t549 = ct{1020};
t55 = ct{1021};
t550 = ct{1022};
t552 = ct{1023};
t553 = ct{1024};
t554 = ct{1025};
t56 = ct{1026};
t562 = ct{1027};
t566 = ct{1028};
t569 = ct{1029};
t57 = ct{1030};
t570 = ct{1031};
t571 = ct{1032};
t579 = ct{1033};
t58 = ct{1034};
t580 = ct{1035};
t582 = ct{1036};
t585 = ct{1037};
t587 = ct{1038};
t588 = ct{1039};
t589 = ct{1040};
t590 = ct{1041};
t591 = ct{1042};
t593 = ct{1043};
t595 = ct{1044};
t596 = ct{1045};
t598 = ct{1046};
t5d = ct{1047};
t5dd = ct{1048};
t600 = ct{1049};
t601 = ct{1050};
t602 = ct{1051};
t604 = ct{1052};
t605 = ct{1053};
t608 = ct{1054};
t609 = ct{1055};
t61 = ct{1056};
t612 = ct{1057};
t614 = ct{1058};
t615 = ct{1059};
t616 = ct{1060};
t617 = ct{1061};
t623 = ct{1062};
t624 = ct{1063};
t625 = ct{1064};
t626 = ct{1065};
t627 = ct{1066};
t63 = ct{1067};
t631 = ct{1068};
t632 = ct{1069};
t633 = ct{1070};
t634 = ct{1071};
t635 = ct{1072};
t636 = ct{1073};
t637 = ct{1074};
t639 = ct{1075};
t641 = ct{1076};
t642 = ct{1077};
t643 = ct{1078};
t644 = ct{1079};
t645 = ct{1080};
t646 = ct{1081};
t647 = ct{1082};
t648 = ct{1083};
t649 = ct{1084};
t650 = ct{1085};
t651 = ct{1086};
t652 = ct{1087};
t653 = ct{1088};
t654 = ct{1089};
t655 = ct{1090};
t656 = ct{1091};
t657 = ct{1092};
t658 = ct{1093};
t659 = ct{1094};
t660 = ct{1095};
t661 = ct{1096};
t662 = ct{1097};
t663 = ct{1098};
t664 = ct{1099};
t665 = ct{1100};
t667 = ct{1101};
t668 = ct{1102};
t669 = ct{1103};
t670 = ct{1104};
t671 = ct{1105};
t673 = ct{1106};
t674 = ct{1107};
t675 = ct{1108};
t676 = ct{1109};
t680 = ct{1110};
t681 = ct{1111};
t682 = ct{1112};
t683 = ct{1113};
t684 = ct{1114};
t685 = ct{1115};
t686 = ct{1116};
t687 = ct{1117};
t689 = ct{1118};
t69 = ct{1119};
t690 = ct{1120};
t694 = ct{1121};
t695 = ct{1122};
t696 = ct{1123};
t697 = ct{1124};
t698 = ct{1125};
t699 = ct{1126};
t6d = ct{1127};
t6dd = ct{1128};
t700 = ct{1129};
t701 = ct{1130};
t702 = ct{1131};
t703 = ct{1132};
t705 = ct{1133};
t706 = ct{1134};
t71 = ct{1135};
t711 = ct{1136};
t712 = ct{1137};
t713 = ct{1138};
t714 = ct{1139};
t720 = ct{1140};
t721 = ct{1141};
t723 = ct{1142};
t724 = ct{1143};
t725 = ct{1144};
t726 = ct{1145};
t727 = ct{1146};
t728 = ct{1147};
t729 = ct{1148};
t731 = ct{1149};
t732 = ct{1150};
t733 = ct{1151};
t735 = ct{1152};
t736 = ct{1153};
t737 = ct{1154};
t738 = ct{1155};
t739 = ct{1156};
t740 = ct{1157};
t742 = ct{1158};
t745 = ct{1159};
t746 = ct{1160};
t747 = ct{1161};
t748 = ct{1162};
t749 = ct{1163};
t75 = ct{1164};
t750 = ct{1165};
t752 = ct{1166};
t753 = ct{1167};
t754 = ct{1168};
t755 = ct{1169};
t756 = ct{1170};
t757 = ct{1171};
t759 = ct{1172};
t760 = ct{1173};
t761 = ct{1174};
t762 = ct{1175};
t763 = ct{1176};
t764 = ct{1177};
t766 = ct{1178};
t767 = ct{1179};
t768 = ct{1180};
t769 = ct{1181};
t770 = ct{1182};
t772 = ct{1183};
t774 = ct{1184};
t775 = ct{1185};
t776 = ct{1186};
t780 = ct{1187};
t781 = ct{1188};
t782 = ct{1189};
t783 = ct{1190};
t785 = ct{1191};
t786 = ct{1192};
t788 = ct{1193};
t789 = ct{1194};
t793 = ct{1195};
t799 = ct{1196};
t8 = ct{1197};
t802 = ct{1198};
t803 = ct{1199};
t804 = ct{1200};
t805 = ct{1201};
t806 = ct{1202};
t807 = ct{1203};
t808 = ct{1204};
t810 = ct{1205};
t814 = ct{1206};
t815 = ct{1207};
t817 = ct{1208};
t82 = ct{1209};
t820 = ct{1210};
t823 = ct{1211};
t824 = ct{1212};
t825 = ct{1213};
t826 = ct{1214};
t827 = ct{1215};
t828 = ct{1216};
t829 = ct{1217};
t830 = ct{1218};
t831 = ct{1219};
t832 = ct{1220};
t833 = ct{1221};
t835 = ct{1222};
t836 = ct{1223};
t838 = ct{1224};
t840 = ct{1225};
t842 = ct{1226};
t843 = ct{1227};
t844 = ct{1228};
t846 = ct{1229};
t848 = ct{1230};
t849 = ct{1231};
t850 = ct{1232};
t851 = ct{1233};
t852 = ct{1234};
t853 = ct{1235};
t854 = ct{1236};
t855 = ct{1237};
t859 = ct{1238};
t861 = ct{1239};
t865 = ct{1240};
t866 = ct{1241};
t867 = ct{1242};
t868 = ct{1243};
t869 = ct{1244};
t870 = ct{1245};
t871 = ct{1246};
t873 = ct{1247};
t874 = ct{1248};
t877 = ct{1249};
t879 = ct{1250};
t88 = ct{1251};
t880 = ct{1252};
t882 = ct{1253};
t883 = ct{1254};
t884 = ct{1255};
t885 = ct{1256};
t887 = ct{1257};
t888 = ct{1258};
t889 = ct{1259};
t890 = ct{1260};
t891 = ct{1261};
t892 = ct{1262};
t894 = ct{1263};
t895 = ct{1264};
t896 = ct{1265};
t897 = ct{1266};
t898 = ct{1267};
t899 = ct{1268};
t9 = ct{1269};
t900 = ct{1270};
t901 = ct{1271};
t902 = ct{1272};
t904 = ct{1273};
t907 = ct{1274};
t908 = ct{1275};
t909 = ct{1276};
t910 = ct{1277};
t911 = ct{1278};
t912 = ct{1279};
t913 = ct{1280};
t915 = ct{1281};
t917 = ct{1282};
t919 = ct{1283};
t921 = ct{1284};
t922 = ct{1285};
t923 = ct{1286};
t927 = ct{1287};
t928 = ct{1288};
t931 = ct{1289};
t932 = ct{1290};
t937 = ct{1291};
t938 = ct{1292};
t943 = ct{1293};
t944 = ct{1294};
t945 = ct{1295};
t952 = ct{1296};
t954 = ct{1297};
t955 = ct{1298};
t956 = ct{1299};
t957 = ct{1300};
t959 = ct{1301};
t960 = ct{1302};
t961 = ct{1303};
t962 = ct{1304};
t963 = ct{1305};
t964 = ct{1306};
t965 = ct{1307};
t966 = ct{1308};
t968 = ct{1309};
t969 = ct{1310};
t970 = ct{1311};
t971 = ct{1312};
t972 = ct{1313};
t973 = ct{1314};
t974 = ct{1315};
t975 = ct{1316};
t978 = ct{1317};
t979 = ct{1318};
t980 = ct{1319};
t981 = ct{1320};
t982 = ct{1321};
t983 = ct{1322};
t984 = ct{1323};
t985 = ct{1324};
t986 = ct{1325};
t987 = ct{1326};
t989 = ct{1327};
t992 = ct{1328};
t993 = ct{1329};
t994 = ct{1330};
t997 = ct{1331};
t998 = ct{1332};
t999 = ct{1333};
t1396 = -t627.*(t101-t401);
t1402 = t341.*t898;
t1407 = t341.*t908;
t1409 = -t1369;
t1411 = t1376./2.0;
t1421 = t1369./2.0;
t1422 = t1370./2.0;
t1423 = t1371./2.0;
t1436 = -t1401;
t1437 = t402.*t898;
t1446 = t402.*t908;
t1451 = t627.*(t101-t401).*(-1.0./2.0);
t1456 = t1400./2.0;
t1459 = t1403./2.0;
t1461 = t1424.*t1d;
t1472 = -t1434;
t1474 = -t1439;
t1475 = -t1440;
t1478 = t1425./2.0;
t1483 = t1434./2.0;
t1486 = t1440./2.0;
t1503 = t694+t695;
t1507 = t1471.*-2.0;
t1508 = t8.*t1454;
t1509 = t14.*t1452;
t1524 = t255.*t1187;
t1525 = t37.*t1419;
t1528 = t37.*t1420;
t1529 = t39.*t1419;
t1533 = t39.*t1420;
t1538 = -t1505;
t1543 = t1505./2.0;
t1546 = -t1522;
t1554 = t330.*t1187;
t1580 = t341.*t1187;
t1586 = t115.*t1420;
t1587 = t609.*t908;
t1588 = t255.*t1296;
t1589 = t330.*t1254;
t1590 = t1537./2.0;
t1594 = -t1551;
t1599 = t8.*t39.*t1452;
t1606 = t18.*t61.*t1420;
t1607 = t14.*t39.*t1454;
t1610 = t18.*t63.*t1420;
t1615 = t112.*t1419;
t1616 = t609.*t898;
t1625 = t402.*t1187;
t1632 = -t1585;
t1633 = t641.*t898;
t1634 = -t908.*(t100-t364);
t1635 = t641.*t908;
t1644 = t1584./2.0;
t1645 = t155.*t1419;
t1646 = -t898.*(t100-t364);
t1655 = t18.*t37.*t1502;
t1657 = t12.*t39.*t1502;
t1661 = t18.*t39.*t1502;
t1668 = t174.*t1420;
t1670 = -t1629;
t1672 = -t1631;
t1675 = -t898.*(t101-t401);
t1676 = -t908.*(t101-t401);
t1683 = t1627./2.0;
t1684 = t1629./2.0;
t1687 = t767+t768;
t1688 = t35.*t39.*t1502;
t1690 = t18.*t61.*t1502;
t1692 = t769+t770;
t1693 = t38.*t39.*t1502;
t1695 = t18.*t63.*t1502;
t1708 = -t1678;
t1715 = -t1679;
t1724 = t1667./2.0;
t1726 = t14.*t1659;
t1727 = t18.*t39.*t1553;
t1739 = t255.*t1419;
t1742 = t786+t803;
t1743 = t256.*t1420;
t1749 = t14.*t1703;
t1752 = t14.*t1705;
t1756 = -t1705;
t1761 = t256.*t1419.*2.0;
t1762 = t255.*t1420.*2.0;
t1774 = t8.*t1701;
t1776 = t766+t877;
t1777 = t363.*t1420;
t1778 = t339.*t1419;
t1779 = t13.*t255.*t1420;
t1781 = t19.*t255.*t1420;
t1783 = t330.*t1419;
t1784 = t329.*t1420;
t1786 = t753+t867;
t1792 = t1734.*t1d;
t1793 = t329.*t1419.*2.0;
t1794 = t609.*t1187;
t1795 = t330.*t1420.*2.0;
t1797 = t341.*t1419;
t1799 = t341.*t1420;
t1800 = t342.*t1420;
t1805 = t428.*t1419;
t1806 = t13.*t330.*t1420;
t1808 = t400.*t1420;
t1809 = t19.*t330.*t1420;
t1814 = t1775./2.0;
t1815 = t8.*t37.*t1659;
t1816 = t8.*t39.*t1659;
t1819 = t255.*t1502;
t1820 = t256.*t1502;
t1823 = -t1187.*(t100-t364);
t1825 = t641.*t1187;
t1826 = t14.*t1780;
t1827 = t402.*t1419;
t1829 = t402.*t1420;
t1830 = t403.*t1420;
t1832 = t14.*t37.*t1701;
t1835 = t14.*t39.*t1701;
t1844 = t35.*t39.*t1659;
t1855 = t329.*t1502;
t1856 = t330.*t1502;
t1861 = t468.*t1419;
t1862 = t453.*t1420;
t1865 = t1187.*(t100-t364);
t1867 = t472.*t1420;
t1869 = -t1187.*(t101-t401);
t1870 = t477.*t1420;
t1871 = t459.*t1420;
t1876 = t1831.*t2d;
t1877 = t1831.*t3d;
t1878 = t1831.*t4d;
t1880 = t1817.*t2d;
t1881 = t1817.*t3d;
t1882 = t1817.*t4d;
t1893 = t341.*t1502;
t1895 = t342.*t1502;
t1897 = -t1839;
t1898 = t255.*t1553;
t1909 = t38.*t39.*t1701;
t1919 = t508.*t1419;
t1920 = t507.*t1420;
t1921 = t513.*t1419;
t1922 = t499.*t1420;
t1924 = t38.*t437.*t1420;
t1928 = t514.*t1420;
t1931 = t524.*t1420;
t1932 = t502.*t1420;
t1935 = t884+t971;
t1938 = t1846./2.0;
t1947 = t402.*t1502;
t1949 = t403.*t1502;
t1953 = t330.*t1553;
t1959 = -t1905;
t1966 = t35.*t484.*t1420;
t1972 = -t1925;
t1983 = t341.*t1553;
t1985 = t1905./2.0;
t1990 = t453.*t1502;
t1996 = t459.*t1502;
t2023 = t402.*t1553;
t2027 = t609.*t1419;
t2028 = t499.*t1502;
t2030 = t609.*t1420;
t2032 = t502.*t1502;
t2050 = t829+t1188;
t2058 = t546.*t1502;
t2059 = t330.*t1659;
t2060 = t548.*t1502;
t2061 = t255.*t1701;
t2064 = -t1419.*(t100-t364);
t2066 = -t1420.*(t100-t364);
t2067 = t641.*t1419;
t2068 = t641.*t1420;
t2077 = t998+t1028;
t2078 = -t2052;
t2079 = t587.*t1502;
t2080 = t588.*t1502;
t2082 = t591.*t1502;
t2084 = t913+t1156;
t2091 = -t1419.*(t101-t401);
t2092 = t1420.*(t100-t364);
t2094 = -t1420.*(t101-t401);
t2096 = t2049./2.0;
t2097 = t2052./2.0;
t2103 = t14.*t2046;
t2121 = t609.*t1502.*2.0;
t2134 = -t8.*(t844-t1156);
t2137 = t669.*t1502;
t2138 = -t1502.*(t100-t364);
t2139 = t641.*t1502;
t2153 = t609.*t1553;
t2161 = t8.*t2116;
t2171 = t535+t732+t757;
t2172 = t2127./2.0;
t2177 = t2133./2.0;
t2180 = t8.*t39.*t2046;
t2181 = t8.*(t844-t1156).*(-1.0./2.0);
t2185 = t1502.*(t101-t401).*-2.0;
t2192 = -t1553.*(t100-t364);
t2193 = t641.*t1553;
t2198 = t494+t764+t802;
t2199 = t724.*t1502;
t2200 = -t14.*t39.*(t844-t1156);
t2202 = t1502.*(t101-t401).*2.0;
t2204 = t579+t728+t763;
t2211 = t739.*t1502;
t2212 = t726.*t1502;
t2216 = t1553.*(t100-t364);
t2219 = -t1553.*(t101-t401);
t2221 = t37.*t2120;
t2222 = t263+t927+t966;
t2225 = t268+t923+t973;
t2228 = t37.*t2124;
t2235 = t14.*t39.*t2116;
t2240 = t14.*t2189;
t2241 = t14.*t2190;
t2243 = t780.*t1502;
t2244 = t14.*t39.*(t844-t1156).*(-1.0./2.0);
t2245 = -t2210;
t2247 = t783.*t1502;
t2256 = t8.*t39.*t2120;
t2257 = t12.*t39.*t2120;
t2259 = t1107+t1223;
t2260 = t14.*t39.*t2120;
t2261 = t18.*t39.*t2120;
t2262 = t8.*t39.*t2124;
t2263 = t12.*t39.*t2124;
t2264 = t14.*t39.*t2124;
t2265 = t18.*t39.*t2124;
t2280 = t537+t810+t814;
t2283 = t2227./2.0;
t2292 = t1180+t1263;
t2294 = t807.*t1502;
t2299 = t815.*t1502;
t2323 = -t8.*(t1155+t341.*(t101-t401));
t2333 = t866.*t1502;
t2335 = t871.*t1502;
t2339 = t8.*t37.*t2189;
t2343 = t8.*t39.*t2189;
t2352 = t14.*t37.*t1502.*(t101-t401).*(-1.0./2.0);
t2363 = t937.*t1502;
t2365 = t330.*t2046;
t2366 = t35.*t39.*t2189;
t2368 = t8.*(t1155+t341.*(t101-t401)).*(-1.0./2.0);
t2370 = -t255.*(t844-t1156);
t2379 = t18.*t37.*t2233;
t2380 = t12.*t39.*t2233;
t2382 = t18.*t39.*t2233;
t2385 = (t8.*(t1155+t341.*(t101-t401)))./2.0;
t2389 = t969.*t1502;
t2390 = t1253+t1296;
t2391 = t1254+t1295;
t2402 = t255.*t2116;
t2403 = -t14.*t37.*(t1155+t341.*(t101-t401));
t2404 = -t14.*t39.*(t1155+t341.*(t101-t401));
t2405 = t2371.*t3d;
t2406 = t2372.*t1d;
t2407 = t2372.*t3d;
t2408 = t255.*t2120;
t2409 = t256.*t2120;
t2410 = t35.*t39.*t2233;
t2412 = t18.*t61.*t2233;
t2413 = t38.*t39.*t2233;
t2414 = t18.*t63.*t2233;
t2416 = t255.*t2124;
t2417 = t256.*t2124;
t2423 = -t2383;
t2424 = t255.*(t844-t1156).*(-1.0./2.0);
t2426 = t1015.*t1502;
t2428 = t1017.*t1502;
t2436 = -t38.*t39.*(t1155+t341.*(t101-t401));
t2439 = t14.*t39.*(t1155+t341.*(t101-t401));
t2440 = t329.*t2120;
t2441 = t330.*t2120;
t2447 = t329.*t2124;
t2448 = t330.*t2124;
t2457 = -t2425;
t2461 = t14.*t37.*(t1155+t341.*(t101-t401)).*(-1.0./2.0);
t2462 = t1069.*t1502;
t2471 = t341.*t2124;
t2475 = t38.*t39.*(t1155+t341.*(t101-t401));
t2477 = (t14.*t37.*(t1155+t341.*(t101-t401)))./2.0;
t2480 = t1291+t1342;
t2481 = t1293+t1340;
t2487 = t1137.*t1502;
t2497 = t402.*t2124;
t2515 = t330.*t2189;
t2516 = t276+t375+t383+t674+t676;
t2518 = t8.*t2469;
t2520 = t1193.*t1502;
t2523 = t255.*t2233;
t2524 = t256.*t2233;
t2547 = -t255.*(t1155+t341.*(t101-t401));
t2553 = t329.*t2233;
t2554 = t330.*t2233;
t2571 = -t2539;
t2578 = t591+t1015+t1069;
t2579 = t593+t1021+t1065;
t2580 = t341.*t2233;
t2581 = t342.*t2233;
t2594 = -t2576;
t2599 = t255.*(t1155+t341.*(t101-t401)).*(-1.0./2.0);
t2608 = -t2593;
t2611 = t403.*t2233;
t2623 = t402.*t2233.*2.0;
t2628 = t453.*t2233;
t2631 = t459.*t2233;
t2635 = t609.*t2124;
t2649 = t499.*t2233;
t2650 = t502.*t2233;
t2651 = -t2124.*(t100-t364);
t2653 = t641.*t2124;
t2654 = t160+t2469;
t2664 = t548.*t2233;
t2674 = -t2124.*(t101-t401);
t2678 = -t18.*t37.*(t544-t1021+t330.*(t100-t364));
t2680 = -t12.*t39.*(t544-t1021+t330.*(t100-t364));
t2682 = -t18.*t39.*(t544-t1021+t330.*(t100-t364));
t2686 = t14.*t2658;
t2688 = t585+t624+t737+t756;
t2690 = t587.*t2233;
t2694 = t8.*t2655;
t2695 = t2124.*(t101-t401);
t2698 = -t35.*t39.*(t544-t1021+t330.*(t100-t364));
t2700 = -t18.*t61.*(t544-t1021+t330.*(t100-t364));
t2702 = -t38.*t39.*(t544-t1021+t330.*(t100-t364));
t2704 = -t18.*t63.*(t544-t1021+t330.*(t100-t364));
t2705 = t18.*t39.*(t544-t1021+t330.*(t100-t364));
t2711 = t18.*t37.*(t544-t1021+t330.*(t100-t364)).*(-1.0./2.0);
t2715 = t609.*t2233.*2.0;
t2723 = t35.*t39.*(t544-t1021+t330.*(t100-t364));
t2724 = t18.*t61.*(t544-t1021+t330.*(t100-t364));
t2726 = -t2233.*(t100-t364);
t2727 = t641.*t2233;
t2729 = -t2706;
t2731 = t228+t360+t361+t1847;
t2736 = -t2714;
t2737 = t1490+t1530;
t2739 = t669.*t2233;
t2741 = t625+t656+t727+t762;
t2750 = t2233.*(t100-t364);
t2753 = t627+t661+t700+t868;
t2756 = -t2747;
t2760 = -t2d.*(-t915+t978+(t8.*(t249-t483))./2.0);
t2761 = -t3d.*(-t915+t978+(t8.*(t249-t483))./2.0);
t2762 = -t4d.*(-t915+t978+(t8.*(t249-t483))./2.0);
t2764 = -t2d.*(-t917+t979+(t14.*(t248-t484))./2.0);
t2765 = -t3d.*(-t917+t979+(t14.*(t248-t484))./2.0);
t2766 = -t4d.*(-t917+t979+(t14.*(t248-t484))./2.0);
t2767 = t626+t657+t750+t761;
t2768 = t2233.*(t101-t401).*-2.0;
t2770 = -t2755;
t2781 = -t2772;
t2783 = -t255.*(t544-t1021+t330.*(t100-t364));
t2785 = -t256.*(t544-t1021+t330.*(t100-t364));
t2794 = t724.*t2233;
t2807 = t739.*t2233;
t2822 = -t329.*(t544-t1021+t330.*(t100-t364));
t2824 = -t330.*(t544-t1021+t330.*(t100-t364));
t2826 = t256.*(t544-t1021+t330.*(t100-t364));
t2838 = -t342.*(t544-t1021+t330.*(t100-t364));
t2841 = t780.*t2233;
t2843 = t783.*t2233;
t2860 = t329.*(t544-t1021+t330.*(t100-t364));
t2863 = t341.*(t544-t1021+t330.*(t100-t364)).*-2.0;
t2868 = t807.*t2233;
t2877 = -t402.*(t544-t1021+t330.*(t100-t364));
t2879 = -t403.*(t544-t1021+t330.*(t100-t364));
t2894 = t342.*(t544-t1021+t330.*(t100-t364)).*(-1.0./2.0);
t2901 = t866.*t2233;
t2912 = -t453.*(t544-t1021+t330.*(t100-t364));
t2914 = -t459.*(t544-t1021+t330.*(t100-t364));
t2916 = t402.*(t544-t1021+t330.*(t100-t364));
t2925 = t14.*t37.*t2233.*(t101-t401).*(-1.0./2.0);
t2934 = t403.*(t544-t1021+t330.*(t100-t364)).*(-1.0./2.0);
t2936 = -t496.*(t544-t1021+t330.*(t100-t364));
t2941 = t2927.*(-1.0./2.0);
t2943 = -t499.*(t544-t1021+t330.*(t100-t364));
t2945 = -t502.*(t544-t1021+t330.*(t100-t364));
t2946 = t1000+t1112+t1115;
t2947 = t1001+t1113+t1116;
t2951 = t39.*t219.*t2655;
t2952 = t36.*t39.*t2655.*2.8925e-2;
t2954 = -t2938;
t2955 = t937.*t2233.*(-1.0./2.0);
t2959 = t2927./2.0;
t2965 = -t542.*(t544-t1021+t330.*(t100-t364));
t2966 = t36.*t39.*t2655.*(-5.785e-2);
t2970 = t496.*(t544-t1021+t330.*(t100-t364));
t2971 = (t937.*t2233)./2.0;
t2978 = t499.*(t544-t1021+t330.*(t100-t364));
t2979 = t502.*(t544-t1021+t330.*(t100-t364));
t2992 = t542.*(t544-t1021+t330.*(t100-t364));
t3008 = -t609.*(t544-t1021+t330.*(t100-t364));
t3023 = t550+t2655;
t3030 = (t100-t364).*(t544-t1021+t330.*(t100-t364)).*2.0;
t3031 = t641.*(t544-t1021+t330.*(t100-t364)).*-2.0;
t3033 = t571+t2658;
t3038 = -t694.*(t544-t1021+t330.*(t100-t364));
t3039 = t14.*(t100-t364).*(t544-t1021+t330.*(t100-t364));
t3042 = (t101-t401).*(t544-t1021+t330.*(t100-t364));
t3062 = t781+t804+t838+t840;
t3063 = t754+t785+t806+t894;
t3066 = -t3045;
t3071 = t14.*t3034;
t3079 = t3045./2.0;
t3082 = t1753+t1772;
t3087 = t3078.*(-1.0./2.0);
t3099 = t8.*t37.*(t100-t364).*(t544-t1021+t330.*(t100-t364));
t3101 = t3078./2.0;
t3102 = -t14.*(t752-t781-t838+t18.*t63.*(t100-t364));
t3103 = -t8.*(t729-t785-t806+t18.*t61.*(t101-t401));
t3114 = t957+t2473;
t3123 = t892.*(t544-t1021+t330.*(t100-t364));
t3125 = t782.*(t544-t1021+t330.*(t100-t364));
t3127 = -t805.*(t544-t1021+t330.*(t100-t364));
t3132 = t697+t731+t981+t999;
t3145 = t755.*(t544-t1021+t330.*(t100-t364)).*(-1.0./2.0);
t3147 = t14.*(t752-t781-t838+t18.*t63.*(t100-t364)).*(-1.0./2.0);
t3149 = t8.*(t729-t785-t806+t18.*t61.*(t101-t401)).*(-1.0./2.0);
t3154 = t14.*t687.*t2655;
t3163 = t805.*(t544-t1021+t330.*(t100-t364));
t3166 = (t755.*(t544-t1021+t330.*(t100-t364)))./2.0;
t3168 = (t14.*(t752-t781-t838+t18.*t63.*(t100-t364)))./2.0;
t3169 = (t8.*(t729-t785-t806+t18.*t61.*(t101-t401)))./2.0;
t3175 = t1497+t2149;
t3176 = t1468+t2179;
t3177 = t14.*t703.*t2655;
t3207 = t1117+t1305+t1351;
t3237 = t3185./2.0;
t3251 = t1703+t2039;
t3298 = t3260./2.0;
t3335 = -t3318;
t3340 = t3318./2.0;
t3341 = t1176+t1442+t1443;
t3342 = t1177+t1441+t1444;
t3343 = t14.*t1036.*t2655;
t3347 = -t3331;
t3349 = t14.*t1055.*t2655;
t3355 = t3331./2.0;
t3360 = t8.*t1082.*t2658;
t3368 = t191+t417+t445+t588+t1017+t1193;
t3381 = t3351./2.0;
t3383 = t2011+t2025;
t3407 = -t2270.*(t745-t747);
t3433 = t901+t902+t1075+t1151;
t3443 = t2270.*(t745-t747).*(-1.0./2.0);
t3452 = t3414./2.0;
t3457 = -t3439;
t3458 = t3416./2.0;
t3459 = -t3440;
t3460 = t3431.*t4d;
t3461 = t3432.*t1d;
t3466 = t14.*t1302.*t2655;
t3468 = (t8.*t1807.*t2169)./2.0;
t3498 = (t14.*t1321.*t2655)./2.0;
t3513 = (t1399.*t2655)./2.0;
t3520 = t495+t548+t683+t686+t783+t807;
t3523 = (t1874.*t2270)./2.0;
t3556 = -t18.*t39.*(-t496-t547+t615+t623+t755+t8.*t37.*(t100-t364));
t3560 = t3546.*(-1.0./2.0);
t3568 = t3546./2.0;
t3579 = t18.*t39.*(-t496-t547+t615+t623+t755+t8.*t37.*(t100-t364));
t3580 = t799.*t3083;
t3584 = t3567.*(-1.0./2.0);
t3606 = t3567./2.0;
t3628 = (t8.*t2113.*t2169)./2.0;
t3674 = -t255.*(-t496-t547+t615+t623+t755+t8.*t37.*(t100-t364));
t3678 = (t721.*t3230)./2.0;
t3697 = -t330.*(-t496-t547+t615+t623+t755+t8.*t37.*(t100-t364));
t3704 = -t341.*(-t496-t547+t615+t623+t755+t8.*t37.*(t100-t364));
t3716 = -t3701;
t3724 = -t402.*(-t496-t547+t615+t623+t755+t8.*t37.*(t100-t364));
t3734 = t1141+t1195+t1213+t1262;
t3738 = -t3712;
t3741 = (t8.*t2169.*t2279)./2.0;
t3744 = t341.*(-t496-t547+t615+t623+t755+t8.*t37.*(t100-t364)).*(-1.0./2.0);
t3750 = t2234+t2302;
t3751 = t3712./2.0;
t3768 = t402.*(-t496-t547+t615+t623+t755+t8.*t37.*(t100-t364)).*(-1.0./2.0);
t3769 = t8.*t1807.*t2658;
t3785 = t8.*t1818.*t2658;
t3835 = -t609.*(-t496-t547+t615+t623+t755+t8.*t37.*(t100-t364));
t3843 = t8.*t1082.*t3230;
t3852 = (t100-t364).*(-t496-t547+t615+t623+t755+t8.*t37.*(t100-t364));
t3853 = t609.*(-t496-t547+t615+t623+t755+t8.*t37.*(t100-t364));
t3854 = -t641.*(-t496-t547+t615+t623+t755+t8.*t37.*(t100-t364));
t3857 = t3846.*(-1.0./2.0);
t3871 = t3846./2.0;
t3872 = t3840./2.0;
t3877 = (t101-t401).*(-t496-t547+t615+t623+t755+t8.*t37.*(t100-t364));
t3878 = t641.*(-t496-t547+t615+t623+t755+t8.*t37.*(t100-t364));
t3895 = t3875.*(-1.0./2.0);
t3897 = -t14.*(t1070.*(t100-t364)+t330.*(t544-t1021+t330.*(t100-t364)));
t3903 = t3875./2.0;
t3918 = t310+t608+t919+t965+t970+t1086;
t3920 = t885+t921+t1427+t1757;
t3922 = t304+t601+t922+t959+t963+t1087;
t3923 = t1297.*t3230;
t3939 = t14.*(t1070.*(t100-t364)+t330.*(t544-t1021+t330.*(t100-t364))).*(-1.0./2.0);
t3943 = t2270.*t2529;
